simulink model "simulator_prototype_v2"  (R2021b)
(part 5 of 12)

tau_c = ft_4({dq1,dq2,dq3,dq4,dq5,dq6,t10,t100,t1000,t1001,t1002,t1003,t1006,t1009,t101,t1011,t1014,t1015,t1017,t1018,t1019,t1020,t1021,t1023,t1024,t1025,t1028,t1029,t103,t1030,t1031,t1032,t1035,t1038,t1039,t104,t1041,t1042,t1044,t1045,t1046,t1048,t1049,t1050,t1051,t1052,t1055,t1056,t1057,t1058,t1059,t106,t1061,t1062,t1065,t1066,t1067,t107,t1070,t1071,t1072,t1073,t1074,t1075,t1076,t108,t1080,t1083,t1084,t1089,t109,t1090,t1091,t1092,t1094,t1095,t1098,t1099,t11,t110,t1100,t1102,t1103,t1104,t1105,t1106,t1107,t1108,t1109,t111,t1110,t1111,t1112,t1113,t1114,t1115,t1116,t1117,t1118,t1119,t1120,t1121,t1122,t1123,t1124,t1125,t1126,t1129,t113,t1132,t1135,t1137,t1138,t1139,t114,t1140,t1141,t1142,t1144,t1145,t1146,t1147,t1148,t1149,t115,t1150,t1154,t1158,t1159,t1162,t1165,t1166,t1167,t1170,t1174,t1176,t1177,t1178,t1179,t118,t1180,t1184,t1185,t1186,t1187,t1188,t1189,t1190,t1192,t1193,t1194,t1195,t1196,t1197,t1198,t1199,t12,t120,t1202,t1203,t1204,t1205,t1206,t1207,t1208,t1209,t121,t1210,t1212,t1213,t1214,t1217,t1218,t1219,t122,t1220,t1221,t1222,t1223,t1224,t1229,t123,t1230,t1232,t1234,t1235,t1236,t1237,t1238,t124,t1241,t1242,t1245,t1246,t1247,t1248,t125,t1251,t1252,t1253,t1254,t1255,t1256,t1259,t126,t1260,t1261,t1262,t1263,t1264,t1265,t1266,t1267,t1268,t127,t1270,t1271,t1272,t1277,t1278,t128,t1280,t1281,t1285,t1286,t1287,t1288,t1289,t1290,t1291,t1292,t1294,t1295,t1296,t1297,t1298,t1299,t13,t130,t1300,t1301,t1302,t1303,t1304,t1305,t1307,t1310,t1311,t1316,t1317,t1319,t132,t1320,t1322,t1323,t1324,t1325,t1326,t1328,t133,t1330,t1331,t1332,t1334,t1335,t1336,t1337,t1338,t134,t1342,t1343,t1344,t1345,t1348,t1349,t1350,t1351,t1352,t1353,t1354,t136,t1360,t1364,t1366,t1367,t1368,t1369,t1370,t1371,t1372,t1374,t1375,t1376,t1377,t1378,t1379,t138,t1380,t1383,t1385,t1386,t1387,t1388,t1389,t139,t1392,t1393,t1394,t1395,t1396,t1397,t1398,t1399,t14,t140,t1401,t1402,t1403,t1404,t1405,t1406,t1407,t1408,t1409,t1410,t1411,t1412,t1413,t1414,t1415,t1416,t1417,t1418,t1419,t1420,t1421,t1422,t1423,t1424,t1425,t1426,t1427,t1428,t1429,t1430,t1431,t1432,t1433,t1434,t1435,t1436,t1437,t1439,t144,t1440,t1441,t1443,t1444,t1445,t1446,t1447,t1448,t145,t1451,t1453,t1454,t1456,t1457,t1458,t1459,t1460,t1461,t1462,t1463,t1464,t1468,t1469,t1471,t1474,t1477,t1478,t1479,t148,t1480,t1481,t1482,t1483,t1484,t1485,t1486,t1487,t1488,t1489,t149,t1490,t1491,t1492,t1493,t1494,t1495,t1497,t1498,t1499,t15,t150,t1500,t1501,t1503,t1504,t1505,t1506,t1507,t1509,t151,t1510,t1512,t1513,t1514,t1515,t1516,t1517,t1518,t1519,t152,t1520,t1522,t1523,t1525,t1526,t1527,t1528,t1529,t153,t1530,t1531,t1532,t1533,t1535,t1536,t1537,t1538,t1539,t1541,t1542,t1543,t1544,t1545,t1546,t1547,t1549,t1550,t1551,t1552,t1554,t1555,t1556,t1558,t1559,t156,t1560,t1565,t1567,t1568,t1569,t157,t1570,t1571,t1572,t1574,t1575,t1576,t1577,t1578,t1579,t158,t1581,t1582,t1583,t1584,t1585,t1586,t1587,t1588,t1591,t1592,t1593,t1594,t1595,t1596,t1599,t16,t160,t1600,t1601,t1602,t1604,t1605,t1606,t1607,t1608,t1609,t161,t1613,t1614,t1615,t1616,t1618,t1619,t162,t1620,t1621,t1622,t1623,t1624,t1625,t1626,t1627,t1628,t1629,t1631,t1633,t1634,t1635,t1636,t1637,t1638,t1639,t1640,t1641,t1642,t1643,t1644,t1645,t1646,t1648,t1649,t165,t1650,t1651,t1652,t1653,t1654,t1655,t1656,t1657,t1658,t166,t1660,t167,t168,t1686,t1688,t1689,t1690,t1695,t17,t170,t1700,t1701,t1702,t171,t172,t173,t174,t175,t1750,t176,t1765,t177,t178,t1780,t1782,t1795,t1796,t1797,t1798,t18,t180,t1807,t181,t1817,t182,t185,t186,t1865,t1868,t1870,t1871,t1872,t1873,t1874,t1875,t1876,t1877,t1879,t188,t1880,t1881,t1882,t1883,t1884,t1886,t1887,t1889,t189,t1890,t1891,t1894,t1895,t1897,t1898,t1899,t19,t190,t1901,t1902,t1903,t1904,t1907,t1909,t191,t1914,t1915,t1916,t1917,t1919,t192,t1920,t1922,t1923,t1924,t1925,t1926,t1927,t1928,t1929,t1930,t1931,t1936,t1937,t1940,t1941,t1942,t1943,t1947,t1948,t1949,t195,t1950,t1951,t1952,t1953,t1956,t1958,t1959,t196,t1960,t1961,t1965,t1966,t1967,t1968,t197,t1970,t1971,t1975,t1977,t198,t1982,t1991,t1997,t20,t201,t2017,t202,t2021,t2022,t2024,t2025,t2027,t2028,t2029,t203,t2030,t2032,t2034,t2035,t2038,t2039,t204,t2043,t2044,t2045,t2049,t205,t2050,t2051,t2052,t2054,t2055,t2056,t2057,t2058,t2059,t2061,t2062,t2063,t2069,t207,t2075,t2077,t208,t2080,t2081,t2082,t2083,t2084,t2085,t2086,t2087,t2088,t2089,t209,t2090,t2091,t2092,t2093,t2096,t2097,t2098,t2099,t21,t210,t2100,t2101,t2102,t2103,t2104,t2105,t211,t2117,t2118,t2119,t212,t2120,t2121,t2122,t2123,t2124,t2131,t2138,t2139,t2140,t2147,t2149,t2150,t2151,t2152,t2153,t2154,t2155,t2156,t2157,t2158,t2159,t216,t217,t218,t219,t22,t221,t223,t225,t226,t227,t229,t2294,t2296,t2299,t230,t2300,t2302,t2303,t2305,t2306,t2308,t2309,t231,t2310,t2313,t2314,t2315,t2316,t2317,t2318,t2319,t2322,t2323,t2324,t2325,t2326,t2327,t2328,t2329,t233,t2330,t2331,t2332,t2334,t2339,t2340,t2345,t2346,t2348,t2349,t2352,t2353,t2354,t2357,t2358,t2359,t236,t2360,t2361,t2362,t2364,t2365,t2366,t2367,t237,t2374,t2378,t238,t2382,t2383,t239,t2391,t2392,t2393,t24,t240,t2402,t2404,t2405,t2406,t2407,t2409,t241,t2411,t2415,t2416,t2417,t2418,t242,t2420,t2426,t2427,t2428,t2429,t243,t2430,t2431,t2432,t2433,t2434,t2435,t2436,t2437,t2438,t2439,t2440,t2441,t2442,t2443,t2444,t2446,t2447,t2448,t2449,t245,t2451,t2452,t2453,t2454,t2455,t2456,t2457,t2459,t246,t2460,t2461,t2463,t2466,t2467,t2469,t247,t2471,t2475,t2482,t2483,t2484,t2485,t2486,t2487,t2488,t2491,t2495,t2498,t2499,t25,t2505,t251,t2512,t2513,t2515,t2529,t2541,t2544,t2546,t2551,t2560,t2567,t2568,t257,t2573,t2577,t2579,t2581,t2586,t2587,t2588,t259,t2593,t2594,t2595,t2596,t2597,t2599,t26,t260,t2600,t2601,t2603,t2605,t2606,t2607,t2608,t2609,t261,t2610,t2611,t2612,t2613,t2614,t2616,t2617,t2618,t2619,t262,t2620,t2621,t2622,t2623,t2624,t2625,t2626,t2627,t2628,t263,t2631,t2632,t2633,t2635,t2639,t264,t2640,t2641,t2642,t2643,t2645,t2646,t2647,t265,t2651,t2652,t2653,t2656,t266,t267,t268,t269,t27,t270,t271,t272,t2723,t2724,t2725,t2726,t2727,t2728,t2729,t273,t2730,t2735,t2736,t274,t2745,t2748,t2749,t275,t2750,t276,t2773,t2774,t2775,t2777,t2778,t2779,t2780,t2781,t2782,t2783,t2785,t2786,t2787,t2788,t279,t2797,t28,t280,t2800,t282,t283,t285,t2857,t2858,t2859,t286,t2860,t2865,t2867,t2868,t2872,t2879,t2883,t2884,t2886,t2887,t289,t2890,t2891,t2892,t2894,t2895,t2896,t2898,t2899,t29,t2900,t2901,t2903,t2905,t2906,t2907,t2908,t291,t2915,t2917,t2918,t2919,t292,t293,t294,t295,t2959,t296,t2960,t2965,t2966,t2967,t2968,t297,t298,t299,t30,t301,t303,t305,t306,t308,t309,t31,t310,t311,t312,t313,t314,t315,t316,t318,t319,t32,t320,t321,t322,t323,t325,t326,t328,t329,t33,t330,t331,t332,t333,t335,t336,t337,t338,t339,t34,t341,t343,t346,t348,t35,t350,t351,t352,t354,t355,t356,t358,t359,t36,t360,t361,t362,t363,t364,t365,t366,t368,t369,t370,t371,t372,t373,t377,t378,t38,t380,t381,t382,t385,t386,t387,t388,t389,t39,t390,t391,t392,t393,t396,t403,t404,t406,t407,t408,t410,t411,t412,t413,t414,t415,t419,t42,t420,t421,t422,t424,t425,t426,t427,t428,t429,t43,t430,t431,t432,t433,t434,t435,t437,t438,t439,t440,t444,t445,t446,t448,t451,t452,t455,t456,t457,t458,t459,t46,t461,t463,t464,t465,t466,t467,t468,t469,t47,t471,t472,t473,t474,t476,t477,t478,t479,t480,t483,t485,t486,t488,t489,t49,t490,t491,t493,t494,t495,t496,t497,t498,t50,t503,t504,t506,t507,t508,t509,t51,t510,t511,t512,t513,t514,t515,t516,t517,t518,t519,t52,t520,t521,t522,t523,t524,t525,t526,t527,t528,t53,t530,t531,t532,t533,t536,t537,t538,t539,t54,t540,t542,t543,t544,t545,t546,t547,t548,t550,t551,t552,t553,t554,t555,t556,t557,t559,t56,t560,t561,t562,t563,t565,t566,t568,t569,t570,t571,t572,t573,t574,t575,t576,t577,t578,t58,t580,t582,t583,t584,t585,t589,t59,t590,t591,t592,t595,t597,t599,t60,t600,t601,t605,t606,t607,t608,t609,t610,t611,t612,t614,t615,t616,t618,t619,t620,t621,t622,t623,t624,t625,t627,t628,t629,t63,t631,t634,t635,t636,t638,t64,t640,t641,t642,t643,t645,t646,t648,t649,t65,t650,t651,t652,t654,t655,t656,t657,t658,t659,t660,t662,t663,t664,t665,t666,t667,t668,t669,t67,t670,t672,t673,t674,t675,t676,t677,t678,t679,t68,t681,t682,t683,t684,t685,t686,t687,t689,t69,t691,t692,t693,t694,t696,t698,t70,t701,t702,t704,t705,t707,t708,t71,t710,t711,t712,t713,t714,t715,t716,t717,t718,t719,t720,t721,t722,t723,t724,t725,t726,t728,t73,t733,t735,t736,t738,t739,t740,t741,t742,t743,t744,t745,t746,t747,t749,t75,t750,t751,t755,t756,t757,t758,t759,t76,t762,t763,t764,t765,t766,t767,t768,t77,t770,t771,t772,t773,t774,t775,t776,t777,t778,t78,t781,t782,t783,t784,t785,t786,t787,t789,t79,t790,t791,t792,t793,t794,t796,t797,t798,t799,t8,t80,t800,t801,t802,t806,t807,t808,t809,t81,t812,t813,t816,t817,t818,t819,t82,t820,t821,t822,t823,t824,t825,t826,t827,t828,t829,t830,t831,t832,t833,t836,t837,t838,t839,t84,t840,t841,t844,t845,t846,t85,t850,t851,t852,t853,t854,t855,t856,t857,t858,t859,t860,t861,t863,t864,t865,t866,t867,t868,t869,t870,t871,t872,t874,t875,t876,t877,t878,t881,t882,t883,t885,t887,t889,t89,t890,t891,t893,t894,t895,t896,t897,t898,t9,t90,t900,t901,t902,t903,t904,t905,t906,t907,t908,t909,t91,t911,t912,t913,t914,t915,t916,t917,t918,t92,t920,t921,t923,t924,t926,t927,t929,t93,t930,t932,t933,t934,t935,t936,t937,t938,t939,t94,t940,t942,t943,t944,t945,t946,t947,t948,t950,t951,t952,t954,t956,t957,t959,t96,t960,t961,t962,t963,t964,t965,t966,t967,t969,t97,t970,t974,t975,t976,t977,t978,t981,t983,t985,t986,t987,t988,t989,t99,t990,t992,t993,t994,t995,t996,t997,t998,t999});
end
function tau_c = ft_4(ct)
dq1 = ct{1};
dq2 = ct{2};
dq3 = ct{3};
dq4 = ct{4};
dq5 = ct{5};
dq6 = ct{6};
t10 = ct{7};
t100 = ct{8};
t1000 = ct{9};
t1001 = ct{10};
t1002 = ct{11};
t1003 = ct{12};
t1006 = ct{13};
t1009 = ct{14};
t101 = ct{15};
t1011 = ct{16};
t1014 = ct{17};
t1015 = ct{18};
t1017 = ct{19};
t1018 = ct{20};
t1019 = ct{21};
t1020 = ct{22};
t1021 = ct{23};
t1023 = ct{24};
t1024 = ct{25};
t1025 = ct{26};
t1028 = ct{27};
t1029 = ct{28};
t103 = ct{29};
t1030 = ct{30};
t1031 = ct{31};
t1032 = ct{32};
t1035 = ct{33};
t1038 = ct{34};
t1039 = ct{35};
t104 = ct{36};
t1041 = ct{37};
t1042 = ct{38};
t1044 = ct{39};
t1045 = ct{40};
t1046 = ct{41};
t1048 = ct{42};
t1049 = ct{43};
t1050 = ct{44};
t1051 = ct{45};
t1052 = ct{46};
t1055 = ct{47};
t1056 = ct{48};
t1057 = ct{49};
t1058 = ct{50};
t1059 = ct{51};
t106 = ct{52};
t1061 = ct{53};
t1062 = ct{54};
t1065 = ct{55};
t1066 = ct{56};
t1067 = ct{57};
t107 = ct{58};
t1070 = ct{59};
t1071 = ct{60};
t1072 = ct{61};
t1073 = ct{62};
t1074 = ct{63};
t1075 = ct{64};
t1076 = ct{65};
t108 = ct{66};
t1080 = ct{67};
t1083 = ct{68};
t1084 = ct{69};
t1089 = ct{70};
t109 = ct{71};
t1090 = ct{72};
t1091 = ct{73};
t1092 = ct{74};
t1094 = ct{75};
t1095 = ct{76};
t1098 = ct{77};
t1099 = ct{78};
t11 = ct{79};
t110 = ct{80};
t1100 = ct{81};
t1102 = ct{82};
t1103 = ct{83};
t1104 = ct{84};
t1105 = ct{85};
t1106 = ct{86};
t1107 = ct{87};
t1108 = ct{88};
t1109 = ct{89};
t111 = ct{90};
t1110 = ct{91};
t1111 = ct{92};
t1112 = ct{93};
t1113 = ct{94};
t1114 = ct{95};
t1115 = ct{96};
t1116 = ct{97};
t1117 = ct{98};
t1118 = ct{99};
t1119 = ct{100};
t1120 = ct{101};
t1121 = ct{102};
t1122 = ct{103};
t1123 = ct{104};
t1124 = ct{105};
t1125 = ct{106};
t1126 = ct{107};
t1129 = ct{108};
t113 = ct{109};
t1132 = ct{110};
t1135 = ct{111};
t1137 = ct{112};
t1138 = ct{113};
t1139 = ct{114};
t114 = ct{115};
t1140 = ct{116};
t1141 = ct{117};
t1142 = ct{118};
t1144 = ct{119};
t1145 = ct{120};
t1146 = ct{121};
t1147 = ct{122};
t1148 = ct{123};
t1149 = ct{124};
t115 = ct{125};
t1150 = ct{126};
t1154 = ct{127};
t1158 = ct{128};
t1159 = ct{129};
t1162 = ct{130};
t1165 = ct{131};
t1166 = ct{132};
t1167 = ct{133};
t1170 = ct{134};
t1174 = ct{135};
t1176 = ct{136};
t1177 = ct{137};
t1178 = ct{138};
t1179 = ct{139};
t118 = ct{140};
t1180 = ct{141};
t1184 = ct{142};
t1185 = ct{143};
t1186 = ct{144};
t1187 = ct{145};
t1188 = ct{146};
t1189 = ct{147};
t1190 = ct{148};
t1192 = ct{149};
t1193 = ct{150};
t1194 = ct{151};
t1195 = ct{152};
t1196 = ct{153};
t1197 = ct{154};
t1198 = ct{155};
t1199 = ct{156};
t12 = ct{157};
t120 = ct{158};
t1202 = ct{159};
t1203 = ct{160};
t1204 = ct{161};
t1205 = ct{162};
t1206 = ct{163};
t1207 = ct{164};
t1208 = ct{165};
t1209 = ct{166};
t121 = ct{167};
t1210 = ct{168};
t1212 = ct{169};
t1213 = ct{170};
t1214 = ct{171};
t1217 = ct{172};
t1218 = ct{173};
t1219 = ct{174};
t122 = ct{175};
t1220 = ct{176};
t1221 = ct{177};
t1222 = ct{178};
t1223 = ct{179};
t1224 = ct{180};
t1229 = ct{181};
t123 = ct{182};
t1230 = ct{183};
t1232 = ct{184};
t1234 = ct{185};
t1235 = ct{186};
t1236 = ct{187};
t1237 = ct{188};
t1238 = ct{189};
t124 = ct{190};
t1241 = ct{191};
t1242 = ct{192};
t1245 = ct{193};
t1246 = ct{194};
t1247 = ct{195};
t1248 = ct{196};
t125 = ct{197};
t1251 = ct{198};
t1252 = ct{199};
t1253 = ct{200};
t1254 = ct{201};
t1255 = ct{202};
t1256 = ct{203};
t1259 = ct{204};
t126 = ct{205};
t1260 = ct{206};
t1261 = ct{207};
t1262 = ct{208};
t1263 = ct{209};
t1264 = ct{210};
t1265 = ct{211};
t1266 = ct{212};
t1267 = ct{213};
t1268 = ct{214};
t127 = ct{215};
t1270 = ct{216};
t1271 = ct{217};
t1272 = ct{218};
t1277 = ct{219};
t1278 = ct{220};
t128 = ct{221};
t1280 = ct{222};
t1281 = ct{223};
t1285 = ct{224};
t1286 = ct{225};
t1287 = ct{226};
t1288 = ct{227};
t1289 = ct{228};
t1290 = ct{229};
t1291 = ct{230};
t1292 = ct{231};
t1294 = ct{232};
t1295 = ct{233};
t1296 = ct{234};
t1297 = ct{235};
t1298 = ct{236};
t1299 = ct{237};
t13 = ct{238};
t130 = ct{239};
t1300 = ct{240};
t1301 = ct{241};
t1302 = ct{242};
t1303 = ct{243};
t1304 = ct{244};
t1305 = ct{245};
t1307 = ct{246};
t1310 = ct{247};
t1311 = ct{248};
t1316 = ct{249};
t1317 = ct{250};
t1319 = ct{251};
t132 = ct{252};
t1320 = ct{253};
t1322 = ct{254};
t1323 = ct{255};
t1324 = ct{256};
t1325 = ct{257};
t1326 = ct{258};
t1328 = ct{259};
t133 = ct{260};
t1330 = ct{261};
t1331 = ct{262};
t1332 = ct{263};
t1334 = ct{264};
t1335 = ct{265};
t1336 = ct{266};
t1337 = ct{267};
t1338 = ct{268};
t134 = ct{269};
t1342 = ct{270};
t1343 = ct{271};
t1344 = ct{272};
t1345 = ct{273};
t1348 = ct{274};
t1349 = ct{275};
t1350 = ct{276};
t1351 = ct{277};
t1352 = ct{278};
t1353 = ct{279};
t1354 = ct{280};
t136 = ct{281};
t1360 = ct{282};
t1364 = ct{283};
t1366 = ct{284};
t1367 = ct{285};
t1368 = ct{286};
t1369 = ct{287};
t1370 = ct{288};
t1371 = ct{289};
t1372 = ct{290};
t1374 = ct{291};
t1375 = ct{292};
t1376 = ct{293};
t1377 = ct{294};
t1378 = ct{295};
t1379 = ct{296};
t138 = ct{297};
t1380 = ct{298};
t1383 = ct{299};
t1385 = ct{300};
t1386 = ct{301};
t1387 = ct{302};
t1388 = ct{303};
t1389 = ct{304};
t139 = ct{305};
t1392 = ct{306};
t1393 = ct{307};
t1394 = ct{308};
t1395 = ct{309};
t1396 = ct{310};
t1397 = ct{311};
t1398 = ct{312};
t1399 = ct{313};
t14 = ct{314};
t140 = ct{315};
t1401 = ct{316};
t1402 = ct{317};
t1403 = ct{318};
t1404 = ct{319};
t1405 = ct{320};
t1406 = ct{321};
t1407 = ct{322};
t1408 = ct{323};
t1409 = ct{324};
t1410 = ct{325};
t1411 = ct{326};
t1412 = ct{327};
t1413 = ct{328};
t1414 = ct{329};
t1415 = ct{330};
t1416 = ct{331};
t1417 = ct{332};
t1418 = ct{333};
t1419 = ct{334};
t1420 = ct{335};
t1421 = ct{336};
t1422 = ct{337};
t1423 = ct{338};
t1424 = ct{339};
t1425 = ct{340};
t1426 = ct{341};
t1427 = ct{342};
t1428 = ct{343};
t1429 = ct{344};
t1430 = ct{345};
t1431 = ct{346};
t1432 = ct{347};
t1433 = ct{348};
t1434 = ct{349};
t1435 = ct{350};
t1436 = ct{351};
t1437 = ct{352};
t1439 = ct{353};
t144 = ct{354};
t1440 = ct{355};
t1441 = ct{356};
t1443 = ct{357};
t1444 = ct{358};
t1445 = ct{359};
t1446 = ct{360};
t1447 = ct{361};
t1448 = ct{362};
t145 = ct{363};
t1451 = ct{364};
t1453 = ct{365};
t1454 = ct{366};
t1456 = ct{367};
t1457 = ct{368};
t1458 = ct{369};
t1459 = ct{370};
t1460 = ct{371};
t1461 = ct{372};
t1462 = ct{373};
t1463 = ct{374};
t1464 = ct{375};
t1468 = ct{376};
t1469 = ct{377};
t1471 = ct{378};
t1474 = ct{379};
t1477 = ct{380};
t1478 = ct{381};
t1479 = ct{382};
t148 = ct{383};
t1480 = ct{384};
t1481 = ct{385};
t1482 = ct{386};
t1483 = ct{387};
t1484 = ct{388};
t1485 = ct{389};
t1486 = ct{390};
t1487 = ct{391};
t1488 = ct{392};
t1489 = ct{393};
t149 = ct{394};
t1490 = ct{395};
t1491 = ct{396};
t1492 = ct{397};
t1493 = ct{398};
t1494 = ct{399};
t1495 = ct{400};
t1497 = ct{401};
t1498 = ct{402};
t1499 = ct{403};
t15 = ct{404};
t150 = ct{405};
t1500 = ct{406};
t1501 = ct{407};
t1503 = ct{408};
t1504 = ct{409};
t1505 = ct{410};
t1506 = ct{411};
t1507 = ct{412};
t1509 = ct{413};
t151 = ct{414};
t1510 = ct{415};
t1512 = ct{416};
t1513 = ct{417};
t1514 = ct{418};
t1515 = ct{419};
t1516 = ct{420};
t1517 = ct{421};
t1518 = ct{422};
t1519 = ct{423};
t152 = ct{424};
t1520 = ct{425};
t1522 = ct{426};
t1523 = ct{427};
t1525 = ct{428};
t1526 = ct{429};
t1527 = ct{430};
t1528 = ct{431};
t1529 = ct{432};
t153 = ct{433};
t1530 = ct{434};
t1531 = ct{435};
t1532 = ct{436};
t1533 = ct{437};
t1535 = ct{438};
t1536 = ct{439};
t1537 = ct{440};
t1538 = ct{441};
t1539 = ct{442};
t1541 = ct{443};
t1542 = ct{444};
t1543 = ct{445};
t1544 = ct{446};
t1545 = ct{447};
t1546 = ct{448};
t1547 = ct{449};
t1549 = ct{450};
t1550 = ct{451};
t1551 = ct{452};
t1552 = ct{453};
t1554 = ct{454};
t1555 = ct{455};
t1556 = ct{456};
t1558 = ct{457};
t1559 = ct{458};
t156 = ct{459};
t1560 = ct{460};
t1565 = ct{461};
t1567 = ct{462};
t1568 = ct{463};
t1569 = ct{464};
t157 = ct{465};
t1570 = ct{466};
t1571 = ct{467};
t1572 = ct{468};
t1574 = ct{469};
t1575 = ct{470};
t1576 = ct{471};
t1577 = ct{472};
t1578 = ct{473};
t1579 = ct{474};
t158 = ct{475};
t1581 = ct{476};
t1582 = ct{477};
t1583 = ct{478};
t1584 = ct{479};
t1585 = ct{480};
t1586 = ct{481};
t1587 = ct{482};
t1588 = ct{483};
t1591 = ct{484};
t1592 = ct{485};
t1593 = ct{486};
t1594 = ct{487};
t1595 = ct{488};
t1596 = ct{489};
t1599 = ct{490};
t16 = ct{491};
t160 = ct{492};
t1600 = ct{493};
t1601 = ct{494};
t1602 = ct{495};
t1604 = ct{496};
t1605 = ct{497};
t1606 = ct{498};
t1607 = ct{499};
t1608 = ct{500};
t1609 = ct{501};
t161 = ct{502};
t1613 = ct{503};
t1614 = ct{504};
t1615 = ct{505};
t1616 = ct{506};
t1618 = ct{507};
t1619 = ct{508};
t162 = ct{509};
t1620 = ct{510};
t1621 = ct{511};
t1622 = ct{512};
t1623 = ct{513};
t1624 = ct{514};
t1625 = ct{515};
t1626 = ct{516};
t1627 = ct{517};
t1628 = ct{518};
t1629 = ct{519};
t1631 = ct{520};
t1633 = ct{521};
t1634 = ct{522};
t1635 = ct{523};
t1636 = ct{524};
t1637 = ct{525};
t1638 = ct{526};
t1639 = ct{527};
t1640 = ct{528};
t1641 = ct{529};
t1642 = ct{530};
t1643 = ct{531};
t1644 = ct{532};
t1645 = ct{533};
t1646 = ct{534};
t1648 = ct{535};
t1649 = ct{536};
t165 = ct{537};
t1650 = ct{538};
t1651 = ct{539};
t1652 = ct{540};
t1653 = ct{541};
t1654 = ct{542};
t1655 = ct{543};
t1656 = ct{544};
t1657 = ct{545};
t1658 = ct{546};
t166 = ct{547};
t1660 = ct{548};
t167 = ct{549};
t168 = ct{550};
t1686 = ct{551};
t1688 = ct{552};
t1689 = ct{553};
t1690 = ct{554};
t1695 = ct{555};
t17 = ct{556};
t170 = ct{557};
t1700 = ct{558};
t1701 = ct{559};
t1702 = ct{560};
t171 = ct{561};
t172 = ct{562};
t173 = ct{563};
t174 = ct{564};
t175 = ct{565};
t1750 = ct{566};
t176 = ct{567};
t1765 = ct{568};
t177 = ct{569};
t178 = ct{570};
t1780 = ct{571};
t1782 = ct{572};
t1795 = ct{573};
t1796 = ct{574};
t1797 = ct{575};
t1798 = ct{576};
t18 = ct{577};
t180 = ct{578};
t1807 = ct{579};
t181 = ct{580};
t1817 = ct{581};
t182 = ct{582};
t185 = ct{583};
t186 = ct{584};
t1865 = ct{585};
t1868 = ct{586};
t1870 = ct{587};
t1871 = ct{588};
t1872 = ct{589};
t1873 = ct{590};
t1874 = ct{591};
t1875 = ct{592};
t1876 = ct{593};
t1877 = ct{594};
t1879 = ct{595};
t188 = ct{596};
t1880 = ct{597};
t1881 = ct{598};
t1882 = ct{599};
t1883 = ct{600};
t1884 = ct{601};
t1886 = ct{602};
t1887 = ct{603};
t1889 = ct{604};
t189 = ct{605};
t1890 = ct{606};
t1891 = ct{607};
t1894 = ct{608};
t1895 = ct{609};
t1897 = ct{610};
t1898 = ct{611};
t1899 = ct{612};
t19 = ct{613};
t190 = ct{614};
t1901 = ct{615};
t1902 = ct{616};
t1903 = ct{617};
t1904 = ct{618};
t1907 = ct{619};
t1909 = ct{620};
t191 = ct{621};
t1914 = ct{622};
t1915 = ct{623};
t1916 = ct{624};
t1917 = ct{625};
t1919 = ct{626};
t192 = ct{627};
t1920 = ct{628};
t1922 = ct{629};
t1923 = ct{630};
t1924 = ct{631};
t1925 = ct{632};
t1926 = ct{633};
t1927 = ct{634};
t1928 = ct{635};
t1929 = ct{636};
t1930 = ct{637};
t1931 = ct{638};
t1936 = ct{639};
t1937 = ct{640};
t1940 = ct{641};
t1941 = ct{642};
t1942 = ct{643};
t1943 = ct{644};
t1947 = ct{645};
t1948 = ct{646};
t1949 = ct{647};
t195 = ct{648};
t1950 = ct{649};
t1951 = ct{650};
t1952 = ct{651};
t1953 = ct{652};
t1956 = ct{653};
t1958 = ct{654};
t1959 = ct{655};
t196 = ct{656};
t1960 = ct{657};
t1961 = ct{658};
t1965 = ct{659};
t1966 = ct{660};
t1967 = ct{661};
t1968 = ct{662};
t197 = ct{663};
t1970 = ct{664};
t1971 = ct{665};
t1975 = ct{666};
t1977 = ct{667};
t198 = ct{668};
t1982 = ct{669};
t1991 = ct{670};
t1997 = ct{671};
t20 = ct{672};
t201 = ct{673};
t2017 = ct{674};
t202 = ct{675};
t2021 = ct{676};
t2022 = ct{677};
t2024 = ct{678};
t2025 = ct{679};
t2027 = ct{680};
t2028 = ct{681};
t2029 = ct{682};
t203 = ct{683};
t2030 = ct{684};
t2032 = ct{685};
t2034 = ct{686};
t2035 = ct{687};
t2038 = ct{688};
t2039 = ct{689};
t204 = ct{690};
t2043 = ct{691};
t2044 = ct{692};
t2045 = ct{693};
t2049 = ct{694};
t205 = ct{695};
t2050 = ct{696};
t2051 = ct{697};
t2052 = ct{698};
t2054 = ct{699};
t2055 = ct{700};
t2056 = ct{701};
t2057 = ct{702};
t2058 = ct{703};
t2059 = ct{704};
t2061 = ct{705};
t2062 = ct{706};
t2063 = ct{707};
t2069 = ct{708};
t207 = ct{709};
t2075 = ct{710};
t2077 = ct{711};
t208 = ct{712};
t2080 = ct{713};
t2081 = ct{714};
t2082 = ct{715};
t2083 = ct{716};
t2084 = ct{717};
t2085 = ct{718};
t2086 = ct{719};
t2087 = ct{720};
t2088 = ct{721};
t2089 = ct{722};
t209 = ct{723};
t2090 = ct{724};
t2091 = ct{725};
t2092 = ct{726};
t2093 = ct{727};
t2096 = ct{728};
t2097 = ct{729};
t2098 = ct{730};
t2099 = ct{731};
t21 = ct{732};
t210 = ct{733};
t2100 = ct{734};
t2101 = ct{735};
t2102 = ct{736};
t2103 = ct{737};
t2104 = ct{738};
t2105 = ct{739};
t211 = ct{740};
t2117 = ct{741};
t2118 = ct{742};
t2119 = ct{743};
t212 = ct{744};
t2120 = ct{745};
t2121 = ct{746};
t2122 = ct{747};
t2123 = ct{748};
t2124 = ct{749};
t2131 = ct{750};
t2138 = ct{751};
t2139 = ct{752};
t2140 = ct{753};
t2147 = ct{754};
t2149 = ct{755};
t2150 = ct{756};
t2151 = ct{757};
t2152 = ct{758};
t2153 = ct{759};
t2154 = ct{760};
t2155 = ct{761};
t2156 = ct{762};
t2157 = ct{763};
t2158 = ct{764};
t2159 = ct{765};
t216 = ct{766};
t217 = ct{767};
t218 = ct{768};
t219 = ct{769};
t22 = ct{770};
t221 = ct{771};
t223 = ct{772};
t225 = ct{773};
t226 = ct{774};
t227 = ct{775};
t229 = ct{776};
t2294 = ct{777};
t2296 = ct{778};
t2299 = ct{779};
t230 = ct{780};
t2300 = ct{781};
t2302 = ct{782};
t2303 = ct{783};
t2305 = ct{784};
t2306 = ct{785};
t2308 = ct{786};
t2309 = ct{787};
t231 = ct{788};
t2310 = ct{789};
t2313 = ct{790};
t2314 = ct{791};
t2315 = ct{792};
t2316 = ct{793};
t2317 = ct{794};
t2318 = ct{795};
t2319 = ct{796};
t2322 = ct{797};
t2323 = ct{798};
t2324 = ct{799};
t2325 = ct{800};
t2326 = ct{801};
t2327 = ct{802};
t2328 = ct{803};
t2329 = ct{804};
t233 = ct{805};
t2330 = ct{806};
t2331 = ct{807};
t2332 = ct{808};
t2334 = ct{809};
t2339 = ct{810};
t2340 = ct{811};
t2345 = ct{812};
t2346 = ct{813};
t2348 = ct{814};
t2349 = ct{815};
t2352 = ct{816};
t2353 = ct{817};
t2354 = ct{818};
t2357 = ct{819};
t2358 = ct{820};
t2359 = ct{821};
t236 = ct{822};
t2360 = ct{823};
t2361 = ct{824};
t2362 = ct{825};
t2364 = ct{826};
t2365 = ct{827};
t2366 = ct{828};
t2367 = ct{829};
t237 = ct{830};
t2374 = ct{831};
t2378 = ct{832};
t238 = ct{833};
t2382 = ct{834};
t2383 = ct{835};
t239 = ct{836};
t2391 = ct{837};
t2392 = ct{838};
t2393 = ct{839};
t24 = ct{840};
t240 = ct{841};
t2402 = ct{842};
t2404 = ct{843};
t2405 = ct{844};
t2406 = ct{845};
t2407 = ct{846};
t2409 = ct{847};
t241 = ct{848};
t2411 = ct{849};
t2415 = ct{850};
t2416 = ct{851};
t2417 = ct{852};
t2418 = ct{853};
t242 = ct{854};
t2420 = ct{855};
t2426 = ct{856};
t2427 = ct{857};
t2428 = ct{858};
t2429 = ct{859};
t243 = ct{860};
t2430 = ct{861};
t2431 = ct{862};
t2432 = ct{863};
t2433 = ct{864};
t2434 = ct{865};
t2435 = ct{866};
t2436 = ct{867};
t2437 = ct{868};
t2438 = ct{869};
t2439 = ct{870};
t2440 = ct{871};
t2441 = ct{872};
t2442 = ct{873};
t2443 = ct{874};
t2444 = ct{875};
t2446 = ct{876};
t2447 = ct{877};
t2448 = ct{878};
t2449 = ct{879};
t245 = ct{880};
t2451 = ct{881};
t2452 = ct{882};
t2453 = ct{883};
t2454 = ct{884};
t2455 = ct{885};
t2456 = ct{886};
t2457 = ct{887};
t2459 = ct{888};
t246 = ct{889};
t2460 = ct{890};
t2461 = ct{891};
t2463 = ct{892};
t2466 = ct{893};
t2467 = ct{894};
t2469 = ct{895};
t247 = ct{896};
t2471 = ct{897};
t2475 = ct{898};
t2482 = ct{899};
t2483 = ct{900};
t2484 = ct{901};
t2485 = ct{902};
t2486 = ct{903};
t2487 = ct{904};
t2488 = ct{905};
t2491 = ct{906};
t2495 = ct{907};
t2498 = ct{908};
t2499 = ct{909};
t25 = ct{910};
t2505 = ct{911};
t251 = ct{912};
t2512 = ct{913};
t2513 = ct{914};
t2515 = ct{915};
t2529 = ct{916};
t2541 = ct{917};
t2544 = ct{918};
t2546 = ct{919};
t2551 = ct{920};
t2560 = ct{921};
t2567 = ct{922};
t2568 = ct{923};
t257 = ct{924};
t2573 = ct{925};
t2577 = ct{926};
t2579 = ct{927};
t2581 = ct{928};
t2586 = ct{929};
t2587 = ct{930};
t2588 = ct{931};
t259 = ct{932};
t2593 = ct{933};
t2594 = ct{934};
t2595 = ct{935};
t2596 = ct{936};
t2597 = ct{937};
t2599 = ct{938};
t26 = ct{939};
t260 = ct{940};
t2600 = ct{941};
t2601 = ct{942};
t2603 = ct{943};
t2605 = ct{944};
t2606 = ct{945};
t2607 = ct{946};
t2608 = ct{947};
t2609 = ct{948};
t261 = ct{949};
t2610 = ct{950};
t2611 = ct{951};
t2612 = ct{952};
t2613 = ct{953};
t2614 = ct{954};
t2616 = ct{955};
t2617 = ct{956};
t2618 = ct{957};
t2619 = ct{958};
t262 = ct{959};
t2620 = ct{960};
t2621 = ct{961};
t2622 = ct{962};
t2623 = ct{963};
t2624 = ct{964};
t2625 = ct{965};
t2626 = ct{966};
t2627 = ct{967};
t2628 = ct{968};
t263 = ct{969};
t2631 = ct{970};
t2632 = ct{971};
t2633 = ct{972};
t2635 = ct{973};
t2639 = ct{974};
t264 = ct{975};
t2640 = ct{976};
t2641 = ct{977};
t2642 = ct{978};
t2643 = ct{979};
t2645 = ct{980};
t2646 = ct{981};
t2647 = ct{982};
t265 = ct{983};
t2651 = ct{984};
t2652 = ct{985};
t2653 = ct{986};
t2656 = ct{987};
t266 = ct{988};
t267 = ct{989};
t268 = ct{990};
t269 = ct{991};
t27 = ct{992};
t270 = ct{993};
t271 = ct{994};
t272 = ct{995};
t2723 = ct{996};
t2724 = ct{997};
t2725 = ct{998};
t2726 = ct{999};
t2727 = ct{1000};
t2728 = ct{1001};
t2729 = ct{1002};
t273 = ct{1003};
t2730 = ct{1004};
t2735 = ct{1005};
t2736 = ct{1006};
t274 = ct{1007};
t2745 = ct{1008};
t2748 = ct{1009};
t2749 = ct{1010};
t275 = ct{1011};
t2750 = ct{1012};
t276 = ct{1013};
t2773 = ct{1014};
t2774 = ct{1015};
t2775 = ct{1016};
t2777 = ct{1017};
t2778 = ct{1018};
t2779 = ct{1019};
t2780 = ct{1020};
t2781 = ct{1021};
t2782 = ct{1022};
t2783 = ct{1023};
t2785 = ct{1024};
t2786 = ct{1025};
t2787 = ct{1026};
t2788 = ct{1027};
t279 = ct{1028};
t2797 = ct{1029};
t28 = ct{1030};
t280 = ct{1031};
t2800 = ct{1032};
t282 = ct{1033};
t283 = ct{1034};
t285 = ct{1035};
t2857 = ct{1036};
t2858 = ct{1037};
t2859 = ct{1038};
t286 = ct{1039};
t2860 = ct{1040};
t2865 = ct{1041};
t2867 = ct{1042};
t2868 = ct{1043};
t2872 = ct{1044};
t2879 = ct{1045};
t2883 = ct{1046};
t2884 = ct{1047};
t2886 = ct{1048};
t2887 = ct{1049};
t289 = ct{1050};
t2890 = ct{1051};
t2891 = ct{1052};
t2892 = ct{1053};
t2894 = ct{1054};
t2895 = ct{1055};
t2896 = ct{1056};
t2898 = ct{1057};
t2899 = ct{1058};
t29 = ct{1059};
t2900 = ct{1060};
t2901 = ct{1061};
t2903 = ct{1062};
t2905 = ct{1063};
t2906 = ct{1064};
t2907 = ct{1065};
t2908 = ct{1066};
t291 = ct{1067};
t2915 = ct{1068};
t2917 = ct{1069};
t2918 = ct{1070};
t2919 = ct{1071};
t292 = ct{1072};
t293 = ct{1073};
t294 = ct{1074};
t295 = ct{1075};
t2959 = ct{1076};
t296 = ct{1077};
t2960 = ct{1078};
t2965 = ct{1079};
t2966 = ct{1080};
t2967 = ct{1081};
t2968 = ct{1082};
t297 = ct{1083};
t298 = ct{1084};
t299 = ct{1085};
t30 = ct{1086};
t301 = ct{1087};
t303 = ct{1088};
t305 = ct{1089};
t306 = ct{1090};
t308 = ct{1091};
t309 = ct{1092};
t31 = ct{1093};
t310 = ct{1094};
t311 = ct{1095};
t312 = ct{1096};
t313 = ct{1097};
t314 = ct{1098};
t315 = ct{1099};
t316 = ct{1100};
t318 = ct{1101};
t319 = ct{1102};
t32 = ct{1103};
t320 = ct{1104};
t321 = ct{1105};
t322 = ct{1106};
t323 = ct{1107};
t325 = ct{1108};
t326 = ct{1109};
t328 = ct{1110};
t329 = ct{1111};
t33 = ct{1112};
t330 = ct{1113};
t331 = ct{1114};
t332 = ct{1115};
t333 = ct{1116};
t335 = ct{1117};
t336 = ct{1118};
t337 = ct{1119};
t338 = ct{1120};
t339 = ct{1121};
t34 = ct{1122};
t341 = ct{1123};
t343 = ct{1124};
t346 = ct{1125};
t348 = ct{1126};
t35 = ct{1127};
t350 = ct{1128};
t351 = ct{1129};
t352 = ct{1130};
t354 = ct{1131};
t355 = ct{1132};
t356 = ct{1133};
t358 = ct{1134};
t359 = ct{1135};
t36 = ct{1136};
t360 = ct{1137};
t361 = ct{1138};
t362 = ct{1139};
t363 = ct{1140};
t364 = ct{1141};
t365 = ct{1142};
t366 = ct{1143};
t368 = ct{1144};
t369 = ct{1145};
t370 = ct{1146};
t371 = ct{1147};
t372 = ct{1148};
t373 = ct{1149};
t377 = ct{1150};
t378 = ct{1151};
t38 = ct{1152};
t380 = ct{1153};
t381 = ct{1154};
t382 = ct{1155};
t385 = ct{1156};
t386 = ct{1157};
t387 = ct{1158};
t388 = ct{1159};
t389 = ct{1160};
t39 = ct{1161};
t390 = ct{1162};
t391 = ct{1163};
t392 = ct{1164};
t393 = ct{1165};
t396 = ct{1166};
t403 = ct{1167};
t404 = ct{1168};
t406 = ct{1169};
t407 = ct{1170};
t408 = ct{1171};
t410 = ct{1172};
t411 = ct{1173};
t412 = ct{1174};
t413 = ct{1175};
t414 = ct{1176};
t415 = ct{1177};
t419 = ct{1178};
t42 = ct{1179};
t420 = ct{1180};
t421 = ct{1181};
t422 = ct{1182};
t424 = ct{1183};
t425 = ct{1184};
t426 = ct{1185};
t427 = ct{1186};
t428 = ct{1187};
t429 = ct{1188};
t43 = ct{1189};
t430 = ct{1190};
t431 = ct{1191};
t432 = ct{1192};
t433 = ct{1193};
t434 = ct{1194};
t435 = ct{1195};
t437 = ct{1196};
t438 = ct{1197};
t439 = ct{1198};
t440 = ct{1199};
t444 = ct{1200};
t445 = ct{1201};
t446 = ct{1202};
t448 = ct{1203};
t451 = ct{1204};
t452 = ct{1205};
t455 = ct{1206};
t456 = ct{1207};
t457 = ct{1208};
t458 = ct{1209};
t459 = ct{1210};
t46 = ct{1211};
t461 = ct{1212};
t463 = ct{1213};
t464 = ct{1214};
t465 = ct{1215};
t466 = ct{1216};
t467 = ct{1217};
t468 = ct{1218};
t469 = ct{1219};
t47 = ct{1220};
t471 = ct{1221};
t472 = ct{1222};
t473 = ct{1223};
t474 = ct{1224};
t476 = ct{1225};
t477 = ct{1226};
t478 = ct{1227};
t479 = ct{1228};
t480 = ct{1229};
t483 = ct{1230};
t485 = ct{1231};
t486 = ct{1232};
t488 = ct{1233};
t489 = ct{1234};
t49 = ct{1235};
t490 = ct{1236};
t491 = ct{1237};
t493 = ct{1238};
t494 = ct{1239};
t495 = ct{1240};
t496 = ct{1241};
t497 = ct{1242};
t498 = ct{1243};
t50 = ct{1244};
t503 = ct{1245};
t504 = ct{1246};
t506 = ct{1247};
t507 = ct{1248};
t508 = ct{1249};
t509 = ct{1250};
t51 = ct{1251};
t510 = ct{1252};
t511 = ct{1253};
t512 = ct{1254};
t513 = ct{1255};
t514 = ct{1256};
t515 = ct{1257};
t516 = ct{1258};
t517 = ct{1259};
t518 = ct{1260};
t519 = ct{1261};
t52 = ct{1262};
t520 = ct{1263};
t521 = ct{1264};
t522 = ct{1265};
t523 = ct{1266};
t524 = ct{1267};
t525 = ct{1268};
t526 = ct{1269};
t527 = ct{1270};
t528 = ct{1271};
t53 = ct{1272};
t530 = ct{1273};
t531 = ct{1274};
t532 = ct{1275};
t533 = ct{1276};
t536 = ct{1277};
t537 = ct{1278};
t538 = ct{1279};
t539 = ct{1280};
t54 = ct{1281};
t540 = ct{1282};
t542 = ct{1283};
t543 = ct{1284};
t544 = ct{1285};
t545 = ct{1286};
t546 = ct{1287};
t547 = ct{1288};
t548 = ct{1289};
t550 = ct{1290};
t551 = ct{1291};
t552 = ct{1292};
t553 = ct{1293};
t554 = ct{1294};
t555 = ct{1295};
t556 = ct{1296};
t557 = ct{1297};
t559 = ct{1298};
t56 = ct{1299};
t560 = ct{1300};
t561 = ct{1301};
t562 = ct{1302};
t563 = ct{1303};
t565 = ct{1304};
t566 = ct{1305};
t568 = ct{1306};
t569 = ct{1307};
t570 = ct{1308};
t571 = ct{1309};
t572 = ct{1310};
t573 = ct{1311};
t574 = ct{1312};
t575 = ct{1313};
t576 = ct{1314};
t577 = ct{1315};
t578 = ct{1316};
t58 = ct{1317};
t580 = ct{1318};
t582 = ct{1319};
t583 = ct{1320};
t584 = ct{1321};
t585 = ct{1322};
t589 = ct{1323};
t59 = ct{1324};
t590 = ct{1325};
t591 = ct{1326};
t592 = ct{1327};
t595 = ct{1328};
t597 = ct{1329};
t599 = ct{1330};
t60 = ct{1331};
t600 = ct{1332};
t601 = ct{1333};
t605 = ct{1334};
t606 = ct{1335};
t607 = ct{1336};
t608 = ct{1337};
t609 = ct{1338};
t610 = ct{1339};
t611 = ct{1340};
t612 = ct{1341};
t614 = ct{1342};
t615 = ct{1343};
t616 = ct{1344};
t618 = ct{1345};
t619 = ct{1346};
t620 = ct{1347};
t621 = ct{1348};
t622 = ct{1349};
t623 = ct{1350};
t624 = ct{1351};
t625 = ct{1352};
t627 = ct{1353};
t628 = ct{1354};
t629 = ct{1355};
t63 = ct{1356};
t631 = ct{1357};
t634 = ct{1358};
t635 = ct{1359};
t636 = ct{1360};
t638 = ct{1361};
t64 = ct{1362};
t640 = ct{1363};
t641 = ct{1364};
t642 = ct{1365};
t643 = ct{1366};
t645 = ct{1367};
t646 = ct{1368};
t648 = ct{1369};
t649 = ct{1370};
t65 = ct{1371};
t650 = ct{1372};
t651 = ct{1373};
t652 = ct{1374};
t654 = ct{1375};
t655 = ct{1376};
t656 = ct{1377};
t657 = ct{1378};
t658 = ct{1379};
t659 = ct{1380};
t660 = ct{1381};
t662 = ct{1382};
t663 = ct{1383};
t664 = ct{1384};
t665 = ct{1385};
t666 = ct{1386};
t667 = ct{1387};
t668 = ct{1388};
t669 = ct{1389};
t67 = ct{1390};
t670 = ct{1391};
t672 = ct{1392};
t673 = ct{1393};
t674 = ct{1394};
t675 = ct{1395};
t676 = ct{1396};
t677 = ct{1397};
t678 = ct{1398};
t679 = ct{1399};
t68 = ct{1400};
t681 = ct{1401};
t682 = ct{1402};
t683 = ct{1403};
t684 = ct{1404};
t685 = ct{1405};
t686 = ct{1406};
t687 = ct{1407};
t689 = ct{1408};
t69 = ct{1409};
t691 = ct{1410};
t692 = ct{1411};
t693 = ct{1412};
t694 = ct{1413};
t696 = ct{1414};
t698 = ct{1415};
t70 = ct{1416};
t701 = ct{1417};
t702 = ct{1418};
t704 = ct{1419};
t705 = ct{1420};
t707 = ct{1421};
t708 = ct{1422};
t71 = ct{1423};
t710 = ct{1424};
t711 = ct{1425};
t712 = ct{1426};
t713 = ct{1427};
t714 = ct{1428};
t715 = ct{1429};
t716 = ct{1430};
t717 = ct{1431};
t718 = ct{1432};
t719 = ct{1433};
t720 = ct{1434};
t721 = ct{1435};
t722 = ct{1436};
t723 = ct{1437};
t724 = ct{1438};
t725 = ct{1439};
t726 = ct{1440};
t728 = ct{1441};
t73 = ct{1442};
t733 = ct{1443};
t735 = ct{1444};
t736 = ct{1445};
t738 = ct{1446};
t739 = ct{1447};
t740 = ct{1448};
t741 = ct{1449};
t742 = ct{1450};
t743 = ct{1451};
t744 = ct{1452};
t745 = ct{1453};
t746 = ct{1454};
t747 = ct{1455};
t749 = ct{1456};
t75 = ct{1457};
t750 = ct{1458};
t751 = ct{1459};
t755 = ct{1460};
t756 = ct{1461};
t757 = ct{1462};
t758 = ct{1463};
t759 = ct{1464};
t76 = ct{1465};
t762 = ct{1466};
t763 = ct{1467};
t764 = ct{1468};
t765 = ct{1469};
t766 = ct{1470};
t767 = ct{1471};
t768 = ct{1472};
t77 = ct{1473};
t770 = ct{1474};
t771 = ct{1475};
t772 = ct{1476};
t773 = ct{1477};
t774 = ct{1478};
t775 = ct{1479};
t776 = ct{1480};
t777 = ct{1481};
t778 = ct{1482};
t78 = ct{1483};
t781 = ct{1484};
t782 = ct{1485};
t783 = ct{1486};
t784 = ct{1487};
t785 = ct{1488};
t786 = ct{1489};
t787 = ct{1490};
t789 = ct{1491};
t79 = ct{1492};
t790 = ct{1493};
t791 = ct{1494};
t792 = ct{1495};
t793 = ct{1496};
t794 = ct{1497};
t796 = ct{1498};
t797 = ct{1499};
t798 = ct{1500};
t799 = ct{1501};
t8 = ct{1502};
t80 = ct{1503};
t800 = ct{1504};
t801 = ct{1505};
t802 = ct{1506};
t806 = ct{1507};
t807 = ct{1508};
t808 = ct{1509};
t809 = ct{1510};
t81 = ct{1511};
t812 = ct{1512};
t813 = ct{1513};
t816 = ct{1514};
t817 = ct{1515};
t818 = ct{1516};
t819 = ct{1517};
t82 = ct{1518};
t820 = ct{1519};
t821 = ct{1520};
t822 = ct{1521};
t823 = ct{1522};
t824 = ct{1523};
t825 = ct{1524};
t826 = ct{1525};
t827 = ct{1526};
t828 = ct{1527};
t829 = ct{1528};
t830 = ct{1529};
t831 = ct{1530};
t832 = ct{1531};
t833 = ct{1532};
t836 = ct{1533};
t837 = ct{1534};
t838 = ct{1535};
t839 = ct{1536};
t84 = ct{1537};
t840 = ct{1538};
t841 = ct{1539};
t844 = ct{1540};
t845 = ct{1541};
t846 = ct{1542};
t85 = ct{1543};
t850 = ct{1544};
t851 = ct{1545};
t852 = ct{1546};
t853 = ct{1547};
t854 = ct{1548};
t855 = ct{1549};
t856 = ct{1550};
t857 = ct{1551};
t858 = ct{1552};
t859 = ct{1553};
t860 = ct{1554};
t861 = ct{1555};
t863 = ct{1556};
t864 = ct{1557};
t865 = ct{1558};
t866 = ct{1559};
t867 = ct{1560};
t868 = ct{1561};
t869 = ct{1562};
t870 = ct{1563};
t871 = ct{1564};
t872 = ct{1565};
t874 = ct{1566};
t875 = ct{1567};
t876 = ct{1568};
t877 = ct{1569};
t878 = ct{1570};
t881 = ct{1571};
t882 = ct{1572};
t883 = ct{1573};
t885 = ct{1574};
t887 = ct{1575};
t889 = ct{1576};
t89 = ct{1577};
t890 = ct{1578};
t891 = ct{1579};
t893 = ct{1580};
t894 = ct{1581};
t895 = ct{1582};
t896 = ct{1583};
t897 = ct{1584};
t898 = ct{1585};
t9 = ct{1586};
t90 = ct{1587};
t900 = ct{1588};
t901 = ct{1589};
t902 = ct{1590};
t903 = ct{1591};
t904 = ct{1592};
t905 = ct{1593};
t906 = ct{1594};
t907 = ct{1595};
t908 = ct{1596};
t909 = ct{1597};
t91 = ct{1598};
t911 = ct{1599};
t912 = ct{1600};
t913 = ct{1601};
t914 = ct{1602};
t915 = ct{1603};
t916 = ct{1604};
t917 = ct{1605};
t918 = ct{1606};
t92 = ct{1607};
t920 = ct{1608};
t921 = ct{1609};
t923 = ct{1610};
t924 = ct{1611};
t926 = ct{1612};
t927 = ct{1613};
t929 = ct{1614};
t93 = ct{1615};
t930 = ct{1616};
t932 = ct{1617};
t933 = ct{1618};
t934 = ct{1619};
t935 = ct{1620};
t936 = ct{1621};
t937 = ct{1622};
t938 = ct{1623};
t939 = ct{1624};
t94 = ct{1625};
t940 = ct{1626};
t942 = ct{1627};
t943 = ct{1628};
t944 = ct{1629};
t945 = ct{1630};
t946 = ct{1631};
t947 = ct{1632};
t948 = ct{1633};
t950 = ct{1634};
t951 = ct{1635};
t952 = ct{1636};
t954 = ct{1637};
t956 = ct{1638};
t957 = ct{1639};
t959 = ct{1640};
t96 = ct{1641};
t960 = ct{1642};
t961 = ct{1643};
t962 = ct{1644};
t963 = ct{1645};
t964 = ct{1646};
t965 = ct{1647};
t966 = ct{1648};
t967 = ct{1649};
t969 = ct{1650};
t97 = ct{1651};
t970 = ct{1652};
t974 = ct{1653};
t975 = ct{1654};
t976 = ct{1655};
t977 = ct{1656};
t978 = ct{1657};
t981 = ct{1658};
t983 = ct{1659};
t985 = ct{1660};
t986 = ct{1661};
t987 = ct{1662};
t988 = ct{1663};
t989 = ct{1664};
t99 = ct{1665};
t990 = ct{1666};
t992 = ct{1667};
t993 = ct{1668};
t994 = ct{1669};
t995 = ct{1670};
t996 = ct{1671};
t997 = ct{1672};
t998 = ct{1673};
t999 = ct{1674};
t1659 = t11.*t13.*t14.*t237.*3.257046415933332e-3;
t1661 = t8.*t9.*t16.*t237.*1.485161268617439e-3;
t1662 = t8.*t11.*t14.*t237.*1.485161268617439e-3;
t1663 = t9.*t11.*t13.*t237.*1.485161268617439e-3;
t1664 = t8.*t9.*t16.*t237.*5.478347731418506e-3;
t1665 = t8.*t9.*t11.*t238.*5.478347731418506e-3;
t1666 = t8.*t11.*t14.*t237.*5.478347731418506e-3;
t1667 = t9.*t11.*t13.*t237.*5.478347731418506e-3;
t1668 = t13.*t14.*t16.*t238.*2.498039274760989e-3;
t1669 = -t1623;
t1670 = t13.*t14.*t16.*t237.*3.257046415933332e-3;
t1671 = t11.*t13.*t14.*t238.*3.257046415933332e-3;
t1672 = t8.*t9.*t16.*t238.*1.485161268617439e-3;
t1673 = t8.*t14.*t16.*t237.*1.485161268617439e-3;
t1674 = t9.*t13.*t16.*t237.*1.485161268617439e-3;
t1675 = t11.*t13.*t14.*t237.*1.485161268617439e-3;
t1676 = t8.*t14.*t16.*t237.*5.478347731418506e-3;
t1677 = t8.*t11.*t14.*t238.*5.478347731418506e-3;
t1678 = t9.*t13.*t16.*t237.*5.478347731418506e-3;
t1679 = t9.*t11.*t13.*t238.*5.478347731418506e-3;
t1680 = t11.*t13.*t14.*t237.*5.478347731418506e-3;
t1681 = t8.*t14.*t16.*t238.*1.485161268617439e-3;
t1682 = t9.*t13.*t16.*t238.*1.485161268617439e-3;
t1683 = t13.*t14.*t16.*t237.*1.485161268617439e-3;
t1684 = t13.*t14.*t16.*t237.*5.478347731418506e-3;
t1685 = t11.*t13.*t14.*t238.*5.478347731418506e-3;
t1687 = t13.*t14.*t16.*t238.*1.485161268617439e-3;
t1691 = t8.*t9.*t237.*1.509490621508912e-3;
t1692 = t8.*t9.*t238.*1.509490621508912e-3;
t1693 = t8.*t14.*t237.*1.509490621508912e-3;
t1694 = t9.*t13.*t237.*1.509490621508912e-3;
t1696 = t8.*t14.*t238.*1.509490621508912e-3;
t1697 = t9.*t13.*t238.*1.509490621508912e-3;
t1698 = t13.*t14.*t237.*1.509490621508912e-3;
t1699 = t264.*3.212809800067317e-5;
t1704 = t262.*(t46-t47).*(-7.183142969324763e-22);
t1705 = t8.*t9.*t237.*1.689683482265228e-6;
t1706 = t8.*t9.*t238.*1.689683482265228e-6;
t1707 = t8.*t14.*t237.*1.689683482265228e-6;
t1708 = t9.*t13.*t237.*1.689683482265228e-6;
t1710 = t8.*t14.*t238.*1.689683482265228e-6;
t1711 = t9.*t13.*t238.*1.689683482265228e-6;
t1712 = t13.*t14.*t237.*1.689683482265228e-6;
t1716 = t13.*t14.*t238.*1.689683482265228e-6;
t1717 = -t1638;
t1738 = -t1686;
t1739 = t27.*t262.*3.161027044821787e-5;
t1740 = t21.*t264.*3.161027044821787e-5;
t1741 = -t1688;
t1742 = -t1689;
t1743 = t27.*t264.*3.161027044821787e-5;
t1745 = t21.*t262.*6.932319085178867e-5;
t1749 = t21.*t264.*6.932319085178867e-5;
t1751 = t27.*t264.*6.932319085178867e-5;
t1752 = -t1700;
t1753 = -t1701;
t1754 = -t1702;
t1756 = t8.*t9.*t237.*2.842045365580232e-6;
t1757 = t8.*t9.*t238.*2.842045365580232e-6;
t1758 = t8.*t14.*t237.*2.842045365580232e-6;
t1759 = t9.*t13.*t237.*2.842045365580232e-6;
t1760 = t8.*t14.*t238.*2.842045365580232e-6;
t1761 = t9.*t13.*t238.*2.842045365580232e-6;
t1762 = t13.*t14.*t237.*2.842045365580232e-6;
t1764 = t13.*t14.*t238.*2.842045365580232e-6;
t1766 = t262.*9.554306323645785e-8;
t1768 = t262.*3.596333474007969e-8;
t1769 = t264.*9.554306323645785e-8;
t1770 = t8.*t9.*t237.*2.538961213904336e-3;
t1771 = t8.*t9.*t238.*2.538961213904336e-3;
t1772 = t8.*t14.*t237.*2.538961213904336e-3;
t1773 = t9.*t13.*t237.*2.538961213904336e-3;
t1775 = t8.*t14.*t238.*2.538961213904336e-3;
t1776 = t9.*t13.*t238.*2.538961213904336e-3;
t1777 = t13.*t14.*t237.*2.538961213904336e-3;
t1779 = t13.*t14.*t238.*2.538961213904336e-3;
t1786 = t20.*t50.*t240.*1.553819674864718e+37i;
t1793 = -t1780;
t1794 = -t1782;
t1799 = t20.*t22.*t50.*t240.*2.657049668350291e+37i;
t1800 = -t1798;
t1801 = t20.*t28.*t50.*t240.*4.888570919953966e+37i;
t1802 = t26.*t50.*t240.*1.720021026545681e+34i;
t1810 = t18.*t19.*t262.*3.212809800067317e-5;
t1813 = t18.*t25.*t262.*3.212809800067317e-5;
t1814 = t19.*t24.*t262.*3.212809800067317e-5;
t1816 = t24.*t25.*t262.*3.212809800067317e-5;
t1819 = t18.*t19.*t27.*t264.*(-3.161027044821787e-5);
t1820 = t18.*t19.*t264.*3.596333474007969e-8;
t1821 = t18.*t25.*t27.*t264.*(-3.161027044821787e-5);
t1822 = t19.*t24.*t27.*t264.*(-3.161027044821787e-5);
t1823 = t18.*t25.*t264.*3.596333474007969e-8;
t1824 = t19.*t24.*t264.*3.596333474007969e-8;
t1825 = t18.*t19.*t27.*t264.*5.316843277159623e-5;
t1826 = t18.*t19.*t21.*t264.*1.166015146360021e-4;
t1827 = t24.*t25.*t264.*3.596333474007969e-8;
t1828 = t18.*t25.*t27.*t264.*5.316843277159623e-5;
t1829 = t19.*t24.*t27.*t264.*5.316843277159623e-5;
t1830 = t18.*t19.*t262.*5.403941802479429e-5;
t1831 = t18.*t21.*t25.*t264.*1.166015146360021e-4;
t1832 = t19.*t21.*t24.*t264.*1.166015146360021e-4;
t1834 = t24.*t25.*t27.*t264.*5.316843277159623e-5;
t1835 = t18.*t25.*t262.*5.403941802479429e-5;
t1836 = t19.*t24.*t262.*5.403941802479429e-5;
t1837 = t21.*t24.*t25.*t264.*1.166015146360021e-4;
t1840 = t24.*t25.*t262.*5.403941802479429e-5;
t1841 = t21.*t24.*t25.*t264.*(-6.932319085178867e-5);
t1842 = t20.*t21.*t50.*t240.*4.064789595703988e+32i;
t1843 = t18.*t19.*t264.*6.049028110982645e-8;
t1844 = t18.*t25.*t264.*6.049028110982645e-8;
t1845 = t19.*t24.*t264.*6.049028110982645e-8;
t1850 = t20.*t27.*t50.*t240.*1.618908833671003e+34i;
t1851 = t24.*t25.*t264.*6.049028110982645e-8;
t1856 = t26.*t27.*t28.*t50.*t240.*2.657049668350291e+37i;
t1858 = t22.*t26.*t27.*t50.*t240.*4.888570919953966e+37i;
t1860 = (t10.*t50.*t123.*t189)./8.112963841460668e+31;
t1861 = (t15.*t50.*t123.*t189)./8.112963841460668e+31;
t1862 = t20.*t21.*t28.*t50.*t240.*1.297387533374166e+34i;
t1866 = t20.*t21.*t22.*t50.*t240.*2.386997519508773e+34i;
t1878 = -t1872;
t1885 = -t1873;
t1888 = -t1874;
t1892 = -t1877;
t1900 = -t1879;
t1905 = -t1887;
t1906 = -t1889;
t1908 = t20.*t50.*t202.*(t46-t47).*(-1.232595164407831e-32);
t1910 = -t1895;
t1911 = -t1894;
t1913 = t26.*t50.*t202.*(t46-t47).*(-1.232595164407831e-32);
t1918 = -t1897;
t1921 = -t1899;
t1932 = -t1907;
t1933 = (t20.*t50.*t202.*(t46-t47))./8.112963841460668e+31;
t1934 = -t1916;
t1935 = -t1915;
t1938 = -t1919;
t1939 = -t1922;
t1944 = -t1928;
t1945 = -t1929;
t1946 = -t1930;
t1954 = -t1940;
t1955 = -t1941;
t1957 = -t1942;
t1962 = -t1947;
t1963 = -t1949;
t1964 = -t1950;
t1969 = -t1953;
t1972 = -t1959;
t1973 = t8.*t9.*t1924;
t1974 = t8.*t14.*t1922;
t1976 = t9.*t13.*t1922;
t1978 = -t1965;
t1979 = t8.*t14.*t1924;
t1980 = t9.*t13.*t1924;
t1981 = t13.*t14.*t1922;
t1983 = t8.*t9.*t10.*t1884;
t1984 = t8.*t9.*t15.*t1882;
t1985 = t13.*t14.*t1924;
t1986 = t8.*t9.*t15.*t1884;
t1987 = t8.*t10.*t14.*t1884;
t1988 = t8.*t14.*t15.*t1882;
t1989 = t9.*t10.*t13.*t1884;
t1990 = t9.*t13.*t15.*t1882;
t1992 = -t1967;
t1993 = t8.*t14.*t15.*t1884;
t1994 = t9.*t13.*t15.*t1884;
t1995 = t10.*t13.*t14.*t1884;
t1996 = t13.*t14.*t15.*t1882;
t1998 = -t1968;
t1999 = t13.*t14.*t15.*t1884;
t2000 = t8.*t9.*t10.*t1889;
t2001 = t8.*t9.*t15.*t1889;
t2002 = t8.*t10.*t14.*t1889;
t2003 = t9.*t10.*t13.*t1889;
t2004 = -t1970;
t2005 = t8.*t9.*t15.*t1890;
t2006 = t8.*t14.*t15.*t1889;
t2007 = t9.*t13.*t15.*t1889;
t2008 = t10.*t13.*t14.*t1889;
t2009 = t8.*t14.*t15.*t1890;
t2010 = t9.*t13.*t15.*t1890;
t2011 = t13.*t14.*t15.*t1889;
t2012 = t13.*t14.*t15.*t1890;
t2013 = t8.*t9.*t1909;
t2014 = t8.*t9.*t1915;
t2015 = t8.*t14.*t1909;
t2016 = t9.*t13.*t1909;
t2018 = t8.*t14.*t1915;
t2019 = t9.*t13.*t1915;
t2020 = t13.*t14.*t1909;
t2023 = t13.*t14.*t1915;
t2026 = t8.*t9.*t1922;
t2031 = -t1975;
t2033 = -t1977;
t2036 = -t1982;
t2037 = t8.*t9.*t1940;
t2040 = t8.*t9.*t1942;
t2041 = t8.*t14.*t1940;
t2042 = t9.*t13.*t1940;
t2046 = t8.*t14.*t1942;
t2047 = t9.*t13.*t1942;
t2048 = t13.*t14.*t1940;
t2053 = t13.*t14.*t1942;
t2060 = t8.*t9.*t1936;
t2064 = t8.*t9.*t1937;
t2065 = t8.*t14.*t1936;
t2066 = t9.*t13.*t1936;
t2067 = -t2021;
t2068 = -t2022;
t2070 = t8.*t14.*t1937;
t2071 = t9.*t13.*t1937;
t2072 = t13.*t14.*t1936;
t2073 = -t2024;
t2074 = -t2025;
t2076 = t13.*t14.*t1937;
t2078 = -t2038;
t2079 = -t2039;
t2094 = -t2055;
t2095 = -t2057;
t2106 = -t2080;
t2107 = -t2088;
t2108 = -t2092;
t2109 = -t2096;
t2110 = -t2097;
t2111 = -t2098;
t2112 = -t2099;
t2113 = t963+2.61156643317655e-1;
t2114 = t964+7.38843356682345e-1;
t2115 = t986+2.61156643317655e-1;
t2116 = t988+7.38843356682345e-1;
t2126 = -t2120;
t2127 = -t2122;
t2128 = -t2123;
t2129 = -t2124;
t2130 = t264.*(t46-t47).*(-1.875105520197095e-20);
t2136 = t264.*7.0482312e-7;
t2141 = -t2131;
t2144 = t264.*(t46-t47).*(-7.825108561121397e-23);
t2145 = -t2139;
t2146 = -t2140;
t2148 = t27.*t262.*6.1855407534e-5;
t2160 = t262.*(t46-t47).*(-2.075672598245148e-23);
t2161 = t21.*t262.*1.35652563578e-4;
t2162 = t264.*(t46-t47).*7.825108561121397e-23;
t2164 = -t2152;
t2165 = -t2153;
t2166 = -t2154;
t2167 = -t2155;
t2168 = -t2158;
t2169 = -t2159;
t2174 = t18.*t19.*t21.*t262.*3.542656816146526e-5;
t2175 = t18.*t19.*t27.*t262.*3.542656816146526e-5;
t2176 = t18.*t19.*t21.*t264.*3.542656816146526e-5;
t2177 = t18.*t21.*t25.*t262.*3.542656816146526e-5;
t2178 = t19.*t21.*t24.*t262.*3.542656816146526e-5;
t2179 = t18.*t25.*t27.*t262.*3.542656816146526e-5;
t2180 = t18.*t21.*t25.*t264.*3.542656816146526e-5;
t2181 = t19.*t24.*t27.*t262.*3.542656816146526e-5;
t2182 = t19.*t21.*t24.*t264.*3.542656816146526e-5;
t2183 = t21.*t24.*t25.*t262.*3.542656816146526e-5;
t2184 = t24.*t25.*t27.*t262.*3.542656816146526e-5;
t2185 = t21.*t24.*t25.*t264.*3.542656816146526e-5;
t2186 = t18.*t19.*t262.*1.641857854109028e-5;
t2187 = t18.*t19.*t264.*1.641857854109028e-5;
t2188 = t18.*t25.*t262.*1.641857854109028e-5;
t2189 = t19.*t24.*t262.*1.641857854109028e-5;
t2190 = t18.*t25.*t264.*1.641857854109028e-5;
t2191 = t19.*t24.*t264.*1.641857854109028e-5;
t2192 = t24.*t25.*t262.*1.641857854109028e-5;
t2193 = t24.*t25.*t264.*1.641857854109028e-5;
t2194 = t18.*t25.*t264.*2.761602722751607e-5;
t2195 = t19.*t24.*t264.*2.761602722751607e-5;
t2196 = t24.*t25.*t262.*2.761602722751607e-5;
t2197 = t18.*t19.*t21.*t262.*1.615395060262503e-5;
t2198 = t24.*t25.*t264.*2.761602722751607e-5;
t2199 = t18.*t19.*t27.*t262.*1.615395060262503e-5;
t2200 = t18.*t21.*t25.*t262.*1.615395060262503e-5;
t2201 = t19.*t21.*t24.*t262.*1.615395060262503e-5;
t2203 = t18.*t19.*t262.*1.837851826825065e-8;
t2204 = t18.*t19.*t27.*t264.*1.615395060262503e-5;
t2205 = t18.*t25.*t27.*t262.*1.615395060262503e-5;
t2206 = t19.*t24.*t27.*t262.*1.615395060262503e-5;
t2207 = t21.*t24.*t25.*t262.*1.615395060262503e-5;
t2209 = t18.*t19.*t264.*1.837851826825065e-8;
t2210 = t18.*t25.*t262.*1.837851826825065e-8;
t2211 = t19.*t24.*t262.*1.837851826825065e-8;
t2212 = t18.*t19.*t21.*t262.*5.958744043986595e-5;
t2213 = t18.*t25.*t27.*t264.*1.615395060262503e-5;
t2214 = t19.*t24.*t27.*t264.*1.615395060262503e-5;
t2215 = t24.*t25.*t27.*t262.*1.615395060262503e-5;
t2217 = t18.*t25.*t264.*1.837851826825065e-8;
t2218 = t19.*t24.*t264.*1.837851826825065e-8;
t2219 = t24.*t25.*t262.*1.837851826825065e-8;
t2220 = t18.*t19.*t27.*t262.*5.958744043986595e-5;
t2221 = t18.*t19.*t21.*t264.*5.958744043986595e-5;
t2222 = t18.*t21.*t25.*t262.*5.958744043986595e-5;
t2223 = t19.*t21.*t24.*t262.*5.958744043986595e-5;
t2224 = t24.*t25.*t27.*t264.*1.615395060262503e-5;
t2225 = t24.*t25.*t264.*1.837851826825065e-8;
t2226 = t18.*t25.*t27.*t262.*5.958744043986595e-5;
t2227 = t18.*t21.*t25.*t264.*5.958744043986595e-5;
t2228 = t19.*t24.*t27.*t262.*5.958744043986595e-5;
t2229 = t19.*t21.*t24.*t264.*5.958744043986595e-5;
t2230 = t21.*t24.*t25.*t262.*5.958744043986595e-5;
t2231 = t18.*t19.*t21.*t262.*2.71709233876478e-5;
t2232 = t24.*t25.*t27.*t262.*5.958744043986595e-5;
t2233 = t21.*t24.*t25.*t264.*5.958744043986595e-5;
t2234 = t18.*t19.*t27.*t262.*2.71709233876478e-5;
t2235 = t18.*t21.*t25.*t262.*2.71709233876478e-5;
t2236 = t19.*t21.*t24.*t262.*2.71709233876478e-5;
t2238 = t18.*t19.*t27.*t264.*2.71709233876478e-5;
t2239 = t18.*t25.*t27.*t262.*2.71709233876478e-5;
t2240 = t19.*t24.*t27.*t262.*2.71709233876478e-5;
t2241 = t21.*t24.*t25.*t262.*2.71709233876478e-5;
t2244 = t18.*t25.*t27.*t264.*2.71709233876478e-5;
t2245 = t19.*t24.*t27.*t264.*2.71709233876478e-5;
t2246 = t24.*t25.*t27.*t262.*2.71709233876478e-5;
t2247 = t24.*t25.*t27.*t264.*2.71709233876478e-5;
t2249 = t18.*t19.*t262.*2.761602722751607e-5;
t2250 = t18.*t19.*t264.*2.761602722751607e-5;
t2251 = t18.*t25.*t262.*2.761602722751607e-5;
t2252 = t19.*t24.*t262.*2.761602722751607e-5;
t2253 = t18.*t19.*t262.*3.091264323687963e-8;
t2255 = t18.*t19.*t264.*3.091264323687963e-8;
t2256 = t18.*t25.*t262.*3.091264323687963e-8;
t2257 = t19.*t24.*t262.*3.091264323687963e-8;
t2259 = t18.*t25.*t264.*3.091264323687963e-8;
t2260 = t19.*t24.*t264.*3.091264323687963e-8;
t2261 = t24.*t25.*t262.*3.091264323687963e-8;
t2263 = t24.*t25.*t264.*3.091264323687963e-8;
t2290 = t10.*t50.*t123.*t189.*7.204296868834178e-35;
t2291 = t15.*t50.*t123.*t189.*7.204296868834178e-35;
t2292 = t10.*t50.*t123.*t189.*7.987216665362745e-37;
t2295 = t15.*t50.*t123.*t189.*7.987216665362745e-37;
t2297 = t238+t1454;
t2304 = t15.*t50.*t123.*t189.*7.974890713718666e-38;
t2311 = t10.*t50.*t123.*t189.*7.974890713718666e-38;
t2320 = -t2308;
t2333 = -t2318;
t2336 = -t2319;
t2341 = -t2326;
t2343 = -t2329;
t2347 = -t2330;
t2363 = t264+t1474;
t2370 = t20.*t50.*t202.*(t46-t47).*(-7.204296868834178e-35);
t2372 = t26.*t50.*t202.*(t46-t47).*(-7.204296868834178e-35);
t2375 = -t2348;
t2377 = -t2349;
t2379 = -t2352;
t2380 = -t2353;
t2384 = -t2359;
t2385 = -t2361;
t2386 = -t2362;
t2389 = -t2364;
t2394 = -t2365;
t2395 = -t2366;
t2396 = -t2367;
t2398 = t20.*t50.*t202.*(t46-t47).*(-7.987216665362745e-37);
t2401 = t26.*t50.*t202.*(t46-t47).*(-7.987216665362745e-37);
t2403 = t26.*t50.*t202.*(t46-t47).*7.204296868834178e-35;
t2408 = -t2383;
t2413 = -t2392;
t2414 = -t2393;
t2422 = -t2406;
t2425 = -t2407;
t2450 = -t2415;
t2458 = -t2420;
t2462 = t20.*t50.*t202.*(t46-t47).*(-7.974890713718666e-38);
t2464 = t26.*t50.*t202.*(t46-t47).*(-7.974890713718666e-38);
t2472 = -t2428;
t2473 = -t2429;
t2474 = -t2430;
t2476 = -t2435;
t2477 = -t2436;
t2478 = -t2437;
t2479 = -t2439;
t2480 = -t2442;
t2481 = -t2443;
t2489 = -t2454;
t2490 = -t2453;
t2492 = -t2456;
t2493 = t20.*t50.*t202.*(t46-t47).*7.974890713718666e-38;
t2494 = t26.*t50.*t202.*(t46-t47).*7.974890713718666e-38;
t2504 = -t2469;
t2508 = -t2475;
t2509 = t35.*t50.*t265.*6.209141233430105e-19i;
t2510 = t36.*t50.*t265.*6.209141233430105e-19i;
t2511 = -t2483;
t2514 = -t2486;
t2516 = -t2495;
t2518 = t188.*t201.*(t46-t47).*(-2.442490654175345e-23);
t2520 = t189.*t202.*(t46-t47).*(-2.442490654175345e-23);
t2524 = -t2513;
t2525 = t188.*t201.*(t46-t47).*2.442490654175345e-23;
t2530 = t35.*t50.*t265.*3.200438707086705e-18i;
t2532 = t36.*t50.*t265.*3.200438707086705e-18i;
t2540 = t18.*t19.*t2483;
t2542 = t18.*t19.*t2484;
t2543 = t18.*t25.*t2483;
t2545 = t19.*t24.*t2483;
t2548 = t18.*t25.*t2484;
t2549 = t19.*t24.*t2484;
t2550 = t24.*t25.*t2483;
t2552 = t18.*t19.*t2451;
t2555 = t24.*t25.*t2484;
t2556 = t18.*t19.*t2453;
t2557 = t18.*t25.*t2451;
t2558 = t19.*t24.*t2451;
t2559 = t18.*t19.*t2455;
t2561 = t18.*t25.*t2453;
t2562 = t19.*t24.*t2453;
t2563 = t24.*t25.*t2451;
t2564 = t18.*t19.*t2457;
t2565 = t18.*t25.*t2455;
t2566 = t19.*t24.*t2455;
t2569 = t24.*t25.*t2453;
t2570 = t18.*t25.*t2457;
t2571 = t19.*t24.*t2457;
t2572 = t24.*t25.*t2455;
t2574 = t24.*t25.*t2457;
t2578 = t18.*t19.*t2512;
t2580 = -t2544;
t2582 = -t2546;
t2583 = t18.*t19.*t2513;
t2584 = t18.*t25.*t2512;
t2585 = t19.*t24.*t2512;
t2589 = -t2551;
t2590 = t18.*t25.*t2513;
t2591 = t19.*t24.*t2513;
t2592 = t24.*t25.*t2512;
t2604 = t24.*t25.*t2513;
t2629 = -t2567;
t2630 = -t2568;
t2634 = -t2573;
t2644 = -t2588;
t2648 = -t2593;
t2649 = -t2594;
t2650 = -t2596;
t2654 = -t2607;
t2655 = -t2608;
t2657 = -t2609;
t2658 = -t2612;
t2659 = -t2613;
t2660 = -t2617;
t2661 = -t2625;
t2662 = -t2631;
t2665 = -t2639;
t2666 = -t2651;
t2667 = -t2652;
t2668 = -t2656;
t2699 = t850+t874;
t2718 = t855+t878;
t2731 = -t2726;
t2734 = -t2727;
t2741 = t20.*t50.*t202.*(t46-t47).*(-2.081785322124547e-36);
t2742 = t26.*t50.*t202.*(t46-t47).*(-2.081785322124547e-36);
t2753 = t20.*t50.*t202.*(t46-t47).*2.081785322124547e-36;
t2754 = t26.*t50.*t202.*(t46-t47).*2.081785322124547e-36;
t2759 = t26.*t50.*t202.*(t46-t47).*(-8.687615694748404e-39);
t2762 = -t2745;
t2769 = t20.*t50.*t202.*(t46-t47).*(-8.687615694748404e-39);
t2790 = t20.*t50.*t202.*(t46-t47).*(-2.304459510155286e-39);
t2792 = t26.*t50.*t202.*(t46-t47).*(-2.304459510155286e-39);
t2795 = -t2773;
t2796 = -t2774;
t2798 = -t2777;
t2799 = -t2778;
t2802 = -t2779;
t2803 = -t2780;
t2805 = -t2781;
t2807 = -t2782;
t2808 = -t2783;
t2811 = -t2785;
t2812 = -t2786;
t2814 = t20.*t50.*t202.*(t46-t47).*2.304459510155286e-39;
t2823 = -t2800;
t2893 = -t2860;
t2911 = -t2872;
t2914 = -t2879;
t2920 = -t2887;
t2922 = -t2891;
t2923 = -t2892;
t2925 = -t2896;
t2926 = -t2899;
t2930 = -t2906;
t2931 = -t2907;
t2933 = -t2908;
t2935 = -t2915;
t2962 = t50.*t188.*t202.*(t46-t47).*(-2.711709361697228e-39);
t2963 = -t2959;
t2964 = -t2960;
t2969 = -t2967;
t2970 = -t2968;
t3974 = t175+t210+t219+t433+t472+t477+t867+t897+t901+t1242+t1291+t1295;
t3995 = t166+t190+t403+t427+t431+t446+t851+t875+t1184+t1197+t1202+t1256;
t4260 = t52+t77+t84+t85+t122+t125+t245+t294+t296+t520+t548+t559+t560+t591+t619+t909+t952+t954;
t4325 = t145+t157+t171+t181+t390+t407+t415+t440+t840+t845+t854+t864+t1166+t1170+t1223+t1254;
t4343 = t64+t65+t96+t104+t115+t246+t247+t266+t298+t299+t532+t533+t561+t566+t595+t913+t920+t938+t946+t957;
t4705 = t51+t69+t75+t80+t81+t82+t93+t118+t233+t251+t269+t282+t289+t515+t519+t537+t545+t554+t555+t557+t570+t599+t923+t929+t939+t975+t977+3.064357668490995e+34;
tau_c = ft_5({dq1,dq2,dq3,dq4,dq5,dq6,t10,t100,t1000,t1001,t1002,t1003,t1006,t1009,t101,t1011,t1014,t1015,t1017,t1018,t1019,t1020,t1021,t1023,t1024,t1025,t1028,t1029,t103,t1030,t1031,t1032,t1035,t1038,t1039,t1041,t1042,t1044,t1045,t1046,t1048,t1049,t1050,t1051,t1052,t1055,t1056,t1057,t1058,t1059,t106,t1061,t1062,t1065,t1066,t1067,t107,t1070,t1071,t1072,t1073,t1074,t1075,t1076,t108,t1080,t1083,t1084,t1089,t109,t1090,t1091,t1092,t1094,t1095,t1098,t1099,t11,t110,t1100,t1102,t1103,t1104,t1105,t1106,t1107,t1108,t1109,t111,t1110,t1111,t1112,t1113,t1114,t1115,t1116,t1117,t1118,t1119,t1120,t1121,t1122,t1123,t1124,t1125,t1126,t1129,t113,t1132,t1135,t1137,t1138,t1139,t114,t1140,t1141,t1142,t1144,t1145,t1146,t1147,t1148,t1149,t1150,t1154,t1158,t1159,t1162,t1165,t1167,t1174,t1176,t1177,t1178,t1179,t1180,t1185,t1186,t1187,t1188,t1189,t1190,t1192,t1193,t1194,t1195,t1196,t1198,t1199,t12,t120,t1203,t1204,t1205,t1206,t1207,t1208,t1209,t121,t1210,t1212,t1213,t1214,t1217,t1218,t1219,t1220,t1221,t1222,t1224,t1229,t123,t1230,t1232,t1234,t1235,t1236,t1237,t1238,t124,t1241,t1245,t1246,t1247,t1248,t1251,t1252,t1253,t1255,t1259,t126,t1260,t1261,t1262,t1263,t1264,t1265,t1266,t1267,t1268,t127,t1270,t1271,t1272,t1277,t1278,t128,t1280,t1281,t1285,t1286,t1287,t1288,t1289,t1290,t1292,t1294,t1296,t1297,t1298,t1299,t13,t130,t1300,t1301,t1302,t1303,t1304,t1305,t1307,t1310,t1311,t1316,t1317,t1319,t132,t1320,t1322,t1323,t1324,t1325,t1326,t1328,t133,t1330,t1331,t1332,t1334,t1335,t1336,t1337,t1338,t134,t1342,t1343,t1344,t1345,t1348,t1349,t1350,t1351,t1352,t1353,t1354,t136,t1360,t1364,t1366,t1367,t1368,t1369,t1370,t1371,t1372,t1374,t1375,t1376,t1377,t1378,t1379,t138,t1380,t1383,t1385,t1386,t1387,t1388,t1389,t139,t1392,t1393,t1394,t1395,t1396,t1397,t1398,t1399,t14,t140,t1401,t1402,t1403,t1404,t1405,t1406,t1407,t1408,t1409,t1410,t1411,t1412,t1413,t1414,t1415,t1416,t1417,t1418,t1419,t1420,t1421,t1422,t1423,t1424,t1425,t1426,t1427,t1428,t1429,t1430,t1431,t1432,t1433,t1434,t1435,t1436,t1437,t1439,t144,t1440,t1441,t1443,t1444,t1445,t1446,t1447,t1448,t1451,t1453,t1456,t1457,t1458,t1459,t1460,t1461,t1462,t1463,t1464,t1468,t1469,t1471,t1477,t1478,t1479,t148,t1480,t1481,t1482,t1483,t1484,t1485,t1486,t1487,t1488,t1489,t149,t1490,t1491,t1492,t1493,t1494,t1495,t1497,t1498,t1499,t15,t150,t1500,t1501,t1503,t1504,t1505,t1506,t1507,t1509,t151,t1510,t1512,t1513,t1514,t1515,t1516,t1517,t1518,t1519,t152,t1520,t1522,t1523,t1525,t1526,t1527,t1528,t1529,t153,t1530,t1531,t1532,t1533,t1535,t1536,t1537,t1538,t1539,t1541,t1542,t1543,t1544,t1545,t1546,t1547,t1549,t1550,t1551,t1552,t1554,t1555,t1556,t1558,t1559,t156,t1560,t1565,t1567,t1568,t1569,t1570,t1571,t1572,t1574,t1575,t1576,t1577,t1578,t1579,t158,t1581,t1582,t1583,t1584,t1585,t1586,t1587,t1588,t1591,t1592,t1593,t1594,t1595,t1596,t1599,t16,t160,t1600,t1601,t1602,t1604,t1605,t1606,t1607,t1608,t1609,t161,t1613,t1614,t1615,t1616,t1618,t1619,t162,t1620,t1621,t1622,t1624,t1625,t1626,t1627,t1628,t1629,t1631,t1633,t1634,t1635,t1636,t1637,t1639,t1640,t1641,t1642,t1643,t1644,t1645,t1646,t1648,t1649,t165,t1650,t1651,t1652,t1653,t1654,t1655,t1656,t1657,t1658,t1659,t1660,t1661,t1662,t1663,t1664,t1665,t1666,t1667,t1668,t1669,t167,t1670,t1671,t1672,t1673,t1674,t1675,t1676,t1677,t1678,t1679,t168,t1680,t1681,t1682,t1683,t1684,t1685,t1686,t1687,t1690,t1691,t1692,t1693,t1694,t1695,t1696,t1697,t1698,t1699,t17,t170,t1700,t1701,t1704,t1705,t1706,t1707,t1708,t1710,t1711,t1712,t1716,t1717,t172,t173,t1738,t1739,t174,t1740,t1741,t1742,t1743,t1745,t1749,t1750,t1751,t1752,t1753,t1754,t1756,t1757,t1758,t1759,t176,t1760,t1761,t1762,t1764,t1765,t1766,t1768,t1769,t177,t1770,t1771,t1772,t1773,t1775,t1776,t1777,t1779,t178,t1786,t1793,t1794,t1795,t1796,t1797,t1799,t18,t180,t1800,t1801,t1802,t1807,t1810,t1813,t1814,t1816,t1817,t1819,t182,t1820,t1821,t1822,t1823,t1824,t1825,t1826,t1827,t1828,t1829,t1830,t1831,t1832,t1834,t1835,t1836,t1837,t1840,t1841,t1842,t1843,t1844,t1845,t185,t1850,t1851,t1856,t1858,t186,t1860,t1861,t1862,t1865,t1866,t1868,t1870,t1871,t1874,t1875,t1876,t1878,t1879,t188,t1880,t1881,t1882,t1883,t1884,t1885,t1886,t1887,t1888,t1889,t189,t1890,t1891,t1892,t1898,t19,t1900,t1901,t1902,t1903,t1904,t1905,t1906,t1909,t191,t1910,t1911,t1913,t1914,t1917,t1918,t192,t1920,t1921,t1923,t1924,t1925,t1926,t1927,t1929,t1930,t1931,t1932,t1933,t1934,t1935,t1936,t1937,t1938,t1939,t1940,t1941,t1943,t1944,t1945,t1946,t1948,t195,t1951,t1952,t1953,t1954,t1955,t1956,t1957,t1958,t1959,t196,t1960,t1961,t1962,t1963,t1964,t1966,t1967,t1969,t197,t1971,t1972,t1973,t1978,t1979,t198,t1980,t1981,t1983,t1984,t1985,t1988,t1990,t1991,t1992,t1993,t1994,t1997,t1998,t1999,t20,t2001,t2002,t2003,t2004,t2005,t2006,t2007,t2008,t2009,t201,t2010,t2013,t2014,t2015,t2016,t2017,t202,t2023,t2024,t2027,t2028,t2029,t203,t2030,t2031,t2032,t2033,t2034,t2035,t2036,t2037,t2039,t204,t2040,t2041,t2042,t2043,t2044,t2045,t2049,t205,t2050,t2051,t2052,t2053,t2054,t2056,t2057,t2058,t2059,t2060,t2061,t2062,t2063,t2064,t2065,t2066,t2067,t2068,t2069,t207,t2070,t2071,t2072,t2073,t2074,t2075,t2077,t2078,t2079,t208,t2081,t2082,t2083,t2084,t2085,t2086,t2087,t2089,t209,t2090,t2091,t2093,t2094,t2095,t2098,t2099,t21,t2100,t2101,t2102,t2103,t2104,t2105,t2106,t2107,t2108,t2109,t211,t2110,t2111,t2112,t2113,t2114,t2115,t2116,t2117,t2118,t2119,t212,t2120,t2121,t2122,t2123,t2126,t2127,t2128,t2129,t2130,t2136,t2138,t2139,t2140,t2141,t2145,t2146,t2147,t2148,t2149,t2150,t2151,t2152,t2153,t2154,t2155,t2156,t2157,t2159,t216,t2160,t2161,t2162,t2164,t2165,t2166,t2167,t2168,t2169,t217,t2174,t2175,t2176,t2177,t2178,t2179,t218,t2180,t2181,t2182,t2183,t2184,t2185,t2186,t2187,t2188,t2189,t2190,t2191,t2192,t2193,t2194,t2195,t2196,t2197,t2198,t2199,t22,t2200,t2201,t2203,t2204,t2205,t2206,t2207,t2209,t221,t2210,t2211,t2212,t2213,t2214,t2215,t2217,t2218,t2219,t2220,t2221,t2222,t2223,t2224,t2225,t2226,t2227,t2228,t2229,t223,t2230,t2231,t2232,t2233,t2234,t2235,t2236,t2238,t2239,t2240,t2241,t2244,t2245,t2246,t2247,t2249,t225,t2250,t2251,t2252,t2253,t2255,t2256,t2257,t2259,t226,t2260,t2261,t2263,t227,t229,t2290,t2291,t2292,t2294,t2295,t2296,t2297,t2299,t230,t2300,t2302,t2303,t2304,t2305,t2306,t2308,t2309,t231,t2310,t2311,t2313,t2314,t2315,t2316,t2317,t2320,t2322,t2323,t2324,t2325,t2326,t2327,t2328,t2329,t2331,t2332,t2333,t2334,t2336,t2339,t2340,t2341,t2343,t2345,t2346,t2347,t2352,t2353,t2354,t2357,t2358,t2359,t236,t2360,t2361,t2362,t2363,t2364,t2365,t2366,t2367,t237,t2370,t2374,t2375,t2377,t2378,t2379,t238,t2380,t2382,t2384,t2385,t2386,t2389,t239,t2391,t2393,t2394,t2395,t2396,t2398,t24,t240,t2401,t2402,t2403,t2404,t2405,t2408,t2409,t241,t2411,t2413,t2414,t2416,t2417,t2418,t242,t2422,t2425,t2426,t2427,t243,t2431,t2432,t2433,t2434,t2438,t2440,t2441,t2444,t2446,t2447,t2448,t2449,t2450,t2451,t2452,t2455,t2457,t2458,t2459,t2460,t2461,t2463,t2466,t2467,t2471,t2472,t2473,t2474,t2476,t2477,t2478,t2479,t2480,t2481,t2482,t2484,t2485,t2487,t2488,t2489,t2490,t2491,t2492,t2493,t2494,t2498,t2499,t25,t2504,t2505,t2508,t2509,t2510,t2511,t2512,t2514,t2515,t2516,t2520,t2524,t2525,t2529,t2530,t2532,t2541,t2542,t2548,t2549,t2550,t2552,t2555,t2556,t2557,t2558,t2559,t2560,t2564,t2565,t2566,t2569,t257,t2570,t2571,t2572,t2577,t2578,t2579,t2580,t2581,t2582,t2583,t2584,t2585,t2586,t2587,t2589,t259,t2595,t2597,t2599,t26,t260,t2600,t2601,t2603,t2604,t2605,t2606,t261,t2610,t2611,t2612,t2613,t2614,t2616,t2618,t2619,t262,t2620,t2621,t2622,t2623,t2624,t2626,t2627,t2628,t2629,t263,t2630,t2632,t2633,t2634,t2635,t264,t2640,t2641,t2642,t2643,t2644,t2645,t2646,t2647,t2648,t2649,t2650,t2651,t2652,t2653,t2654,t2655,t2657,t2658,t2659,t2660,t2661,t2662,t2665,t2666,t2667,t2668,t267,t268,t2699,t27,t270,t271,t2718,t272,t2723,t2724,t2725,t2728,t2729,t273,t2730,t2731,t2734,t2735,t2736,t274,t2742,t2745,t2748,t2749,t275,t2750,t2753,t2754,t2759,t276,t2762,t2769,t2773,t2774,t2775,t2777,t2778,t2779,t2781,t2785,t2786,t2787,t2788,t279,t2790,t2792,t2795,t2796,t2797,t2798,t2799,t28,t280,t2802,t2803,t2805,t2807,t2808,t2811,t2812,t2814,t2823,t283,t285,t2857,t2858,t2859,t286,t2865,t2867,t2868,t2883,t2884,t2886,t2890,t2893,t2894,t2895,t2898,t29,t2900,t2901,t2903,t2905,t291,t2911,t2914,t2917,t2918,t2919,t292,t2920,t2922,t2923,t2925,t2926,t293,t2930,t2931,t2933,t2935,t295,t2962,t2963,t2964,t2965,t2966,t2969,t297,t2970,t30,t301,t303,t305,t306,t308,t309,t31,t310,t311,t312,t313,t314,t315,t316,t318,t319,t32,t320,t321,t322,t323,t325,t326,t328,t329,t33,t330,t331,t332,t333,t335,t336,t337,t338,t339,t34,t341,t343,t346,t348,t35,t350,t351,t352,t354,t355,t356,t358,t359,t36,t360,t361,t362,t363,t364,t365,t366,t368,t369,t370,t371,t372,t373,t377,t378,t38,t380,t381,t382,t385,t386,t387,t388,t389,t39,t391,t392,t393,t396,t3974,t3995,t404,t406,t408,t410,t411,t412,t413,t414,t419,t42,t420,t421,t422,t424,t425,t426,t4260,t428,t429,t43,t430,t432,t4325,t434,t4343,t435,t437,t438,t439,t444,t445,t448,t451,t452,t455,t456,t457,t458,t459,t46,t461,t463,t464,t465,t466,t467,t468,t469,t47,t4705,t471,t473,t474,t476,t478,t479,t480,t483,t485,t486,t488,t489,t49,t490,t491,t493,t494,t495,t496,t497,t498,t50,t503,t504,t506,t507,t508,t509,t510,t511,t512,t513,t514,t516,t517,t518,t521,t522,t523,t524,t525,t526,t527,t528,t53,t530,t531,t536,t538,t539,t54,t540,t542,t543,t544,t546,t547,t550,t551,t552,t553,t556,t56,t562,t563,t565,t568,t569,t571,t572,t573,t574,t575,t576,t577,t578,t58,t580,t582,t583,t584,t585,t589,t59,t590,t592,t597,t60,t600,t601,t605,t606,t607,t608,t609,t610,t611,t612,t614,t615,t616,t618,t620,t621,t622,t623,t624,t625,t627,t628,t629,t63,t631,t634,t635,t636,t638,t640,t641,t642,t643,t645,t646,t648,t649,t650,t651,t652,t654,t655,t656,t657,t658,t659,t660,t662,t663,t664,t665,t666,t667,t668,t669,t67,t670,t672,t673,t674,t675,t676,t677,t678,t679,t68,t681,t682,t683,t684,t685,t686,t687,t689,t691,t692,t693,t694,t696,t698,t70,t701,t702,t704,t705,t707,t708,t71,t710,t711,t712,t713,t714,t715,t716,t717,t718,t719,t720,t721,t722,t723,t724,t725,t726,t728,t73,t733,t735,t736,t738,t739,t740,t741,t742,t743,t744,t745,t746,t747,t749,t750,t751,t755,t756,t757,t758,t759,t76,t762,t763,t764,t765,t766,t767,t768,t770,t771,t772,t773,t774,t775,t776,t777,t778,t78,t781,t782,t783,t784,t785,t786,t787,t789,t79,t790,t791,t792,t793,t794,t796,t797,t798,t799,t8,t800,t801,t802,t806,t807,t808,t809,t812,t813,t816,t817,t818,t819,t820,t821,t822,t823,t824,t825,t826,t827,t828,t829,t830,t831,t832,t833,t836,t837,t838,t839,t841,t844,t846,t850,t852,t853,t855,t856,t857,t858,t859,t860,t861,t863,t865,t866,t868,t869,t870,t871,t872,t874,t876,t877,t878,t881,t882,t883,t885,t887,t889,t89,t890,t891,t893,t894,t895,t896,t898,t9,t90,t900,t902,t903,t904,t905,t906,t907,t908,t91,t911,t912,t914,t915,t916,t917,t918,t92,t921,t924,t926,t927,t930,t932,t933,t934,t935,t936,t937,t94,t940,t942,t943,t944,t945,t947,t948,t950,t951,t956,t959,t960,t961,t962,t965,t966,t967,t969,t97,t970,t974,t976,t978,t981,t983,t985,t987,t989,t99,t990,t992,t993,t994,t995,t996,t997,t998,t999});
end
function tau_c = ft_5(ct)
dq1 = ct{1};
dq2 = ct{2};
dq3 = ct{3};
dq4 = ct{4};
dq5 = ct{5};
dq6 = ct{6};
t10 = ct{7};
t100 = ct{8};
t1000 = ct{9};
t1001 = ct{10};
t1002 = ct{11};
t1003 = ct{12};
t1006 = ct{13};
t1009 = ct{14};
t101 = ct{15};
t1011 = ct{16};
t1014 = ct{17};
t1015 = ct{18};
t1017 = ct{19};
t1018 = ct{20};
t1019 = ct{21};
t1020 = ct{22};
t1021 = ct{23};
t1023 = ct{24};
t1024 = ct{25};
t1025 = ct{26};
t1028 = ct{27};
t1029 = ct{28};
t103 = ct{29};
t1030 = ct{30};
t1031 = ct{31};
t1032 = ct{32};
t1035 = ct{33};
t1038 = ct{34};
t1039 = ct{35};
t1041 = ct{36};
t1042 = ct{37};
t1044 = ct{38};
t1045 = ct{39};
t1046 = ct{40};
t1048 = ct{41};
t1049 = ct{42};
t1050 = ct{43};
t1051 = ct{44};
t1052 = ct{45};
t1055 = ct{46};
t1056 = ct{47};
t1057 = ct{48};
t1058 = ct{49};
t1059 = ct{50};
t106 = ct{51};
t1061 = ct{52};
t1062 = ct{53};
t1065 = ct{54};
t1066 = ct{55};
t1067 = ct{56};
t107 = ct{57};
t1070 = ct{58};
t1071 = ct{59};
t1072 = ct{60};
t1073 = ct{61};
t1074 = ct{62};
t1075 = ct{63};
t1076 = ct{64};
t108 = ct{65};
t1080 = ct{66};
t1083 = ct{67};
t1084 = ct{68};
t1089 = ct{69};
t109 = ct{70};
t1090 = ct{71};
t1091 = ct{72};
t1092 = ct{73};
t1094 = ct{74};
t1095 = ct{75};
t1098 = ct{76};
t1099 = ct{77};
t11 = ct{78};
t110 = ct{79};
t1100 = ct{80};
t1102 = ct{81};
t1103 = ct{82};
t1104 = ct{83};
t1105 = ct{84};
t1106 = ct{85};
t1107 = ct{86};
t1108 = ct{87};
t1109 = ct{88};
t111 = ct{89};
t1110 = ct{90};
t1111 = ct{91};
t1112 = ct{92};
t1113 = ct{93};
t1114 = ct{94};
t1115 = ct{95};
t1116 = ct{96};
t1117 = ct{97};
t1118 = ct{98};
t1119 = ct{99};
t1120 = ct{100};
t1121 = ct{101};
t1122 = ct{102};
t1123 = ct{103};
t1124 = ct{104};
t1125 = ct{105};
t1126 = ct{106};
t1129 = ct{107};
t113 = ct{108};
t1132 = ct{109};
t1135 = ct{110};
t1137 = ct{111};
t1138 = ct{112};
t1139 = ct{113};
t114 = ct{114};
t1140 = ct{115};
t1141 = ct{116};
t1142 = ct{117};
t1144 = ct{118};
t1145 = ct{119};
t1146 = ct{120};
t1147 = ct{121};
t1148 = ct{122};
t1149 = ct{123};
t1150 = ct{124};
t1154 = ct{125};
t1158 = ct{126};
t1159 = ct{127};
t1162 = ct{128};
t1165 = ct{129};
t1167 = ct{130};
t1174 = ct{131};
t1176 = ct{132};
t1177 = ct{133};
t1178 = ct{134};
t1179 = ct{135};
t1180 = ct{136};
t1185 = ct{137};
t1186 = ct{138};
t1187 = ct{139};
t1188 = ct{140};
t1189 = ct{141};
t1190 = ct{142};
t1192 = ct{143};
t1193 = ct{144};
t1194 = ct{145};
t1195 = ct{146};
t1196 = ct{147};
t1198 = ct{148};
t1199 = ct{149};
t12 = ct{150};
t120 = ct{151};
t1203 = ct{152};
t1204 = ct{153};
t1205 = ct{154};
t1206 = ct{155};
t1207 = ct{156};
t1208 = ct{157};
t1209 = ct{158};
t121 = ct{159};
t1210 = ct{160};
t1212 = ct{161};
t1213 = ct{162};
t1214 = ct{163};
t1217 = ct{164};
t1218 = ct{165};
t1219 = ct{166};
t1220 = ct{167};
t1221 = ct{168};
t1222 = ct{169};
t1224 = ct{170};
t1229 = ct{171};
t123 = ct{172};
t1230 = ct{173};
t1232 = ct{174};
t1234 = ct{175};
t1235 = ct{176};
t1236 = ct{177};
t1237 = ct{178};
t1238 = ct{179};
t124 = ct{180};
t1241 = ct{181};
t1245 = ct{182};
t1246 = ct{183};
t1247 = ct{184};
t1248 = ct{185};
t1251 = ct{186};
t1252 = ct{187};
t1253 = ct{188};
t1255 = ct{189};
t1259 = ct{190};
t126 = ct{191};
t1260 = ct{192};
t1261 = ct{193};
t1262 = ct{194};
t1263 = ct{195};
t1264 = ct{196};
t1265 = ct{197};
t1266 = ct{198};
t1267 = ct{199};
t1268 = ct{200};
t127 = ct{201};
t1270 = ct{202};
t1271 = ct{203};
t1272 = ct{204};
t1277 = ct{205};
t1278 = ct{206};
t128 = ct{207};
t1280 = ct{208};
t1281 = ct{209};
t1285 = ct{210};
t1286 = ct{211};
t1287 = ct{212};
t1288 = ct{213};
t1289 = ct{214};
t1290 = ct{215};
t1292 = ct{216};
t1294 = ct{217};
t1296 = ct{218};
t1297 = ct{219};
t1298 = ct{220};
t1299 = ct{221};
t13 = ct{222};
t130 = ct{223};
t1300 = ct{224};
t1301 = ct{225};
t1302 = ct{226};
t1303 = ct{227};
t1304 = ct{228};
t1305 = ct{229};
t1307 = ct{230};
t1310 = ct{231};
t1311 = ct{232};
t1316 = ct{233};
t1317 = ct{234};
t1319 = ct{235};
t132 = ct{236};
t1320 = ct{237};
t1322 = ct{238};
t1323 = ct{239};
t1324 = ct{240};
t1325 = ct{241};
t1326 = ct{242};
t1328 = ct{243};
t133 = ct{244};
t1330 = ct{245};
t1331 = ct{246};
t1332 = ct{247};
t1334 = ct{248};
t1335 = ct{249};
t1336 = ct{250};
t1337 = ct{251};
t1338 = ct{252};
t134 = ct{253};
t1342 = ct{254};
t1343 = ct{255};
t1344 = ct{256};
t1345 = ct{257};
t1348 = ct{258};
t1349 = ct{259};
t1350 = ct{260};
t1351 = ct{261};
t1352 = ct{262};
t1353 = ct{263};
t1354 = ct{264};
t136 = ct{265};
t1360 = ct{266};
t1364 = ct{267};
t1366 = ct{268};
t1367 = ct{269};
t1368 = ct{270};
t1369 = ct{271};
t1370 = ct{272};
t1371 = ct{273};
t1372 = ct{274};
t1374 = ct{275};
t1375 = ct{276};
t1376 = ct{277};
t1377 = ct{278};
t1378 = ct{279};
t1379 = ct{280};
t138 = ct{281};
t1380 = ct{282};
t1383 = ct{283};
t1385 = ct{284};
t1386 = ct{285};
t1387 = ct{286};
t1388 = ct{287};
t1389 = ct{288};
t139 = ct{289};
t1392 = ct{290};
t1393 = ct{291};
t1394 = ct{292};
t1395 = ct{293};
t1396 = ct{294};
t1397 = ct{295};
t1398 = ct{296};
t1399 = ct{297};
t14 = ct{298};
t140 = ct{299};
t1401 = ct{300};
t1402 = ct{301};
t1403 = ct{302};
t1404 = ct{303};
t1405 = ct{304};
t1406 = ct{305};
t1407 = ct{306};
t1408 = ct{307};
t1409 = ct{308};
t1410 = ct{309};
t1411 = ct{310};
t1412 = ct{311};
t1413 = ct{312};
t1414 = ct{313};
t1415 = ct{314};
t1416 = ct{315};
t1417 = ct{316};
t1418 = ct{317};
t1419 = ct{318};
t1420 = ct{319};
t1421 = ct{320};
t1422 = ct{321};
t1423 = ct{322};
t1424 = ct{323};
t1425 = ct{324};
t1426 = ct{325};
t1427 = ct{326};
t1428 = ct{327};
t1429 = ct{328};
t1430 = ct{329};
t1431 = ct{330};
t1432 = ct{331};
t1433 = ct{332};
t1434 = ct{333};
t1435 = ct{334};
t1436 = ct{335};
t1437 = ct{336};
t1439 = ct{337};
t144 = ct{338};
t1440 = ct{339};
t1441 = ct{340};
t1443 = ct{341};
t1444 = ct{342};
t1445 = ct{343};
t1446 = ct{344};
t1447 = ct{345};
t1448 = ct{346};
t1451 = ct{347};
t1453 = ct{348};
t1456 = ct{349};
t1457 = ct{350};
t1458 = ct{351};
t1459 = ct{352};
t1460 = ct{353};
t1461 = ct{354};
t1462 = ct{355};
t1463 = ct{356};
t1464 = ct{357};
t1468 = ct{358};
t1469 = ct{359};
t1471 = ct{360};
t1477 = ct{361};
t1478 = ct{362};
t1479 = ct{363};
t148 = ct{364};
t1480 = ct{365};
t1481 = ct{366};
t1482 = ct{367};
t1483 = ct{368};
t1484 = ct{369};
t1485 = ct{370};
t1486 = ct{371};
t1487 = ct{372};
t1488 = ct{373};
t1489 = ct{374};
t149 = ct{375};
t1490 = ct{376};
t1491 = ct{377};
t1492 = ct{378};
t1493 = ct{379};
t1494 = ct{380};
t1495 = ct{381};
t1497 = ct{382};
t1498 = ct{383};
t1499 = ct{384};
t15 = ct{385};
t150 = ct{386};
t1500 = ct{387};
t1501 = ct{388};
t1503 = ct{389};
t1504 = ct{390};
t1505 = ct{391};
t1506 = ct{392};
t1507 = ct{393};
t1509 = ct{394};
t151 = ct{395};
t1510 = ct{396};
t1512 = ct{397};
t1513 = ct{398};
t1514 = ct{399};
t1515 = ct{400};
t1516 = ct{401};
t1517 = ct{402};
t1518 = ct{403};
t1519 = ct{404};
t152 = ct{405};
t1520 = ct{406};
t1522 = ct{407};
t1523 = ct{408};
t1525 = ct{409};
t1526 = ct{410};
t1527 = ct{411};
t1528 = ct{412};
t1529 = ct{413};
t153 = ct{414};
t1530 = ct{415};
t1531 = ct{416};
t1532 = ct{417};
t1533 = ct{418};
t1535 = ct{419};
t1536 = ct{420};
t1537 = ct{421};
t1538 = ct{422};
t1539 = ct{423};
t1541 = ct{424};
t1542 = ct{425};
t1543 = ct{426};
t1544 = ct{427};
t1545 = ct{428};
t1546 = ct{429};
t1547 = ct{430};
t1549 = ct{431};
t1550 = ct{432};
t1551 = ct{433};
t1552 = ct{434};
t1554 = ct{435};
t1555 = ct{436};
t1556 = ct{437};
t1558 = ct{438};
t1559 = ct{439};
t156 = ct{440};
t1560 = ct{441};
t1565 = ct{442};
t1567 = ct{443};
t1568 = ct{444};
t1569 = ct{445};
t1570 = ct{446};
t1571 = ct{447};
t1572 = ct{448};
t1574 = ct{449};
t1575 = ct{450};
t1576 = ct{451};
t1577 = ct{452};
t1578 = ct{453};
t1579 = ct{454};
t158 = ct{455};
t1581 = ct{456};
t1582 = ct{457};
t1583 = ct{458};
t1584 = ct{459};
t1585 = ct{460};
t1586 = ct{461};
t1587 = ct{462};
t1588 = ct{463};
t1591 = ct{464};
t1592 = ct{465};
t1593 = ct{466};
t1594 = ct{467};
t1595 = ct{468};
t1596 = ct{469};
t1599 = ct{470};
t16 = ct{471};
t160 = ct{472};
t1600 = ct{473};
t1601 = ct{474};
t1602 = ct{475};
t1604 = ct{476};
t1605 = ct{477};
t1606 = ct{478};
t1607 = ct{479};
t1608 = ct{480};
t1609 = ct{481};
t161 = ct{482};
t1613 = ct{483};
t1614 = ct{484};
t1615 = ct{485};
t1616 = ct{486};
t1618 = ct{487};
t1619 = ct{488};
t162 = ct{489};
t1620 = ct{490};
t1621 = ct{491};
t1622 = ct{492};
t1624 = ct{493};
t1625 = ct{494};
t1626 = ct{495};
t1627 = ct{496};
t1628 = ct{497};
t1629 = ct{498};
t1631 = ct{499};
t1633 = ct{500};
t1634 = ct{501};
t1635 = ct{502};
t1636 = ct{503};
t1637 = ct{504};
t1639 = ct{505};
t1640 = ct{506};
t1641 = ct{507};
t1642 = ct{508};
t1643 = ct{509};
t1644 = ct{510};
t1645 = ct{511};
t1646 = ct{512};
t1648 = ct{513};
t1649 = ct{514};
t165 = ct{515};
t1650 = ct{516};
t1651 = ct{517};
t1652 = ct{518};
t1653 = ct{519};
t1654 = ct{520};
t1655 = ct{521};
t1656 = ct{522};
t1657 = ct{523};
t1658 = ct{524};
t1659 = ct{525};
t1660 = ct{526};
t1661 = ct{527};
t1662 = ct{528};
t1663 = ct{529};
t1664 = ct{530};
t1665 = ct{531};
t1666 = ct{532};
t1667 = ct{533};
t1668 = ct{534};
t1669 = ct{535};
t167 = ct{536};
t1670 = ct{537};
t1671 = ct{538};
t1672 = ct{539};
t1673 = ct{540};
t1674 = ct{541};
t1675 = ct{542};
t1676 = ct{543};
t1677 = ct{544};
t1678 = ct{545};
t1679 = ct{546};
t168 = ct{547};
t1680 = ct{548};
t1681 = ct{549};
t1682 = ct{550};
t1683 = ct{551};
t1684 = ct{552};
t1685 = ct{553};
t1686 = ct{554};
t1687 = ct{555};
t1690 = ct{556};
t1691 = ct{557};
t1692 = ct{558};
t1693 = ct{559};
t1694 = ct{560};
t1695 = ct{561};
t1696 = ct{562};
t1697 = ct{563};
t1698 = ct{564};
t1699 = ct{565};
t17 = ct{566};
t170 = ct{567};
t1700 = ct{568};
t1701 = ct{569};
t1704 = ct{570};
t1705 = ct{571};
t1706 = ct{572};
t1707 = ct{573};
t1708 = ct{574};
t1710 = ct{575};
t1711 = ct{576};
t1712 = ct{577};
t1716 = ct{578};
t1717 = ct{579};
t172 = ct{580};
t173 = ct{581};
t1738 = ct{582};
t1739 = ct{583};
t174 = ct{584};
t1740 = ct{585};
t1741 = ct{586};
t1742 = ct{587};
t1743 = ct{588};
t1745 = ct{589};
t1749 = ct{590};
t1750 = ct{591};
t1751 = ct{592};
t1752 = ct{593};
t1753 = ct{594};
t1754 = ct{595};
t1756 = ct{596};
t1757 = ct{597};
t1758 = ct{598};
t1759 = ct{599};
t176 = ct{600};
t1760 = ct{601};
t1761 = ct{602};
t1762 = ct{603};
t1764 = ct{604};
t1765 = ct{605};
t1766 = ct{606};
t1768 = ct{607};
t1769 = ct{608};
t177 = ct{609};
t1770 = ct{610};
t1771 = ct{611};
t1772 = ct{612};
t1773 = ct{613};
t1775 = ct{614};
t1776 = ct{615};
t1777 = ct{616};
t1779 = ct{617};
t178 = ct{618};
t1786 = ct{619};
t1793 = ct{620};
t1794 = ct{621};
t1795 = ct{622};
t1796 = ct{623};
t1797 = ct{624};
t1799 = ct{625};
t18 = ct{626};
t180 = ct{627};
t1800 = ct{628};
t1801 = ct{629};
t1802 = ct{630};
t1807 = ct{631};
t1810 = ct{632};
t1813 = ct{633};
t1814 = ct{634};
t1816 = ct{635};
t1817 = ct{636};
t1819 = ct{637};
t182 = ct{638};
t1820 = ct{639};
t1821 = ct{640};
t1822 = ct{641};
t1823 = ct{642};
t1824 = ct{643};
t1825 = ct{644};
t1826 = ct{645};
t1827 = ct{646};
t1828 = ct{647};
t1829 = ct{648};
t1830 = ct{649};
t1831 = ct{650};
t1832 = ct{651};
t1834 = ct{652};
t1835 = ct{653};
t1836 = ct{654};
t1837 = ct{655};
t1840 = ct{656};
t1841 = ct{657};
t1842 = ct{658};
t1843 = ct{659};
t1844 = ct{660};
t1845 = ct{661};
t185 = ct{662};
t1850 = ct{663};
t1851 = ct{664};
t1856 = ct{665};
t1858 = ct{666};
t186 = ct{667};
t1860 = ct{668};
t1861 = ct{669};
t1862 = ct{670};
t1865 = ct{671};
t1866 = ct{672};
t1868 = ct{673};
t1870 = ct{674};
t1871 = ct{675};
t1874 = ct{676};
t1875 = ct{677};
t1876 = ct{678};
t1878 = ct{679};
t1879 = ct{680};
t188 = ct{681};
t1880 = ct{682};
t1881 = ct{683};
t1882 = ct{684};
t1883 = ct{685};
t1884 = ct{686};
t1885 = ct{687};
t1886 = ct{688};
t1887 = ct{689};
t1888 = ct{690};
t1889 = ct{691};
t189 = ct{692};
t1890 = ct{693};
t1891 = ct{694};
t1892 = ct{695};
t1898 = ct{696};
t19 = ct{697};
t1900 = ct{698};
t1901 = ct{699};
t1902 = ct{700};
t1903 = ct{701};
t1904 = ct{702};
t1905 = ct{703};
t1906 = ct{704};
t1909 = ct{705};
t191 = ct{706};
t1910 = ct{707};
t1911 = ct{708};
t1913 = ct{709};
t1914 = ct{710};
t1917 = ct{711};
t1918 = ct{712};
t192 = ct{713};
t1920 = ct{714};
t1921 = ct{715};
t1923 = ct{716};
t1924 = ct{717};
t1925 = ct{718};
t1926 = ct{719};
t1927 = ct{720};
t1929 = ct{721};
t1930 = ct{722};
t1931 = ct{723};
t1932 = ct{724};
t1933 = ct{725};
t1934 = ct{726};
t1935 = ct{727};
t1936 = ct{728};
t1937 = ct{729};
t1938 = ct{730};
t1939 = ct{731};
t1940 = ct{732};
t1941 = ct{733};
t1943 = ct{734};
t1944 = ct{735};
t1945 = ct{736};
t1946 = ct{737};
t1948 = ct{738};
t195 = ct{739};
t1951 = ct{740};
t1952 = ct{741};
t1953 = ct{742};
t1954 = ct{743};
t1955 = ct{744};
t1956 = ct{745};
t1957 = ct{746};
t1958 = ct{747};
t1959 = ct{748};
t196 = ct{749};
t1960 = ct{750};
t1961 = ct{751};
t1962 = ct{752};
t1963 = ct{753};
t1964 = ct{754};
t1966 = ct{755};
t1967 = ct{756};
t1969 = ct{757};
t197 = ct{758};
t1971 = ct{759};
t1972 = ct{760};
t1973 = ct{761};
t1978 = ct{762};
t1979 = ct{763};
t198 = ct{764};
t1980 = ct{765};
t1981 = ct{766};
t1983 = ct{767};
t1984 = ct{768};
t1985 = ct{769};
t1988 = ct{770};
t1990 = ct{771};
t1991 = ct{772};
t1992 = ct{773};
t1993 = ct{774};
t1994 = ct{775};
t1997 = ct{776};
t1998 = ct{777};
t1999 = ct{778};
t20 = ct{779};
t2001 = ct{780};
t2002 = ct{781};
t2003 = ct{782};
t2004 = ct{783};
t2005 = ct{784};
t2006 = ct{785};
t2007 = ct{786};
t2008 = ct{787};
t2009 = ct{788};
t201 = ct{789};
t2010 = ct{790};
t2013 = ct{791};
t2014 = ct{792};
t2015 = ct{793};
t2016 = ct{794};
t2017 = ct{795};
t202 = ct{796};
t2023 = ct{797};
t2024 = ct{798};
t2027 = ct{799};
t2028 = ct{800};
t2029 = ct{801};
t203 = ct{802};
t2030 = ct{803};
t2031 = ct{804};
t2032 = ct{805};
t2033 = ct{806};
t2034 = ct{807};
t2035 = ct{808};
t2036 = ct{809};
t2037 = ct{810};
t2039 = ct{811};
t204 = ct{812};
t2040 = ct{813};
t2041 = ct{814};
t2042 = ct{815};
t2043 = ct{816};
t2044 = ct{817};
t2045 = ct{818};
t2049 = ct{819};
t205 = ct{820};
t2050 = ct{821};
t2051 = ct{822};
t2052 = ct{823};
t2053 = ct{824};
t2054 = ct{825};
t2056 = ct{826};
t2057 = ct{827};
t2058 = ct{828};
t2059 = ct{829};
t2060 = ct{830};
t2061 = ct{831};
t2062 = ct{832};
t2063 = ct{833};
t2064 = ct{834};
t2065 = ct{835};
t2066 = ct{836};
t2067 = ct{837};
t2068 = ct{838};
t2069 = ct{839};
t207 = ct{840};
t2070 = ct{841};
t2071 = ct{842};
t2072 = ct{843};
t2073 = ct{844};
t2074 = ct{845};
t2075 = ct{846};
t2077 = ct{847};
t2078 = ct{848};
t2079 = ct{849};
t208 = ct{850};
t2081 = ct{851};
t2082 = ct{852};
t2083 = ct{853};
t2084 = ct{854};
t2085 = ct{855};
t2086 = ct{856};
t2087 = ct{857};
t2089 = ct{858};
t209 = ct{859};
t2090 = ct{860};
t2091 = ct{861};
t2093 = ct{862};
t2094 = ct{863};
t2095 = ct{864};
t2098 = ct{865};
t2099 = ct{866};
t21 = ct{867};
t2100 = ct{868};
t2101 = ct{869};
t2102 = ct{870};
t2103 = ct{871};
t2104 = ct{872};
t2105 = ct{873};
t2106 = ct{874};
t2107 = ct{875};
t2108 = ct{876};
t2109 = ct{877};
t211 = ct{878};
t2110 = ct{879};
t2111 = ct{880};
t2112 = ct{881};
t2113 = ct{882};
t2114 = ct{883};
t2115 = ct{884};
t2116 = ct{885};
t2117 = ct{886};
t2118 = ct{887};
t2119 = ct{888};
t212 = ct{889};
t2120 = ct{890};
t2121 = ct{891};
t2122 = ct{892};
t2123 = ct{893};
t2126 = ct{894};
t2127 = ct{895};
t2128 = ct{896};
t2129 = ct{897};
t2130 = ct{898};
t2136 = ct{899};
t2138 = ct{900};
t2139 = ct{901};
t2140 = ct{902};
t2141 = ct{903};
t2145 = ct{904};
t2146 = ct{905};
t2147 = ct{906};
t2148 = ct{907};
t2149 = ct{908};
t2150 = ct{909};
t2151 = ct{910};
t2152 = ct{911};
t2153 = ct{912};
t2154 = ct{913};
t2155 = ct{914};
t2156 = ct{915};
t2157 = ct{916};
t2159 = ct{917};
t216 = ct{918};
t2160 = ct{919};
t2161 = ct{920};
t2162 = ct{921};
t2164 = ct{922};
t2165 = ct{923};
t2166 = ct{924};
t2167 = ct{925};
t2168 = ct{926};
t2169 = ct{927};
t217 = ct{928};
t2174 = ct{929};
t2175 = ct{930};
t2176 = ct{931};
t2177 = ct{932};
t2178 = ct{933};
t2179 = ct{934};
t218 = ct{935};
t2180 = ct{936};
t2181 = ct{937};
t2182 = ct{938};
t2183 = ct{939};
t2184 = ct{940};
t2185 = ct{941};
t2186 = ct{942};
t2187 = ct{943};
t2188 = ct{944};
t2189 = ct{945};
t2190 = ct{946};
t2191 = ct{947};
t2192 = ct{948};
t2193 = ct{949};
t2194 = ct{950};
t2195 = ct{951};
t2196 = ct{952};
t2197 = ct{953};
t2198 = ct{954};
t2199 = ct{955};
t22 = ct{956};
t2200 = ct{957};
t2201 = ct{958};
t2203 = ct{959};
t2204 = ct{960};
t2205 = ct{961};
t2206 = ct{962};
t2207 = ct{963};
t2209 = ct{964};
t221 = ct{965};
t2210 = ct{966};
t2211 = ct{967};
t2212 = ct{968};
t2213 = ct{969};
t2214 = ct{970};
t2215 = ct{971};
t2217 = ct{972};
t2218 = ct{973};
t2219 = ct{974};
t2220 = ct{975};
t2221 = ct{976};
t2222 = ct{977};
t2223 = ct{978};
t2224 = ct{979};
t2225 = ct{980};
t2226 = ct{981};
t2227 = ct{982};
t2228 = ct{983};
t2229 = ct{984};
t223 = ct{985};
t2230 = ct{986};
t2231 = ct{987};
t2232 = ct{988};
t2233 = ct{989};
t2234 = ct{990};
t2235 = ct{991};
t2236 = ct{992};
t2238 = ct{993};
t2239 = ct{994};
t2240 = ct{995};
t2241 = ct{996};
t2244 = ct{997};
t2245 = ct{998};
t2246 = ct{999};
t2247 = ct{1000};
t2249 = ct{1001};
t225 = ct{1002};
t2250 = ct{1003};
t2251 = ct{1004};
t2252 = ct{1005};
t2253 = ct{1006};
t2255 = ct{1007};
t2256 = ct{1008};
t2257 = ct{1009};
t2259 = ct{1010};
t226 = ct{1011};
t2260 = ct{1012};
t2261 = ct{1013};
t2263 = ct{1014};
t227 = ct{1015};
t229 = ct{1016};
t2290 = ct{1017};
t2291 = ct{1018};
t2292 = ct{1019};
t2294 = ct{1020};
t2295 = ct{1021};
t2296 = ct{1022};
t2297 = ct{1023};
t2299 = ct{1024};
t230 = ct{1025};
t2300 = ct{1026};
t2302 = ct{1027};
t2303 = ct{1028};
t2304 = ct{1029};
t2305 = ct{1030};
t2306 = ct{1031};
t2308 = ct{1032};
t2309 = ct{1033};
t231 = ct{1034};
t2310 = ct{1035};
t2311 = ct{1036};
t2313 = ct{1037};
t2314 = ct{1038};
t2315 = ct{1039};
t2316 = ct{1040};
t2317 = ct{1041};
t2320 = ct{1042};
t2322 = ct{1043};
t2323 = ct{1044};
t2324 = ct{1045};
t2325 = ct{1046};
t2326 = ct{1047};
t2327 = ct{1048};
t2328 = ct{1049};
t2329 = ct{1050};
t2331 = ct{1051};
t2332 = ct{1052};
t2333 = ct{1053};
t2334 = ct{1054};
t2336 = ct{1055};
t2339 = ct{1056};
t2340 = ct{1057};
t2341 = ct{1058};
t2343 = ct{1059};
t2345 = ct{1060};
t2346 = ct{1061};
t2347 = ct{1062};
t2352 = ct{1063};
t2353 = ct{1064};
t2354 = ct{1065};
t2357 = ct{1066};
t2358 = ct{1067};
t2359 = ct{1068};
t236 = ct{1069};
t2360 = ct{1070};
t2361 = ct{1071};
t2362 = ct{1072};
t2363 = ct{1073};
t2364 = ct{1074};
t2365 = ct{1075};
t2366 = ct{1076};
t2367 = ct{1077};
t237 = ct{1078};
t2370 = ct{1079};
t2374 = ct{1080};
t2375 = ct{1081};
t2377 = ct{1082};
t2378 = ct{1083};
t2379 = ct{1084};
t238 = ct{1085};
t2380 = ct{1086};
t2382 = ct{1087};
t2384 = ct{1088};
t2385 = ct{1089};
t2386 = ct{1090};
t2389 = ct{1091};
t239 = ct{1092};
t2391 = ct{1093};
t2393 = ct{1094};
t2394 = ct{1095};
t2395 = ct{1096};
t2396 = ct{1097};
t2398 = ct{1098};
t24 = ct{1099};
t240 = ct{1100};
t2401 = ct{1101};
t2402 = ct{1102};
t2403 = ct{1103};
t2404 = ct{1104};
t2405 = ct{1105};
t2408 = ct{1106};
t2409 = ct{1107};
t241 = ct{1108};
t2411 = ct{1109};
t2413 = ct{1110};
t2414 = ct{1111};
t2416 = ct{1112};
t2417 = ct{1113};
t2418 = ct{1114};
t242 = ct{1115};
t2422 = ct{1116};
t2425 = ct{1117};
t2426 = ct{1118};
t2427 = ct{1119};
t243 = ct{1120};
t2431 = ct{1121};
t2432 = ct{1122};
t2433 = ct{1123};
t2434 = ct{1124};
t2438 = ct{1125};
t2440 = ct{1126};
t2441 = ct{1127};
t2444 = ct{1128};
t2446 = ct{1129};
t2447 = ct{1130};
t2448 = ct{1131};
t2449 = ct{1132};
t2450 = ct{1133};
t2451 = ct{1134};
t2452 = ct{1135};
t2455 = ct{1136};
t2457 = ct{1137};
t2458 = ct{1138};
t2459 = ct{1139};
t2460 = ct{1140};
t2461 = ct{1141};
t2463 = ct{1142};
t2466 = ct{1143};
t2467 = ct{1144};
t2471 = ct{1145};
t2472 = ct{1146};
t2473 = ct{1147};
t2474 = ct{1148};
t2476 = ct{1149};
t2477 = ct{1150};
t2478 = ct{1151};
t2479 = ct{1152};
t2480 = ct{1153};
t2481 = ct{1154};
t2482 = ct{1155};
t2484 = ct{1156};
t2485 = ct{1157};
t2487 = ct{1158};
t2488 = ct{1159};
t2489 = ct{1160};
t2490 = ct{1161};
t2491 = ct{1162};
t2492 = ct{1163};
t2493 = ct{1164};
t2494 = ct{1165};
t2498 = ct{1166};
t2499 = ct{1167};
t25 = ct{1168};
t2504 = ct{1169};
t2505 = ct{1170};
t2508 = ct{1171};
t2509 = ct{1172};
t2510 = ct{1173};
t2511 = ct{1174};
t2512 = ct{1175};
t2514 = ct{1176};
t2515 = ct{1177};
t2516 = ct{1178};
t2520 = ct{1179};
t2524 = ct{1180};
t2525 = ct{1181};
t2529 = ct{1182};
t2530 = ct{1183};
t2532 = ct{1184};
t2541 = ct{1185};
t2542 = ct{1186};
t2548 = ct{1187};
t2549 = ct{1188};
t2550 = ct{1189};
t2552 = ct{1190};
t2555 = ct{1191};
t2556 = ct{1192};
t2557 = ct{1193};
t2558 = ct{1194};
t2559 = ct{1195};
t2560 = ct{1196};
t2564 = ct{1197};
t2565 = ct{1198};
t2566 = ct{1199};
t2569 = ct{1200};
t257 = ct{1201};
t2570 = ct{1202};
t2571 = ct{1203};
t2572 = ct{1204};
t2577 = ct{1205};
t2578 = ct{1206};
t2579 = ct{1207};
t2580 = ct{1208};
t2581 = ct{1209};
t2582 = ct{1210};
t2583 = ct{1211};
t2584 = ct{1212};
t2585 = ct{1213};
t2586 = ct{1214};
t2587 = ct{1215};
t2589 = ct{1216};
t259 = ct{1217};
t2595 = ct{1218};
t2597 = ct{1219};
t2599 = ct{1220};
t26 = ct{1221};
t260 = ct{1222};
t2600 = ct{1223};
t2601 = ct{1224};
t2603 = ct{1225};
t2604 = ct{1226};
t2605 = ct{1227};
t2606 = ct{1228};
t261 = ct{1229};
t2610 = ct{1230};
t2611 = ct{1231};
t2612 = ct{1232};
t2613 = ct{1233};
t2614 = ct{1234};
t2616 = ct{1235};
t2618 = ct{1236};
t2619 = ct{1237};
t262 = ct{1238};
t2620 = ct{1239};
t2621 = ct{1240};
t2622 = ct{1241};
t2623 = ct{1242};
t2624 = ct{1243};
t2626 = ct{1244};
t2627 = ct{1245};
t2628 = ct{1246};
t2629 = ct{1247};
t263 = ct{1248};
t2630 = ct{1249};
t2632 = ct{1250};
t2633 = ct{1251};
t2634 = ct{1252};
t2635 = ct{1253};
t264 = ct{1254};
t2640 = ct{1255};
t2641 = ct{1256};
t2642 = ct{1257};
t2643 = ct{1258};
t2644 = ct{1259};
t2645 = ct{1260};
t2646 = ct{1261};
t2647 = ct{1262};
t2648 = ct{1263};
t2649 = ct{1264};
t2650 = ct{1265};
t2651 = ct{1266};
t2652 = ct{1267};
t2653 = ct{1268};
t2654 = ct{1269};
t2655 = ct{1270};
t2657 = ct{1271};
t2658 = ct{1272};
t2659 = ct{1273};
t2660 = ct{1274};
t2661 = ct{1275};
t2662 = ct{1276};
t2665 = ct{1277};
t2666 = ct{1278};
t2667 = ct{1279};
t2668 = ct{1280};
t267 = ct{1281};
t268 = ct{1282};
t2699 = ct{1283};
t27 = ct{1284};
t270 = ct{1285};
t271 = ct{1286};
t2718 = ct{1287};
t272 = ct{1288};
t2723 = ct{1289};
t2724 = ct{1290};
t2725 = ct{1291};
t2728 = ct{1292};
t2729 = ct{1293};
t273 = ct{1294};
t2730 = ct{1295};
t2731 = ct{1296};
t2734 = ct{1297};
t2735 = ct{1298};
t2736 = ct{1299};
t274 = ct{1300};
t2742 = ct{1301};
t2745 = ct{1302};
t2748 = ct{1303};
t2749 = ct{1304};
t275 = ct{1305};
t2750 = ct{1306};
t2753 = ct{1307};
t2754 = ct{1308};
t2759 = ct{1309};
t276 = ct{1310};
t2762 = ct{1311};
t2769 = ct{1312};
t2773 = ct{1313};
t2774 = ct{1314};
t2775 = ct{1315};
t2777 = ct{1316};
t2778 = ct{1317};
t2779 = ct{1318};
t2781 = ct{1319};
t2785 = ct{1320};
t2786 = ct{1321};
t2787 = ct{1322};
t2788 = ct{1323};
t279 = ct{1324};
t2790 = ct{1325};
t2792 = ct{1326};
t2795 = ct{1327};
t2796 = ct{1328};
t2797 = ct{1329};
t2798 = ct{1330};
t2799 = ct{1331};
t28 = ct{1332};
t280 = ct{1333};
t2802 = ct{1334};
t2803 = ct{1335};
t2805 = ct{1336};
t2807 = ct{1337};
t2808 = ct{1338};
t2811 = ct{1339};
t2812 = ct{1340};
t2814 = ct{1341};
t2823 = ct{1342};
t283 = ct{1343};
t285 = ct{1344};
t2857 = ct{1345};
t2858 = ct{1346};
t2859 = ct{1347};
t286 = ct{1348};
t2865 = ct{1349};
t2867 = ct{1350};
t2868 = ct{1351};
t2883 = ct{1352};
t2884 = ct{1353};
t2886 = ct{1354};
t2890 = ct{1355};
t2893 = ct{1356};
t2894 = ct{1357};
t2895 = ct{1358};
t2898 = ct{1359};
t29 = ct{1360};
t2900 = ct{1361};
t2901 = ct{1362};
t2903 = ct{1363};
t2905 = ct{1364};
t291 = ct{1365};
t2911 = ct{1366};
t2914 = ct{1367};
t2917 = ct{1368};
t2918 = ct{1369};
t2919 = ct{1370};
t292 = ct{1371};
t2920 = ct{1372};
t2922 = ct{1373};
t2923 = ct{1374};
t2925 = ct{1375};
t2926 = ct{1376};
t293 = ct{1377};
t2930 = ct{1378};
t2931 = ct{1379};
t2933 = ct{1380};
t2935 = ct{1381};
t295 = ct{1382};
t2962 = ct{1383};
t2963 = ct{1384};
t2964 = ct{1385};
t2965 = ct{1386};
t2966 = ct{1387};
t2969 = ct{1388};
t297 = ct{1389};
t2970 = ct{1390};
t30 = ct{1391};
t301 = ct{1392};
t303 = ct{1393};
t305 = ct{1394};
t306 = ct{1395};
t308 = ct{1396};
t309 = ct{1397};
t31 = ct{1398};
t310 = ct{1399};
t311 = ct{1400};
t312 = ct{1401};
t313 = ct{1402};
t314 = ct{1403};
t315 = ct{1404};
t316 = ct{1405};
t318 = ct{1406};
t319 = ct{1407};
t32 = ct{1408};
t320 = ct{1409};
t321 = ct{1410};
t322 = ct{1411};
t323 = ct{1412};
t325 = ct{1413};
t326 = ct{1414};
t328 = ct{1415};
t329 = ct{1416};
t33 = ct{1417};
t330 = ct{1418};
t331 = ct{1419};
t332 = ct{1420};
t333 = ct{1421};
t335 = ct{1422};
t336 = ct{1423};
t337 = ct{1424};
t338 = ct{1425};
t339 = ct{1426};
t34 = ct{1427};
t341 = ct{1428};
t343 = ct{1429};
t346 = ct{1430};
t348 = ct{1431};
t35 = ct{1432};
t350 = ct{1433};
t351 = ct{1434};
t352 = ct{1435};
t354 = ct{1436};
t355 = ct{1437};
t356 = ct{1438};
t358 = ct{1439};
t359 = ct{1440};
t36 = ct{1441};
t360 = ct{1442};
t361 = ct{1443};
t362 = ct{1444};
t363 = ct{1445};
t364 = ct{1446};
t365 = ct{1447};
t366 = ct{1448};
t368 = ct{1449};
t369 = ct{1450};
t370 = ct{1451};
t371 = ct{1452};
t372 = ct{1453};
t373 = ct{1454};
t377 = ct{1455};
t378 = ct{1456};
t38 = ct{1457};
t380 = ct{1458};
t381 = ct{1459};
t382 = ct{1460};
t385 = ct{1461};
t386 = ct{1462};
t387 = ct{1463};
t388 = ct{1464};
t389 = ct{1465};
t39 = ct{1466};
t391 = ct{1467};
t392 = ct{1468};
t393 = ct{1469};
t396 = ct{1470};
t3974 = ct{1471};
t3995 = ct{1472};
t404 = ct{1473};
t406 = ct{1474};
t408 = ct{1475};
t410 = ct{1476};
t411 = ct{1477};
t412 = ct{1478};
t413 = ct{1479};
t414 = ct{1480};
t419 = ct{1481};
t42 = ct{1482};
t420 = ct{1483};
t421 = ct{1484};
t422 = ct{1485};
t424 = ct{1486};
t425 = ct{1487};
t426 = ct{1488};
t4260 = ct{1489};
t428 = ct{1490};
t429 = ct{1491};
t43 = ct{1492};
t430 = ct{1493};
t432 = ct{1494};
t4325 = ct{1495};
t434 = ct{1496};
t4343 = ct{1497};
t435 = ct{1498};
t437 = ct{1499};
t438 = ct{1500};
t439 = ct{1501};
t444 = ct{1502};
t445 = ct{1503};
t448 = ct{1504};
t451 = ct{1505};
t452 = ct{1506};
t455 = ct{1507};
t456 = ct{1508};
t457 = ct{1509};
t458 = ct{1510};
t459 = ct{1511};
t46 = ct{1512};
t461 = ct{1513};
t463 = ct{1514};
t464 = ct{1515};
t465 = ct{1516};
t466 = ct{1517};
t467 = ct{1518};
t468 = ct{1519};
t469 = ct{1520};
t47 = ct{1521};
t4705 = ct{1522};
t471 = ct{1523};
t473 = ct{1524};
t474 = ct{1525};
t476 = ct{1526};
t478 = ct{1527};
t479 = ct{1528};
t480 = ct{1529};
t483 = ct{1530};
t485 = ct{1531};
t486 = ct{1532};
t488 = ct{1533};
t489 = ct{1534};
t49 = ct{1535};
t490 = ct{1536};
t491 = ct{1537};
t493 = ct{1538};
t494 = ct{1539};
t495 = ct{1540};
t496 = ct{1541};
t497 = ct{1542};
t498 = ct{1543};
t50 = ct{1544};
t503 = ct{1545};
t504 = ct{1546};
t506 = ct{1547};
t507 = ct{1548};
t508 = ct{1549};
t509 = ct{1550};
t510 = ct{1551};
t511 = ct{1552};
t512 = ct{1553};
t513 = ct{1554};
t514 = ct{1555};
t516 = ct{1556};
t517 = ct{1557};
t518 = ct{1558};
t521 = ct{1559};
t522 = ct{1560};
t523 = ct{1561};
t524 = ct{1562};
t525 = ct{1563};
t526 = ct{1564};
t527 = ct{1565};
t528 = ct{1566};
t53 = ct{1567};
t530 = ct{1568};
t531 = ct{1569};
t536 = ct{1570};
t538 = ct{1571};
t539 = ct{1572};
t54 = ct{1573};
t540 = ct{1574};
t542 = ct{1575};
t543 = ct{1576};
t544 = ct{1577};
t546 = ct{1578};
t547 = ct{1579};
t550 = ct{1580};
t551 = ct{1581};
t552 = ct{1582};
t553 = ct{1583};
t556 = ct{1584};
t56 = ct{1585};
t562 = ct{1586};
t563 = ct{1587};
t565 = ct{1588};
t568 = ct{1589};
t569 = ct{1590};
t571 = ct{1591};
t572 = ct{1592};
t573 = ct{1593};
t574 = ct{1594};
t575 = ct{1595};
t576 = ct{1596};
t577 = ct{1597};
t578 = ct{1598};
t58 = ct{1599};
t580 = ct{1600};
t582 = ct{1601};
t583 = ct{1602};
t584 = ct{1603};
t585 = ct{1604};
t589 = ct{1605};
t59 = ct{1606};
t590 = ct{1607};
t592 = ct{1608};
t597 = ct{1609};
t60 = ct{1610};
t600 = ct{1611};
t601 = ct{1612};
t605 = ct{1613};
t606 = ct{1614};
t607 = ct{1615};
t608 = ct{1616};
t609 = ct{1617};
t610 = ct{1618};
t611 = ct{1619};
t612 = ct{1620};
t614 = ct{1621};
t615 = ct{1622};
t616 = ct{1623};
t618 = ct{1624};
t620 = ct{1625};
t621 = ct{1626};
t622 = ct{1627};
t623 = ct{1628};
t624 = ct{1629};
t625 = ct{1630};
t627 = ct{1631};
t628 = ct{1632};
t629 = ct{1633};
t63 = ct{1634};
t631 = ct{1635};
t634 = ct{1636};
t635 = ct{1637};
t636 = ct{1638};
t638 = ct{1639};
t640 = ct{1640};
t641 = ct{1641};
t642 = ct{1642};
t643 = ct{1643};
t645 = ct{1644};
t646 = ct{1645};
t648 = ct{1646};
t649 = ct{1647};
t650 = ct{1648};
t651 = ct{1649};
t652 = ct{1650};
t654 = ct{1651};
t655 = ct{1652};
t656 = ct{1653};
t657 = ct{1654};
t658 = ct{1655};
t659 = ct{1656};
t660 = ct{1657};
t662 = ct{1658};
t663 = ct{1659};
t664 = ct{1660};
t665 = ct{1661};
t666 = ct{1662};
t667 = ct{1663};
t668 = ct{1664};
t669 = ct{1665};
t67 = ct{1666};
t670 = ct{1667};
t672 = ct{1668};
t673 = ct{1669};
t674 = ct{1670};
t675 = ct{1671};
t676 = ct{1672};
t677 = ct{1673};
t678 = ct{1674};
t679 = ct{1675};
t68 = ct{1676};
t681 = ct{1677};
t682 = ct{1678};
t683 = ct{1679};
t684 = ct{1680};
t685 = ct{1681};
t686 = ct{1682};
t687 = ct{1683};
t689 = ct{1684};
t691 = ct{1685};
t692 = ct{1686};
t693 = ct{1687};
t694 = ct{1688};
t696 = ct{1689};
t698 = ct{1690};
t70 = ct{1691};
t701 = ct{1692};
t702 = ct{1693};
t704 = ct{1694};
t705 = ct{1695};
t707 = ct{1696};
t708 = ct{1697};
t71 = ct{1698};
t710 = ct{1699};
t711 = ct{1700};
t712 = ct{1701};
t713 = ct{1702};
t714 = ct{1703};
t715 = ct{1704};
t716 = ct{1705};
t717 = ct{1706};
t718 = ct{1707};
t719 = ct{1708};
t720 = ct{1709};
t721 = ct{1710};
t722 = ct{1711};
t723 = ct{1712};
t724 = ct{1713};
t725 = ct{1714};
t726 = ct{1715};
t728 = ct{1716};
t73 = ct{1717};
t733 = ct{1718};
t735 = ct{1719};
t736 = ct{1720};
t738 = ct{1721};
t739 = ct{1722};
t740 = ct{1723};
t741 = ct{1724};
t742 = ct{1725};
t743 = ct{1726};
t744 = ct{1727};
t745 = ct{1728};
t746 = ct{1729};
t747 = ct{1730};
t749 = ct{1731};
t750 = ct{1732};
t751 = ct{1733};
t755 = ct{1734};
t756 = ct{1735};
t757 = ct{1736};
t758 = ct{1737};
t759 = ct{1738};
t76 = ct{1739};
t762 = ct{1740};
t763 = ct{1741};
t764 = ct{1742};
t765 = ct{1743};
t766 = ct{1744};
t767 = ct{1745};
t768 = ct{1746};
t770 = ct{1747};
t771 = ct{1748};
t772 = ct{1749};
t773 = ct{1750};
t774 = ct{1751};
t775 = ct{1752};
t776 = ct{1753};
t777 = ct{1754};
t778 = ct{1755};
t78 = ct{1756};
t781 = ct{1757};
t782 = ct{1758};
t783 = ct{1759};
t784 = ct{1760};
t785 = ct{1761};
t786 = ct{1762};
t787 = ct{1763};
t789 = ct{1764};
t79 = ct{1765};
t790 = ct{1766};
t791 = ct{1767};
t792 = ct{1768};
t793 = ct{1769};
t794 = ct{1770};
t796 = ct{1771};
t797 = ct{1772};
t798 = ct{1773};
t799 = ct{1774};
t8 = ct{1775};
t800 = ct{1776};
t801 = ct{1777};
t802 = ct{1778};
t806 = ct{1779};
t807 = ct{1780};
t808 = ct{1781};
t809 = ct{1782};
t812 = ct{1783};
t813 = ct{1784};
t816 = ct{1785};
t817 = ct{1786};
t818 = ct{1787};
t819 = ct{1788};
t820 = ct{1789};
t821 = ct{1790};
t822 = ct{1791};
t823 = ct{1792};
t824 = ct{1793};
t825 = ct{1794};
t826 = ct{1795};
t827 = ct{1796};
t828 = ct{1797};
t829 = ct{1798};
t830 = ct{1799};
t831 = ct{1800};
t832 = ct{1801};
t833 = ct{1802};
t836 = ct{1803};
t837 = ct{1804};
t838 = ct{1805};
t839 = ct{1806};
t841 = ct{1807};
t844 = ct{1808};
t846 = ct{1809};
t850 = ct{1810};
t852 = ct{1811};
t853 = ct{1812};
t855 = ct{1813};
t856 = ct{1814};
t857 = ct{1815};
t858 = ct{1816};
t859 = ct{1817};
t860 = ct{1818};
t861 = ct{1819};
t863 = ct{1820};
t865 = ct{1821};
t866 = ct{1822};
t868 = ct{1823};
t869 = ct{1824};
t870 = ct{1825};
t871 = ct{1826};
t872 = ct{1827};
t874 = ct{1828};
t876 = ct{1829};
t877 = ct{1830};
t878 = ct{1831};
t881 = ct{1832};
t882 = ct{1833};
t883 = ct{1834};
t885 = ct{1835};
t887 = ct{1836};
t889 = ct{1837};
t89 = ct{1838};
t890 = ct{1839};
t891 = ct{1840};
t893 = ct{1841};
t894 = ct{1842};
t895 = ct{1843};
t896 = ct{1844};
t898 = ct{1845};
t9 = ct{1846};
t90 = ct{1847};
t900 = ct{1848};
t902 = ct{1849};
t903 = ct{1850};
t904 = ct{1851};
t905 = ct{1852};
t906 = ct{1853};
t907 = ct{1854};
t908 = ct{1855};
t91 = ct{1856};
t911 = ct{1857};
t912 = ct{1858};
t914 = ct{1859};
t915 = ct{1860};
t916 = ct{1861};
t917 = ct{1862};
t918 = ct{1863};
t92 = ct{1864};
t921 = ct{1865};
t924 = ct{1866};
t926 = ct{1867};
t927 = ct{1868};
t930 = ct{1869};
t932 = ct{1870};
t933 = ct{1871};
t934 = ct{1872};
t935 = ct{1873};
t936 = ct{1874};
t937 = ct{1875};
t94 = ct{1876};
t940 = ct{1877};
t942 = ct{1878};
t943 = ct{1879};
t944 = ct{1880};
t945 = ct{1881};
t947 = ct{1882};
t948 = ct{1883};
t950 = ct{1884};
t951 = ct{1885};
t956 = ct{1886};
t959 = ct{1887};
t960 = ct{1888};
t961 = ct{1889};
t962 = ct{1890};
t965 = ct{1891};
t966 = ct{1892};
t967 = ct{1893};
t969 = ct{1894};
t97 = ct{1895};
t970 = ct{1896};
t974 = ct{1897};
t976 = ct{1898};
t978 = ct{1899};
t981 = ct{1900};
t983 = ct{1901};
t985 = ct{1902};
t987 = ct{1903};
t989 = ct{1904};
t99 = ct{1905};
t990 = ct{1906};
t992 = ct{1907};
t993 = ct{1908};
t994 = ct{1909};
t995 = ct{1910};
t996 = ct{1911};
t997 = ct{1912};
t998 = ct{1913};
t999 = ct{1914};
t4762 = t144+t153+t170+t180+t368+t386+t392+t408+t424+t425+t434+t459+t839+t841+t853+t863+t1080+t1148+t1167+t1178+t1179+t1180+t1204+t1234;
t4763 = t150+t156+t168+t178+t355+t385+t391+t396+t404+t406+t432+t457+t838+t844+t852+t861+t1112+t1145+t1177+t1185+t1198+t1199+t1203+t1232;
t5025 = t149+t158+t177+t192+t198+t212+t221+t388+t420+t435+t451+t467+t476+t483+t837+t846+t869+t877+t890+t898+t903+t1092+t1192+t1246+t1252+t1267+t1294+t1297;
t5027 = t148+t165+t174+t186+t207+t209+t218+t377+t419+t448+t452+t464+t495+t496+t836+t857+t866+t883+t889+t896+t900+t1137+t1189+t1229+t1247+t1265+t1278+t1280;
t141 = t47+t49;
t300 = t292.^2;
t347 = -t335;
t535 = -t523;
t549 = -t536;
t564 = -t542;
t579 = -t551;
t581 = -t556;
t587 = -t565;
t593 = -t571;
t594 = -t577;
t598 = -t578;
t644 = -t611;
t680 = -t651;
t925 = -t907;
t941 = t188+t268;
t949 = -t944;
t991 = t948.^2;
t1004 = (t140.*t262)./9.007199254740992e+15;
t1005 = (t140.*t264)./9.007199254740992e+15;
t1022 = t999.^2;
t1033 = t27.*t992;
t1034 = t27.*t993;
t1036 = -t1015;
t1037 = t27.*t995;
t1040 = -t1020;
t1043 = -t1024;
t1053 = -t1038;
t1054 = -t1041;
t1060 = -t1046;
t1063 = -t1051;
t1064 = -t1052;
t1068 = -t1059;
t1069 = -t1062;
t1077 = t8.*t9.*t1041;
t1078 = t8.*t14.*t1041;
t1079 = t9.*t13.*t1041;
t1081 = t13.*t14.*t1041;
t1085 = t8.*t9.*t1028;
t1086 = t8.*t14.*t1028;
t1087 = t9.*t13.*t1028;
t1088 = t13.*t14.*t1028;
t1093 = -t1072;
t1097 = -t1073;
t1127 = t8.*t14.*t1059;
t1128 = t9.*t13.*t1059;
t1130 = -t1090;
t1131 = -t1091;
t1133 = -t1094;
t1134 = t13.*t14.*t1059;
t1136 = -t1095;
t1151 = -t1102;
t1152 = -t1106;
t1153 = -t1107;
t1156 = -t1117;
t1160 = -t1122;
t1163 = t8.*t9.*t1059;
t1164 = -t1132;
t1169 = -t1141;
t1172 = -t1146;
t1173 = -t1147;
t1175 = -t1149;
t1200 = -t1186;
t1211 = -t1188;
t1442 = t337+t348;
t1465 = t27.*t1431;
t1466 = t27.*t1432;
t1467 = t27.*t1439;
t1472 = -t1459;
t1476 = -t1468;
t1502 = -t1486;
t1508 = -t1499;
t1534 = -t1525;
t1540 = -t1532;
t1548 = -t1544;
t1553 = -t1547;
t1557 = -t1552;
t1564 = -t1559;
t1580 = t140.*t264.*6.489053738789607e-19;
t1597 = t140.*t264.*7.194245199571015e-21;
t1603 = -t1588;
t1610 = -t1594;
t1630 = t140.*t262.*7.183142969324763e-22;
t1632 = -t1618;
t1647 = -t1620;
t1709 = -t1633;
t1713 = -t1635;
t1714 = -t1636;
t1715 = -t1637;
t1718 = -t1643;
t1719 = -t1650;
t1720 = -t1651;
t1721 = -t1652;
t1722 = -t1653;
t1723 = -t1654;
t1724 = -t1664;
t1725 = -t1665;
t1726 = -t1666;
t1727 = -t1667;
t1728 = -t1668;
t1729 = -t1671;
t1730 = -t1672;
t1731 = -t1673;
t1732 = -t1674;
t1733 = -t1676;
t1734 = -t1678;
t1735 = -t1681;
t1736 = -t1682;
t1737 = -t1683;
t1744 = -t1691;
t1746 = -t1692;
t1747 = -t1693;
t1748 = -t1694;
t1755 = -t1705;
t1763 = -t1716;
t1767 = -t1739;
t1774 = -t1745;
t1778 = -t1749;
t1781 = -t1756;
t1783 = -t1757;
t1784 = -t1758;
t1785 = -t1759;
t1787 = -t1771;
t1788 = -t1772;
t1789 = -t1773;
t1790 = -t1775;
t1791 = -t1776;
t1792 = -t1777;
t1803 = -t1799;
t1804 = t18.*t19.*t1743;
t1805 = t18.*t25.*t1743;
t1806 = t19.*t24.*t1743;
t1808 = t24.*t25.*t1743;
t1809 = t18.*t19.*t1749;
t1811 = t18.*t25.*t1749;
t1812 = t19.*t24.*t1749;
t1815 = t24.*t25.*t1749;
t1818 = -t1802;
t1833 = -t1810;
t1838 = -t1813;
t1839 = -t1814;
t1846 = -t1826;
t1847 = -t1827;
t1848 = -t1828;
t1849 = -t1829;
t1852 = -t1834;
t1853 = -t1835;
t1854 = -t1836;
t1855 = -t1840;
t1857 = -t1842;
t1859 = -t1843;
t1864 = -t1861;
t1867 = -t1862;
t1869 = -t1866;
t1893 = (t20.*t50.*t140.*t202)./8.112963841460668e+31;
t1896 = (t26.*t50.*t140.*t202)./8.112963841460668e+31;
t2125 = t140.*t264.*1.875105520197095e-20;
t2132 = t35.*t2113;
t2133 = t35.*t2114;
t2134 = t36.*t2113;
t2135 = t36.*t2114;
t2137 = t140.*t264.*7.825108561121397e-23;
t2142 = t140.*t262.*2.075672598245148e-23;
t2143 = -t2136;
t2163 = -t2148;
t2170 = t38.*t2115;
t2171 = t38.*t2116;
t2172 = t39.*t2115;
t2173 = t39.*t2116;
t2202 = -t2175;
t2208 = -t2183;
t2216 = -t2185;
t2237 = -t2186;
t2242 = -t2188;
t2243 = -t2189;
t2248 = -t2193;
t2254 = -t2196;
t2258 = -t2197;
t2262 = -t2199;
t2264 = -t2204;
t2265 = -t2205;
t2266 = -t2206;
t2267 = -t2212;
t2268 = -t2213;
t2269 = -t2214;
t2270 = -t2219;
t2271 = -t2220;
t2272 = -t2221;
t2273 = -t2225;
t2274 = -t2226;
t2275 = -t2228;
t2276 = -t2231;
t2277 = -t2235;
t2278 = -t2236;
t2279 = -t2239;
t2280 = -t2240;
t2281 = -t2244;
t2282 = -t2245;
t2283 = -t2246;
t2284 = -t2247;
t2285 = -t2250;
t2286 = -t2251;
t2287 = -t2252;
t2288 = -t2253;
t2289 = -t2255;
t2293 = -t2290;
t2298 = -t2292;
t2301 = -t2295;
t2307 = t237+t1469;
t2312 = -t2304;
t2321 = t513+t872;
t2335 = t12.*t2297;
t2337 = t17.*t2297;
t2338 = t512+t887;
t2342 = t20.*t50.*t140.*t202.*7.204296868834178e-35;
t2344 = t26.*t50.*t140.*t202.*7.204296868834178e-35;
t2368 = t20.*t50.*t140.*t202.*7.987216665362745e-37;
t2371 = t26.*t50.*t140.*t202.*7.987216665362745e-37;
t2388 = t262+t1484;
t2399 = t518+t891;
t2419 = t517+t904;
t2421 = t20.*t50.*t140.*t202.*7.974890713718666e-38;
t2423 = t26.*t50.*t140.*t202.*7.974890713718666e-38;
t2465 = t22.*t2363;
t2468 = t28.*t2363;
t2470 = t16.*t2297.*(3.0./5.0e+2);
t2500 = t140.*t188.*t201.*2.442490654175345e-23;
t2507 = t140.*t189.*t202.*2.442490654175345e-23;
t2534 = -t2530;
t2535 = t27.*t2363.*(3.0./5.0e+2);
t2538 = t38.*t50.*t292.*6.209141233430105e-19i;
t2539 = t39.*t50.*t292.*6.209141233430105e-19i;
t2554 = (t11.*t2297)./1.0e+8;
t2576 = t39.*t50.*t292.*3.200438707086705e-18i;
t2637 = t38.*t50.*t292.*3.200438707086705e-18i;
t2670 = t35.*t236.*t291.*2.79634861451666e-3;
t2671 = t36.*t236.*t291.*2.79634861451666e-3;
t2678 = t35.*t236.*t291.*1.44134945686578e-2;
t2680 = t36.*t236.*t291.*1.44134945686578e-2;
t2706 = t859+t874;
t2722 = t865+t878;
t2732 = t20.*t50.*t140.*t202.*2.081785322124547e-36;
t2733 = t26.*t50.*t140.*t202.*2.081785322124547e-36;
t2743 = t11.*t2297.*1.247162e-2;
t2744 = t26.*t50.*t140.*t202.*8.687615694748404e-39;
t2757 = t20.*t50.*t140.*t202.*8.687615694748404e-39;
t2758 = t16.*t2297.*5.68686e-3;
t2765 = t20.*t50.*t140.*t202.*2.304459510155286e-39;
t2767 = t26.*t50.*t140.*t202.*2.304459510155286e-39;
t2793 = t16.*t2297.*3.131399999999998e-4;
t2801 = t16.*t2297.*5.7e-7;
t2831 = t11.*t2297.*2.4e-7;
t2832 = t21.*t2363.*1.247162e-2;
t2849 = t27.*t2363.*5.68686e-3;
t2850 = t11.*t2297.*4.0e-8;
t2851 = t16.*t2297.*4.0e-8;
t2909 = t27.*t2363.*3.131399999999998e-4;
t2924 = t38.*t50.*t292.*4.512400254276827e-21i;
t2927 = t39.*t50.*t292.*4.512400254276827e-21i;
t2939 = t38.*t50.*t292.*2.325870823794656e-20i;
t2940 = t39.*t50.*t292.*2.325870823794656e-20i;
t2958 = t50.*t140.*t188.*t202.*2.711709361697228e-39;
t2971 = t526+t1871;
t2972 = t997+t1483;
t2973 = t525+t1878;
t2974 = t35.*t50.*t236.*t291.*3.104570616715053e-19i;
t2975 = t36.*t50.*t236.*t291.*3.104570616715053e-19i;
t2976 = t574+t1921;
t2979 = t35.*t50.*t236.*t291.*1.600219353543352e-18i;
t2980 = t36.*t50.*t236.*t291.*1.600219353543352e-18i;
t2981 = t569+t1938;
t2988 = t318+t323+t1403;
t2989 = t315+t320+t325+t361;
t2990 = (t1403.*t1535)./2.0;
t2993 = t201.*t2297.*8.595599785252598e-9;
t3017 = t201.*t2297.*5.329271866856611e-7;
t3018 = t201.*t2297.*2.784974330421842e-6;
t3019 = t201.*t2297.*6.730354631852784e-6;
t3049 = t50.*t202.*t2297.*9.543032792050485e-25;
t3064 = t50.*t202.*t2297.*9.390344267377678e-22;
t3066 = t50.*t202.*t2297.*5.916680331071301e-23;
t3070 = t50.*t202.*t2297.*3.091942624624357e-22;
t3071 = t50.*t202.*t2297.*7.472194676175529e-22;
t3080 = t11.*t50.*t202.*t2297.*9.733893447891495e-23;
t3081 = t16.*t50.*t202.*t2297.*5.439528691468777e-23;
t3084 = t11.*t50.*t202.*t2297.*2.290327870092116e-23;
t3086 = t11.*t50.*t202.*t2297.*3.817213116820194e-24;
t3087 = t16.*t50.*t202.*t2297.*3.817213116820194e-24;
t3130 = (t2297.*t2363)./1.0e+8;
t3154 = t2297.*t2363.*6.2e-7;
t3155 = t576+t1898+t1932;
t3160 = t11.*t2297.*t2363.*1.02e-6;
t3166 = t572+t1917+t1944;
t3172 = t11.*t2297.*t2363.*(-4.0e-8);
t3173 = t16.*t2297.*t2363.*(-4.0e-8);
t3313 = t38.*t947.*t999.*t2718.*4.392651260556773e-1;
t3315 = t39.*t947.*t999.*t2718.*4.392651260556773e-1;
t3320 = t540+t552+t1914+t1920;
t3327 = t1017+t1057+t1480+t1531;
t3381 = t38.*t947.*t999.*t2718.*2.244797987218524e-1;
t3382 = t39.*t947.*t999.*t2718.*2.244797987218524e-1;
t3384 = t38.*t947.*t999.*t2718.*3.775747223193135e-1;
t3385 = t39.*t947.*t999.*t2718.*3.775747223193135e-1;
t3390 = t38.*t947.*t999.*t2718.*1.015213745795343e-2;
t3391 = t39.*t947.*t999.*t2718.*1.015213745795343e-2;
t3470 = t38.*t947.*t999.*t2718.*2.933606309255039e-4;
t3471 = t39.*t947.*t999.*t2718.*2.933606309255039e-4;
t3523 = t1622+t1766+t1960+t2078;
t3533 = t1100+t1118+t2452+t2482;
t3638 = t524+t575+t1885+t1886+t1957;
t3649 = t543+t610+t1892+t1927+t1998;
t3767 = t1001+t1025+t1031+t1042+t1497+t1509;
t3806 = t2314+t2331+t2332+t2333;
t3807 = t2315+t2316+t2334+t2347;
t3837 = t2723+t2728+t2729+t2731;
t3838 = t2724+t2725+t2730+t2734;
t3875 = t1624+t1669+t1740+t1751+t2056+t2077;
t3876 = t592+t600+t601+t608+t1560+t1570+t1571+t1572;
t3877 = t589+t590+t597+t621+t1567+t1568+t1569+t1583;
t3878 = t584+t585+t607+t622+t1560+t1570+t1571+t1572;
t3879 = t583+t605+t606+t609+t1567+t1568+t1569+t1583;
t4035 = t204+t260+t272+t491+t507+t509+t912+t960+t967+t1304+t1460+t1463;
t4104 = t225+t229+t439+t458+t486+t489+t932+t935+t1264+t1272+t1326+t1422;
t4147 = t1110+t1123+t1124+t1150+t2118+t2119+t2121+t2129;
t4150 = t1104+t1105+t1121+t1126+t2117+t2126+t2127+t2128;
t4153 = t1113+t1114+t1162+t1176+t2118+t2119+t2121+t2129;
t4154 = t1108+t1154+t1158+t1159+t2117+t2126+t2127+t2128;
t4314 = t54+t113+t114+t121+t133+t138+t273+t301+t303+t546+t631+t634+t652+t739+t765+t985+t1029+t1032;
t4327 = t63+t78+t79+t94+t106+t127+t267+t270+t285+t297+t531+t550+t553+t568+t582+t620+t921+t924+t956+t976;
t4334 = t162+t176+t197+t227+t421+t426+t485+t497+t871+t895+t918+t934+t1224+t1262+t1325+t1353;
t4338 = t185+t191+t211+t242+t465+t468+t478+t494+t876+t882+t902+t906+t1248+t1253+t1277+t1296;
t4476 = t1292+t1334+t1402+t1443+t1445+t1446+t1479+t1482+t1796+t1800+t1807+t1817;
t4563 = t547+t905+t908+t1055+t1061+t1066+t1070+t1491+t1523+t1528+t1530+t1533+t1541+t1542;
t4683 = t860+t1255+t1281+t1298+t1401+t1413+t1426+t1430+t1695+t1765+t1793+t1794+t1795+t1797;
t4716 = t53+t103+t109+t110+t111+t120+t132+t136+t275+t283+t295+t309+t311+t527+t544+t618+t625+t627+t629+t650+t701+t735+t970+t981+t994+t1009+t1014+3.064357668490995e+34;
t4847 = t161+t172+t196+t226+t373+t412+t414+t422+t437+t438+t469+t490+t870+t885+t917+t933+t1187+t1209+t1251+t1263+t1270+t1271+t1332+t1423;
t4850 = t160+t173+t195+t223+t389+t411+t413+t445+t455+t456+t466+t488+t868+t894+t916+t930+t1174+t1206+t1241+t1245+t1260+t1261+t1330+t1418;
t5036 = t152+t167+t205+t217+t243+t263+t274+t381+t430+t471+t479+t493+t508+t511+t858+t881+t914+t927+t943+t962+t969+t1213+t1268+t1310+t1383+t1437+t1451+t1461;
et1 = t236.*t241.*t4705.*(t208-t225-t439+t444+t463-t489+t915+t1259+t1364-t20.*t21.*t28.*t240.*1.075008113939401e+50-t27.*t28.*t50.*t240.*1.025883768304404e+34i-t21.*t22.*t26.*t50.*t240.*3.315051378778914e+33i);
et2 = -2.394182569460511e-91;
t5296 = et1.*et2;
et3 = t236.*t241.*t4705.*(t208-t225-t439+t444+t463-t489+t915+t1259+t1364-t20.*t21.*t28.*t240.*1.075008113939401e+50-t27.*t28.*t50.*t240.*1.025883768304404e+34i-t21.*t22.*t26.*t50.*t240.*3.315051378778914e+33i);
et4 = 2.394182569460511e-91;
t5299 = et3.*et4;
et5 = t236.*t241.*t4763.*(t208-t225-t439+t444+t463-t489+t915+t1259+t1364-t20.*t21.*t28.*t240.*1.075008113939401e+50-t27.*t28.*t50.*t240.*1.025883768304404e+34i-t21.*t22.*t26.*t50.*t240.*3.315051378778914e+33i);
et6 = -2.658076613771277e-107;
t5370 = et5.*et6;
et7 = t236.*t241.*t5025.*(t208-t225-t439+t444+t463-t489+t915+t1259+t1364-t20.*t21.*t28.*t240.*1.075008113939401e+50-t27.*t28.*t50.*t240.*1.025883768304404e+34i-t21.*t22.*t26.*t50.*t240.*3.315051378778914e+33i);
et8 = -1.297888971568006e-110;
t5437 = et7.*et8;
t1026 = -t1005;
t1598 = -t1580;
t1612 = -t1597;
t1703 = -t1630;
t1912 = -t1896;
t2350 = t11.*t2307;
t2351 = t12.*t2307;
t2355 = t16.*t2307;
t2356 = t17.*t2307;
t2369 = -t2342;
t2373 = t16.*t2335;
t2376 = t16.*t2337;
t2381 = -t2337;
t2387 = t11.*t2321;
t2390 = t16.*t2321;
t2397 = -t2368;
t2400 = -t2371;
t2410 = t12.*t2338;
t2412 = t17.*t2338;
t2496 = t21.*t2388;
t2497 = t22.*t2388;
t2502 = t27.*t2388;
t2503 = t28.*t2388;
t2517 = -t2500;
t2521 = t21.*t2399;
t2522 = t27.*t2399;
t2526 = t27.*t2465;
t2527 = t22.*t2419;
t2528 = t27.*t2468;
t2531 = t28.*t2419;
t2575 = -t2538;
t2638 = -t2576;
t2664 = -t2637;
t2672 = t2132.*5.110348748545983e-1;
t2673 = -t2670;
t2674 = t2134.*5.110348748545983e-1;
t2675 = -t2671;
t2676 = t2133.*8.595599785252598e-1;
t2679 = t2135.*8.595599785252598e-1;
t2681 = t2132.*2.311164e-2;
t2682 = t2134.*2.311164e-2;
t2683 = -t2678;
t2684 = t2133.*1.273194e-2;
t2685 = -t2680;
t2686 = t2132.*4.251385e-2;
t2687 = t2135.*1.273194e-2;
t2688 = t2134.*4.251385e-2;
t2691 = t2170.*5.110348748545983e-1;
t2692 = t2132.*6.562549e-2;
t2694 = t2172.*5.110348748545983e-1;
t2695 = t2134.*6.562549e-2;
t2697 = t38.*t241.*t300.*2.79634861451666e-3;
t2698 = t39.*t241.*t300.*2.79634861451666e-3;
t2701 = t2171.*8.595599785252598e-1;
t2703 = t2173.*8.595599785252598e-1;
t2707 = t2171.*1.273194e-2;
t2708 = t2170.*4.251385e-2;
t2709 = t2173.*1.273194e-2;
t2710 = t2172.*4.251385e-2;
t2711 = t38.*t241.*t300.*1.44134945686578e-2;
t2712 = t39.*t241.*t300.*1.44134945686578e-2;
t2714 = t2170.*6.562549e-2;
t2716 = t2172.*6.562549e-2;
t2737 = t2335.*9.99471e-3;
t2738 = t2337.*9.99471e-3;
t2739 = t2335.*1.838876e-2;
t2740 = t2337.*1.838876e-2;
t2771 = -t2758;
t2791 = -t2767;
t2804 = t2335.*9.3e-7;
t2806 = t2335.*1.02e-6;
t2810 = t2337.*9.3e-7;
t2813 = t2337.*1.02e-6;
t2817 = t2465.*9.99471e-3;
t2818 = t2468.*9.99471e-3;
t2819 = t2465.*1.838876e-2;
t2820 = t2468.*1.838876e-2;
t2825 = -t2801;
t2835 = t2335.*9.0e-8;
t2838 = t2337.*9.0e-8;
t2870 = -t2849;
t2875 = -t2851;
t2937 = -t2924;
t2941 = -t2939;
t2942 = -t2940;
t2943 = t38.*t241.*t300.*2.032204410370765e-5;
t2944 = t39.*t241.*t300.*2.032204410370765e-5;
t2947 = t2170.*6.678441185616e-4;
t2948 = t2172.*6.678441185616e-4;
t2949 = t2171.*9.2527464159e-5;
t2950 = t2173.*9.2527464159e-5;
t2951 = t38.*t241.*t300.*1.047479097535352e-4;
t2952 = t39.*t241.*t300.*1.047479097535352e-4;
t2955 = t2170.*4.769234047515e-4;
t2956 = t2172.*4.769234047515e-4;
t2961 = -t2958;
t2977 = -t2974;
t2978 = -t2975;
t2982 = -t2980;
t2983 = t39.*t50.*t241.*t300.*3.104570616715053e-19i;
t2984 = t38.*t50.*t241.*t300.*3.104570616715053e-19i;
t2986 = t38.*t50.*t241.*t300.*1.600219353543352e-18i;
t2987 = t39.*t50.*t241.*t300.*1.600219353543352e-18i;
t2991 = (t1442.*t1536)./2.0;
t2999 = t35.*t941.*t991.*2.196325630278387e-1;
t3000 = t36.*t941.*t991.*2.196325630278387e-1;
t3004 = t38.*t50.*t241.*t300.*2.256200127138414e-21i;
t3005 = t39.*t50.*t241.*t300.*2.256200127138414e-21i;
t3008 = t39.*t50.*t241.*t300.*1.162935411897328e-20i;
t3010 = t38.*t50.*t241.*t300.*1.162935411897328e-20i;
t3011 = t39.*t947.*t1022.*2.196325630278387e-1;
t3012 = t38.*t947.*t1022.*2.196325630278387e-1;
t3015 = t201.*t2307.*8.458070188688557e-6;
t3022 = t35.*t941.*t991.*1.122398993609262e-1;
t3023 = t36.*t941.*t991.*1.122398993609262e-1;
t3026 = t35.*t941.*t991.*1.887873611596568e-1;
t3027 = t36.*t941.*t991.*1.887873611596568e-1;
t3029 = t35.*t941.*t991.*5.076068728976717e-3;
t3030 = t36.*t941.*t991.*5.076068728976717e-3;
t3036 = t38.*t947.*t1022.*1.122398993609262e-1;
t3037 = t39.*t947.*t1022.*1.122398993609262e-1;
t3042 = t38.*t947.*t1022.*1.887873611596568e-1;
t3043 = t39.*t947.*t1022.*1.887873611596568e-1;
t3044 = t38.*t947.*t1022.*5.076068728976717e-3;
t3045 = t39.*t947.*t1022.*5.076068728976717e-3;
t3050 = t50.*t202.*t2307.*9.543032792050485e-25;
t3051 = t11.*t3049;
t3054 = t50.*t202.*t2338.*9.543032792050485e-25;
t3057 = (t410.*t2989)./2.0;
t3058 = (t429.*t2988)./2.0;
t3065 = t50.*t202.*t2307.*9.390344267377678e-22;
t3067 = t50.*t202.*t2307.*5.916680331071301e-23;
t3068 = t50.*t202.*t2321.*9.390344267377678e-22;
t3069 = t38.*t947.*t1022.*1.46680315462752e-4;
t3072 = t39.*t947.*t1022.*1.46680315462752e-4;
t3074 = t50.*t202.*t2307.*3.091942624624357e-22;
t3075 = -t3070;
t3076 = t50.*t202.*t2307.*7.472194676175529e-22;
t3077 = -t3071;
t3079 = t50.*t202.*t2338.*5.916680331071301e-23;
t3082 = t50.*t202.*t2338.*3.091942624624357e-22;
t3083 = t50.*t202.*t2338.*7.472194676175529e-22;
t3085 = -t3081;
t3088 = -t3084;
t3119 = t1039+t1064+t1520;
t3120 = t1030+t1069+t1518;
tau_c = ft_6({dq1,dq2,dq3,dq4,dq5,dq6,t10,t100,t1000,t1002,t1003,t1004,t1005,t1006,t101,t1011,t1015,t1018,t1019,t1020,t1021,t1022,t1023,t1024,t1026,t1028,t1033,t1034,t1035,t1036,t1037,t1038,t1040,t1043,t1044,t1045,t1046,t1048,t1049,t1050,t1051,t1053,t1054,t1056,t1057,t1058,t1059,t1060,t1063,t1065,t1067,t1068,t107,t1071,t1072,t1074,t1075,t1076,t1077,t1078,t1079,t108,t1083,t1084,t1088,t1089,t1093,t1097,t1098,t1099,t11,t1103,t1104,t1105,t1108,t1109,t1111,t1115,t1116,t1119,t1120,t1121,t1125,t1127,t1128,t1129,t1130,t1131,t1133,t1135,t1136,t1138,t1139,t1140,t1142,t1144,t1151,t1152,t1153,t1156,t1158,t1159,t1160,t1163,t1164,t1165,t1169,t1172,t1173,t1175,t1190,t1193,t1194,t1195,t1196,t12,t1200,t1205,t1207,t1208,t1210,t1211,t1212,t1214,t1217,t1218,t1219,t1220,t1221,t1222,t123,t1230,t1235,t1236,t1237,t1238,t124,t126,t1266,t128,t1285,t1286,t1287,t1288,t1289,t1290,t1299,t13,t130,t1300,t1301,t1302,t1303,t1305,t1307,t1311,t1316,t1317,t1319,t1320,t1322,t1323,t1324,t1328,t1331,t1335,t1336,t1337,t1338,t134,t1342,t1343,t1344,t1345,t1348,t1349,t1350,t1351,t1352,t1354,t1360,t1366,t1367,t1368,t1369,t1370,t1371,t1372,t1374,t1375,t1376,t1377,t1378,t1379,t1380,t1385,t1386,t1387,t1388,t1389,t139,t1392,t1393,t1394,t1395,t1396,t1397,t1398,t1399,t14,t140,t1404,t1405,t1406,t1407,t1408,t1409,t1410,t1411,t1412,t1414,t1415,t1416,t1417,t1419,t1420,t1421,t1424,t1425,t1427,t1428,t1429,t1431,t1432,t1433,t1434,t1435,t1436,t1439,t1440,t1441,t1444,t1447,t1448,t1453,t1456,t1457,t1458,t1462,t1464,t1465,t1466,t1467,t1471,t1472,t1476,t1477,t1478,t1481,t1485,t1487,t1488,t1489,t1490,t1492,t1493,t1494,t1495,t1498,t15,t1500,t1501,t1502,t1503,t1504,t1505,t1506,t1507,t1508,t151,t1510,t1512,t1513,t1514,t1515,t1516,t1517,t1519,t1522,t1526,t1527,t1529,t1531,t1534,t1537,t1538,t1539,t1540,t1543,t1544,t1545,t1546,t1547,t1548,t1549,t1550,t1551,t1553,t1554,t1555,t1556,t1557,t1558,t1559,t1564,t1565,t1574,t1575,t1576,t1577,t1578,t1579,t1581,t1582,t1584,t1585,t1586,t1587,t1591,t1592,t1593,t1595,t1596,t1598,t1599,t16,t1600,t1601,t1602,t1603,t1604,t1605,t1606,t1607,t1608,t1609,t1610,t1612,t1613,t1614,t1615,t1616,t1619,t1621,t1625,t1626,t1627,t1628,t1629,t1631,t1632,t1634,t1637,t1639,t1640,t1641,t1642,t1644,t1645,t1646,t1647,t1648,t1649,t1655,t1656,t1657,t1658,t1659,t1660,t1661,t1662,t1663,t1666,t1667,t1670,t1675,t1677,t1679,t1680,t1683,t1684,t1685,t1686,t1687,t1690,t1692,t1696,t1697,t1698,t1699,t17,t1700,t1701,t1703,t1704,t1705,t1706,t1707,t1708,t1709,t1710,t1711,t1712,t1713,t1714,t1715,t1717,t1718,t1719,t1720,t1721,t1722,t1723,t1724,t1725,t1726,t1727,t1728,t1729,t1730,t1731,t1732,t1733,t1734,t1735,t1736,t1737,t1738,t1739,t1741,t1742,t1743,t1744,t1745,t1746,t1747,t1748,t1750,t1752,t1753,t1754,t1755,t1758,t1759,t1760,t1761,t1762,t1763,t1764,t1767,t1768,t1769,t1770,t1774,t1775,t1776,t1778,t1779,t1781,t1783,t1784,t1785,t1786,t1787,t1788,t1789,t1790,t1791,t1792,t18,t1801,t1803,t1808,t1809,t1811,t1812,t1816,t1818,t1819,t182,t1820,t1821,t1822,t1823,t1824,t1825,t1830,t1831,t1832,t1833,t1837,t1838,t1839,t1841,t1844,t1845,t1846,t1847,t1848,t1849,t1850,t1851,t1852,t1853,t1854,t1855,t1856,t1857,t1858,t1859,t1860,t1861,t1864,t1865,t1867,t1868,t1869,t1870,t1874,t1875,t1876,t1879,t188,t1880,t1881,t1882,t1883,t1884,t1886,t1887,t1888,t1889,t189,t1890,t1891,t1893,t1896,t19,t1900,t1901,t1902,t1903,t1904,t1905,t1906,t1909,t1910,t1911,t1912,t1913,t1918,t1923,t1924,t1925,t1926,t1927,t1929,t1930,t1931,t1933,t1934,t1935,t1936,t1937,t1939,t1940,t1941,t1943,t1945,t1946,t1948,t1951,t1952,t1953,t1954,t1955,t1956,t1957,t1958,t1959,t1961,t1962,t1963,t1964,t1966,t1967,t1969,t1971,t1972,t1973,t1978,t1979,t1980,t1981,t1983,t1984,t1985,t1988,t1990,t1991,t1992,t1993,t1994,t1997,t1998,t1999,t20,t2001,t2002,t2003,t2004,t2005,t2006,t2007,t2008,t2009,t201,t2010,t2013,t2014,t2015,t2016,t2017,t202,t2023,t2024,t2027,t2028,t2029,t203,t2030,t2031,t2032,t2033,t2034,t2035,t2036,t2037,t2039,t2040,t2041,t2042,t2043,t2044,t2045,t2049,t2050,t2051,t2052,t2053,t2054,t2057,t2058,t2059,t2060,t2061,t2062,t2063,t2064,t2065,t2066,t2067,t2068,t2069,t2070,t2071,t2072,t2073,t2074,t2075,t2079,t2081,t2082,t2083,t2084,t2085,t2086,t2087,t2089,t2090,t2091,t2093,t2094,t2095,t2098,t2099,t21,t2100,t2101,t2102,t2103,t2104,t2105,t2106,t2107,t2108,t2109,t2110,t2111,t2112,t2117,t2120,t2122,t2123,t2125,t2130,t2132,t2133,t2134,t2135,t2137,t2138,t2139,t2140,t2141,t2142,t2143,t2145,t2146,t2147,t2149,t2150,t2151,t2152,t2153,t2154,t2155,t2156,t2157,t2159,t216,t2160,t2161,t2162,t2163,t2164,t2165,t2166,t2167,t2168,t2169,t2170,t2171,t2172,t2173,t2174,t2176,t2177,t2178,t2179,t2180,t2181,t2182,t2183,t2184,t2187,t2190,t2191,t2192,t2193,t2194,t2195,t2198,t2199,t22,t2200,t2201,t2202,t2203,t2207,t2208,t2209,t2210,t2211,t2215,t2216,t2217,t2218,t2219,t2222,t2223,t2224,t2227,t2229,t2230,t2232,t2233,t2234,t2237,t2238,t2239,t2240,t2241,t2242,t2243,t2248,t2249,t2254,t2256,t2257,t2258,t2259,t2260,t2261,t2262,t2263,t2264,t2265,t2266,t2267,t2268,t2269,t2270,t2271,t2272,t2273,t2274,t2275,t2276,t2277,t2278,t2279,t2280,t2281,t2282,t2283,t2284,t2285,t2286,t2287,t2288,t2289,t2290,t2291,t2292,t2293,t2294,t2295,t2296,t2297,t2298,t2299,t230,t2300,t2301,t2302,t2303,t2304,t2305,t2306,t2307,t2308,t2309,t231,t2310,t2311,t2312,t2313,t2317,t2320,t2322,t2323,t2324,t2325,t2326,t2327,t2328,t2329,t2335,t2336,t2337,t2338,t2339,t2340,t2341,t2342,t2343,t2344,t2345,t2346,t2350,t2351,t2352,t2353,t2354,t2355,t2356,t2357,t2358,t2359,t236,t2360,t2361,t2362,t2363,t2364,t2365,t2366,t2367,t2368,t2369,t237,t2370,t2371,t2373,t2374,t2375,t2376,t2377,t2378,t2379,t238,t2380,t2381,t2382,t2384,t2385,t2386,t2387,t2388,t2389,t239,t2390,t2391,t2393,t2394,t2395,t2396,t2397,t2398,t2399,t24,t2400,t2401,t2402,t2403,t2404,t2405,t2408,t2409,t241,t2410,t2411,t2412,t2413,t2414,t2416,t2417,t2418,t2419,t2421,t2422,t2423,t2425,t2426,t2427,t2431,t2432,t2433,t2434,t2438,t2440,t2441,t2444,t2446,t2447,t2448,t2449,t2450,t2451,t2455,t2457,t2458,t2459,t2460,t2461,t2463,t2465,t2466,t2467,t2468,t2470,t2471,t2472,t2473,t2474,t2476,t2477,t2478,t2479,t2480,t2481,t2484,t2485,t2487,t2488,t2489,t2490,t2491,t2492,t2493,t2494,t2496,t2497,t2498,t2499,t25,t2500,t2502,t2503,t2504,t2505,t2507,t2508,t2509,t2510,t2511,t2512,t2514,t2515,t2516,t2517,t2520,t2521,t2522,t2524,t2525,t2526,t2527,t2528,t2529,t2530,t2531,t2532,t2534,t2535,t2539,t2541,t2542,t2548,t2549,t2550,t2552,t2554,t2555,t2556,t2557,t2558,t2559,t2560,t2564,t2565,t2566,t2569,t257,t2570,t2571,t2572,t2575,t2577,t2578,t2579,t2580,t2581,t2582,t2583,t2584,t2585,t2586,t2587,t2589,t259,t2595,t2597,t2599,t26,t2600,t2601,t2603,t2604,t2605,t2606,t261,t2610,t2611,t2612,t2613,t2614,t2616,t2618,t2619,t262,t2620,t2621,t2622,t2623,t2624,t2626,t2627,t2628,t2629,t2630,t2632,t2633,t2634,t2635,t2638,t264,t2640,t2641,t2642,t2643,t2644,t2645,t2646,t2647,t2648,t2649,t2650,t2651,t2652,t2653,t2654,t2655,t2657,t2658,t2659,t2660,t2661,t2662,t2664,t2665,t2666,t2667,t2668,t2670,t2671,t2672,t2673,t2674,t2675,t2676,t2678,t2679,t2680,t2681,t2682,t2683,t2684,t2685,t2686,t2687,t2688,t2691,t2692,t2694,t2695,t2697,t2698,t2699,t27,t2701,t2703,t2707,t2708,t2709,t271,t2710,t2711,t2712,t2714,t2716,t2732,t2733,t2735,t2736,t2737,t2738,t2739,t2740,t2742,t2743,t2744,t2745,t2748,t2749,t2750,t2753,t2754,t2757,t2759,t276,t2762,t2765,t2769,t2771,t2773,t2774,t2775,t2777,t2778,t2779,t2781,t2785,t2786,t2787,t2788,t279,t2790,t2791,t2792,t2793,t2795,t2796,t2797,t2798,t2799,t28,t280,t2801,t2802,t2803,t2804,t2805,t2806,t2807,t2808,t2810,t2811,t2812,t2813,t2814,t2817,t2818,t2819,t2820,t2823,t2825,t2831,t2832,t2835,t2838,t2850,t2851,t2857,t2858,t2859,t286,t2865,t2867,t2868,t2870,t2875,t2883,t2884,t2886,t2890,t2893,t2894,t2895,t2898,t29,t2900,t2901,t2903,t2905,t2909,t2911,t2914,t2917,t2918,t2919,t2920,t2922,t2923,t2925,t2926,t2927,t293,t2930,t2931,t2933,t2935,t2937,t2941,t2942,t2943,t2944,t2947,t2948,t2949,t2950,t2951,t2952,t2955,t2956,t2961,t2962,t2963,t2964,t2965,t2966,t2969,t2970,t2971,t2972,t2973,t2975,t2976,t2977,t2978,t2979,t2981,t2982,t2983,t2984,t2986,t2987,t2990,t2991,t2993,t2999,t30,t3000,t3004,t3005,t3008,t3010,t3011,t3012,t3015,t3017,t3018,t3019,t3022,t3023,t3026,t3027,t3029,t3030,t3036,t3037,t3042,t3043,t3044,t3045,t3049,t305,t3050,t3051,t3054,t3057,t3058,t306,t3064,t3065,t3066,t3067,t3068,t3069,t3072,t3074,t3075,t3076,t3077,t3079,t308,t3080,t3081,t3082,t3083,t3085,t3086,t3087,t3088,t31,t310,t3119,t312,t3120,t313,t3130,t314,t3154,t3155,t316,t3160,t3166,t3172,t3173,t319,t32,t321,t322,t326,t328,t329,t33,t330,t331,t3313,t3315,t332,t3320,t3327,t333,t335,t336,t338,t3381,t3382,t3384,t3385,t339,t3390,t3391,t34,t341,t343,t346,t347,t3470,t3471,t35,t350,t351,t352,t3523,t3533,t354,t356,t358,t359,t36,t360,t362,t363,t3638,t364,t3649,t365,t366,t369,t370,t371,t372,t3767,t378,t38,t380,t3806,t3807,t382,t3837,t3838,t387,t3875,t3876,t3877,t3878,t3879,t39,t393,t3974,t3995,t4035,t410,t4147,t4153,t4154,t42,t4260,t428,t429,t43,t4314,t4325,t4327,t4334,t4338,t4343,t4476,t4563,t46,t461,t4683,t47,t4705,t4716,t473,t474,t4762,t4763,t480,t4847,t4850,t498,t50,t5025,t5027,t503,t5036,t504,t506,t510,t514,t516,t521,t522,t523,t524,t528,t5296,t530,t535,t5370,t538,t539,t542,t543,t5437,t549,t56,t562,t563,t564,t573,t575,t577,t579,t58,t580,t581,t587,t59,t593,t594,t598,t60,t610,t611,t612,t614,t615,t616,t623,t624,t628,t635,t636,t638,t640,t641,t642,t643,t644,t645,t646,t648,t649,t654,t655,t656,t657,t658,t659,t660,t662,t663,t664,t665,t666,t667,t668,t669,t67,t670,t672,t673,t674,t675,t676,t677,t678,t679,t68,t680,t681,t682,t683,t684,t685,t686,t687,t689,t691,t692,t693,t694,t696,t698,t70,t702,t704,t705,t707,t708,t71,t710,t711,t712,t713,t714,t715,t716,t717,t718,t719,t720,t721,t722,t723,t724,t725,t726,t728,t73,t733,t736,t738,t740,t741,t742,t743,t744,t745,t746,t747,t749,t750,t751,t755,t756,t757,t758,t759,t76,t762,t763,t764,t766,t767,t768,t770,t771,t772,t773,t774,t775,t776,t777,t778,t781,t782,t783,t784,t785,t786,t787,t789,t790,t791,t792,t793,t794,t796,t797,t798,t799,t8,t800,t801,t802,t806,t807,t808,t809,t812,t813,t816,t817,t818,t819,t820,t821,t822,t823,t824,t825,t826,t827,t828,t829,t830,t831,t832,t833,t850,t855,t856,t874,t878,t89,t893,t9,t90,t91,t911,t92,t925,t926,t936,t937,t940,t941,t942,t944,t945,t948,t949,t950,t951,t959,t961,t965,t966,t97,t974,t978,t983,t987,t989,t99,t990,t991,t992,t993,t995,t996,t998});
end
function tau_c = ft_6(ct)
dq1 = ct{1};
dq2 = ct{2};
dq3 = ct{3};
dq4 = ct{4};
dq5 = ct{5};
dq6 = ct{6};
t10 = ct{7};
t100 = ct{8};
t1000 = ct{9};
t1002 = ct{10};
t1003 = ct{11};
t1004 = ct{12};
t1005 = ct{13};
t1006 = ct{14};
t101 = ct{15};
t1011 = ct{16};
t1015 = ct{17};
t1018 = ct{18};
t1019 = ct{19};
t1020 = ct{20};
t1021 = ct{21};
t1022 = ct{22};
t1023 = ct{23};
t1024 = ct{24};
t1026 = ct{25};
t1028 = ct{26};
t1033 = ct{27};
t1034 = ct{28};
t1035 = ct{29};
t1036 = ct{30};
t1037 = ct{31};
t1038 = ct{32};
t1040 = ct{33};
t1043 = ct{34};
t1044 = ct{35};
t1045 = ct{36};
t1046 = ct{37};
t1048 = ct{38};
t1049 = ct{39};
t1050 = ct{40};
t1051 = ct{41};
t1053 = ct{42};
t1054 = ct{43};
t1056 = ct{44};
t1057 = ct{45};
t1058 = ct{46};
t1059 = ct{47};
t1060 = ct{48};
t1063 = ct{49};
t1065 = ct{50};
t1067 = ct{51};
t1068 = ct{52};
t107 = ct{53};
t1071 = ct{54};
t1072 = ct{55};
t1074 = ct{56};
t1075 = ct{57};
t1076 = ct{58};
t1077 = ct{59};
t1078 = ct{60};
t1079 = ct{61};
t108 = ct{62};
t1083 = ct{63};
t1084 = ct{64};
t1088 = ct{65};
t1089 = ct{66};
t1093 = ct{67};
t1097 = ct{68};
t1098 = ct{69};
t1099 = ct{70};
t11 = ct{71};
t1103 = ct{72};
t1104 = ct{73};
t1105 = ct{74};
t1108 = ct{75};
t1109 = ct{76};
t1111 = ct{77};
t1115 = ct{78};
t1116 = ct{79};
t1119 = ct{80};
t1120 = ct{81};
t1121 = ct{82};
t1125 = ct{83};
t1127 = ct{84};
t1128 = ct{85};
t1129 = ct{86};
t1130 = ct{87};
t1131 = ct{88};
t1133 = ct{89};
t1135 = ct{90};
t1136 = ct{91};
t1138 = ct{92};
t1139 = ct{93};
t1140 = ct{94};
t1142 = ct{95};
t1144 = ct{96};
t1151 = ct{97};
t1152 = ct{98};
t1153 = ct{99};
t1156 = ct{100};
t1158 = ct{101};
t1159 = ct{102};
t1160 = ct{103};
t1163 = ct{104};
t1164 = ct{105};
t1165 = ct{106};
t1169 = ct{107};
t1172 = ct{108};
t1173 = ct{109};
t1175 = ct{110};
t1190 = ct{111};
t1193 = ct{112};
t1194 = ct{113};
t1195 = ct{114};
t1196 = ct{115};
t12 = ct{116};
t1200 = ct{117};
t1205 = ct{118};
t1207 = ct{119};
t1208 = ct{120};
t1210 = ct{121};
t1211 = ct{122};
t1212 = ct{123};
t1214 = ct{124};
t1217 = ct{125};
t1218 = ct{126};
t1219 = ct{127};
t1220 = ct{128};
t1221 = ct{129};
t1222 = ct{130};
t123 = ct{131};
t1230 = ct{132};
t1235 = ct{133};
t1236 = ct{134};
t1237 = ct{135};
t1238 = ct{136};
t124 = ct{137};
t126 = ct{138};
t1266 = ct{139};
t128 = ct{140};
t1285 = ct{141};
t1286 = ct{142};
t1287 = ct{143};
t1288 = ct{144};
t1289 = ct{145};
t1290 = ct{146};
t1299 = ct{147};
t13 = ct{148};
t130 = ct{149};
t1300 = ct{150};
t1301 = ct{151};
t1302 = ct{152};
t1303 = ct{153};
t1305 = ct{154};
t1307 = ct{155};
t1311 = ct{156};
t1316 = ct{157};
t1317 = ct{158};
t1319 = ct{159};
t1320 = ct{160};
t1322 = ct{161};
t1323 = ct{162};
t1324 = ct{163};
t1328 = ct{164};
t1331 = ct{165};
t1335 = ct{166};
t1336 = ct{167};
t1337 = ct{168};
t1338 = ct{169};
t134 = ct{170};
t1342 = ct{171};
t1343 = ct{172};
t1344 = ct{173};
t1345 = ct{174};
t1348 = ct{175};
t1349 = ct{176};
t1350 = ct{177};
t1351 = ct{178};
t1352 = ct{179};
t1354 = ct{180};
t1360 = ct{181};
t1366 = ct{182};
t1367 = ct{183};
t1368 = ct{184};
t1369 = ct{185};
t1370 = ct{186};
t1371 = ct{187};
t1372 = ct{188};
t1374 = ct{189};
t1375 = ct{190};
t1376 = ct{191};
t1377 = ct{192};
t1378 = ct{193};
t1379 = ct{194};
t1380 = ct{195};
t1385 = ct{196};
t1386 = ct{197};
t1387 = ct{198};
t1388 = ct{199};
t1389 = ct{200};
t139 = ct{201};
t1392 = ct{202};
t1393 = ct{203};
t1394 = ct{204};
t1395 = ct{205};
t1396 = ct{206};
t1397 = ct{207};
t1398 = ct{208};
t1399 = ct{209};
t14 = ct{210};
t140 = ct{211};
t1404 = ct{212};
t1405 = ct{213};
t1406 = ct{214};
t1407 = ct{215};
t1408 = ct{216};
t1409 = ct{217};
t1410 = ct{218};
t1411 = ct{219};
t1412 = ct{220};
t1414 = ct{221};
t1415 = ct{222};
t1416 = ct{223};
t1417 = ct{224};
t1419 = ct{225};
t1420 = ct{226};
t1421 = ct{227};
t1424 = ct{228};
t1425 = ct{229};
t1427 = ct{230};
t1428 = ct{231};
t1429 = ct{232};
t1431 = ct{233};
t1432 = ct{234};
t1433 = ct{235};
t1434 = ct{236};
t1435 = ct{237};
t1436 = ct{238};
t1439 = ct{239};
t1440 = ct{240};
t1441 = ct{241};
t1444 = ct{242};
t1447 = ct{243};
t1448 = ct{244};
t1453 = ct{245};
t1456 = ct{246};
t1457 = ct{247};
t1458 = ct{248};
t1462 = ct{249};
t1464 = ct{250};
t1465 = ct{251};
t1466 = ct{252};
t1467 = ct{253};
t1471 = ct{254};
t1472 = ct{255};
t1476 = ct{256};
t1477 = ct{257};
t1478 = ct{258};
t1481 = ct{259};
t1485 = ct{260};
t1487 = ct{261};
t1488 = ct{262};
t1489 = ct{263};
t1490 = ct{264};
t1492 = ct{265};
t1493 = ct{266};
t1494 = ct{267};
t1495 = ct{268};
t1498 = ct{269};
t15 = ct{270};
t1500 = ct{271};
t1501 = ct{272};
t1502 = ct{273};
t1503 = ct{274};
t1504 = ct{275};
t1505 = ct{276};
t1506 = ct{277};
t1507 = ct{278};
t1508 = ct{279};
t151 = ct{280};
t1510 = ct{281};
t1512 = ct{282};
t1513 = ct{283};
t1514 = ct{284};
t1515 = ct{285};
t1516 = ct{286};
t1517 = ct{287};
t1519 = ct{288};
t1522 = ct{289};
t1526 = ct{290};
t1527 = ct{291};
t1529 = ct{292};
t1531 = ct{293};
t1534 = ct{294};
t1537 = ct{295};
t1538 = ct{296};
t1539 = ct{297};
t1540 = ct{298};
t1543 = ct{299};
t1544 = ct{300};
t1545 = ct{301};
t1546 = ct{302};
t1547 = ct{303};
t1548 = ct{304};
t1549 = ct{305};
t1550 = ct{306};
t1551 = ct{307};
t1553 = ct{308};
t1554 = ct{309};
t1555 = ct{310};
t1556 = ct{311};
t1557 = ct{312};
t1558 = ct{313};
t1559 = ct{314};
t1564 = ct{315};
t1565 = ct{316};
t1574 = ct{317};
t1575 = ct{318};
t1576 = ct{319};
t1577 = ct{320};
t1578 = ct{321};
t1579 = ct{322};
t1581 = ct{323};
t1582 = ct{324};
t1584 = ct{325};
t1585 = ct{326};
t1586 = ct{327};
t1587 = ct{328};
t1591 = ct{329};
t1592 = ct{330};
t1593 = ct{331};
t1595 = ct{332};
t1596 = ct{333};
t1598 = ct{334};
t1599 = ct{335};
t16 = ct{336};
t1600 = ct{337};
t1601 = ct{338};
t1602 = ct{339};
t1603 = ct{340};
t1604 = ct{341};
t1605 = ct{342};
t1606 = ct{343};
t1607 = ct{344};
t1608 = ct{345};
t1609 = ct{346};
t1610 = ct{347};
t1612 = ct{348};
t1613 = ct{349};
t1614 = ct{350};
t1615 = ct{351};
t1616 = ct{352};
t1619 = ct{353};
t1621 = ct{354};
t1625 = ct{355};
t1626 = ct{356};
t1627 = ct{357};
t1628 = ct{358};
t1629 = ct{359};
t1631 = ct{360};
t1632 = ct{361};
t1634 = ct{362};
t1637 = ct{363};
t1639 = ct{364};
t1640 = ct{365};
t1641 = ct{366};
t1642 = ct{367};
t1644 = ct{368};
t1645 = ct{369};
t1646 = ct{370};
t1647 = ct{371};
t1648 = ct{372};
t1649 = ct{373};
t1655 = ct{374};
t1656 = ct{375};
t1657 = ct{376};
t1658 = ct{377};
t1659 = ct{378};
t1660 = ct{379};
t1661 = ct{380};
t1662 = ct{381};
t1663 = ct{382};
t1666 = ct{383};
t1667 = ct{384};
t1670 = ct{385};
t1675 = ct{386};
t1677 = ct{387};
t1679 = ct{388};
t1680 = ct{389};
t1683 = ct{390};
t1684 = ct{391};
t1685 = ct{392};
t1686 = ct{393};
t1687 = ct{394};
t1690 = ct{395};
t1692 = ct{396};
t1696 = ct{397};
t1697 = ct{398};
t1698 = ct{399};
t1699 = ct{400};
t17 = ct{401};
t1700 = ct{402};
t1701 = ct{403};
t1703 = ct{404};
t1704 = ct{405};
t1705 = ct{406};
t1706 = ct{407};
t1707 = ct{408};
t1708 = ct{409};
t1709 = ct{410};
t1710 = ct{411};
t1711 = ct{412};
t1712 = ct{413};
t1713 = ct{414};
t1714 = ct{415};
t1715 = ct{416};
t1717 = ct{417};
t1718 = ct{418};
t1719 = ct{419};
t1720 = ct{420};
t1721 = ct{421};
t1722 = ct{422};
t1723 = ct{423};
t1724 = ct{424};
t1725 = ct{425};
t1726 = ct{426};
t1727 = ct{427};
t1728 = ct{428};
t1729 = ct{429};
t1730 = ct{430};
t1731 = ct{431};
t1732 = ct{432};
t1733 = ct{433};
t1734 = ct{434};
t1735 = ct{435};
t1736 = ct{436};
t1737 = ct{437};
t1738 = ct{438};
t1739 = ct{439};
t1741 = ct{440};
t1742 = ct{441};
t1743 = ct{442};
t1744 = ct{443};
t1745 = ct{444};
t1746 = ct{445};
t1747 = ct{446};
t1748 = ct{447};
t1750 = ct{448};
t1752 = ct{449};
t1753 = ct{450};
t1754 = ct{451};
t1755 = ct{452};
t1758 = ct{453};
t1759 = ct{454};
t1760 = ct{455};
t1761 = ct{456};
t1762 = ct{457};
t1763 = ct{458};
t1764 = ct{459};
t1767 = ct{460};
t1768 = ct{461};
t1769 = ct{462};
t1770 = ct{463};
t1774 = ct{464};
t1775 = ct{465};
t1776 = ct{466};
t1778 = ct{467};
t1779 = ct{468};
t1781 = ct{469};
t1783 = ct{470};
t1784 = ct{471};
t1785 = ct{472};
t1786 = ct{473};
t1787 = ct{474};
t1788 = ct{475};
t1789 = ct{476};
t1790 = ct{477};
t1791 = ct{478};
t1792 = ct{479};
t18 = ct{480};
t1801 = ct{481};
t1803 = ct{482};
t1808 = ct{483};
t1809 = ct{484};
t1811 = ct{485};
t1812 = ct{486};
t1816 = ct{487};
t1818 = ct{488};
t1819 = ct{489};
t182 = ct{490};
t1820 = ct{491};
t1821 = ct{492};
t1822 = ct{493};
t1823 = ct{494};
t1824 = ct{495};
t1825 = ct{496};
t1830 = ct{497};
t1831 = ct{498};
t1832 = ct{499};
t1833 = ct{500};
t1837 = ct{501};
t1838 = ct{502};
t1839 = ct{503};
t1841 = ct{504};
t1844 = ct{505};
t1845 = ct{506};
t1846 = ct{507};
t1847 = ct{508};
t1848 = ct{509};
t1849 = ct{510};
t1850 = ct{511};
t1851 = ct{512};
t1852 = ct{513};
t1853 = ct{514};
t1854 = ct{515};
t1855 = ct{516};
t1856 = ct{517};
t1857 = ct{518};
t1858 = ct{519};
t1859 = ct{520};
t1860 = ct{521};
t1861 = ct{522};
t1864 = ct{523};
t1865 = ct{524};
t1867 = ct{525};
t1868 = ct{526};
t1869 = ct{527};
t1870 = ct{528};
t1874 = ct{529};
t1875 = ct{530};
t1876 = ct{531};
t1879 = ct{532};
t188 = ct{533};
t1880 = ct{534};
t1881 = ct{535};
t1882 = ct{536};
t1883 = ct{537};
t1884 = ct{538};
t1886 = ct{539};
t1887 = ct{540};
t1888 = ct{541};
t1889 = ct{542};
t189 = ct{543};
t1890 = ct{544};
t1891 = ct{545};
t1893 = ct{546};
t1896 = ct{547};
t19 = ct{548};
t1900 = ct{549};
t1901 = ct{550};
t1902 = ct{551};
t1903 = ct{552};
t1904 = ct{553};
t1905 = ct{554};
t1906 = ct{555};
t1909 = ct{556};
t1910 = ct{557};
t1911 = ct{558};
t1912 = ct{559};
t1913 = ct{560};
t1918 = ct{561};
t1923 = ct{562};
t1924 = ct{563};
t1925 = ct{564};
t1926 = ct{565};
t1927 = ct{566};
t1929 = ct{567};
t1930 = ct{568};
t1931 = ct{569};
t1933 = ct{570};
t1934 = ct{571};
t1935 = ct{572};
t1936 = ct{573};
t1937 = ct{574};
t1939 = ct{575};
t1940 = ct{576};
t1941 = ct{577};
t1943 = ct{578};
t1945 = ct{579};
t1946 = ct{580};
t1948 = ct{581};
t1951 = ct{582};
t1952 = ct{583};
t1953 = ct{584};
t1954 = ct{585};
t1955 = ct{586};
t1956 = ct{587};
t1957 = ct{588};
t1958 = ct{589};
t1959 = ct{590};
t1961 = ct{591};
t1962 = ct{592};
t1963 = ct{593};
t1964 = ct{594};
t1966 = ct{595};
t1967 = ct{596};
t1969 = ct{597};
t1971 = ct{598};
t1972 = ct{599};
t1973 = ct{600};
t1978 = ct{601};
t1979 = ct{602};
t1980 = ct{603};
t1981 = ct{604};
t1983 = ct{605};
t1984 = ct{606};
t1985 = ct{607};
t1988 = ct{608};
t1990 = ct{609};
t1991 = ct{610};
t1992 = ct{611};
t1993 = ct{612};
t1994 = ct{613};
t1997 = ct{614};
t1998 = ct{615};
t1999 = ct{616};
t20 = ct{617};
t2001 = ct{618};
t2002 = ct{619};
t2003 = ct{620};
t2004 = ct{621};
t2005 = ct{622};
t2006 = ct{623};
t2007 = ct{624};
t2008 = ct{625};
t2009 = ct{626};
t201 = ct{627};
t2010 = ct{628};
t2013 = ct{629};
t2014 = ct{630};
t2015 = ct{631};
t2016 = ct{632};
t2017 = ct{633};
t202 = ct{634};
t2023 = ct{635};
t2024 = ct{636};
t2027 = ct{637};
t2028 = ct{638};
t2029 = ct{639};
t203 = ct{640};
t2030 = ct{641};
t2031 = ct{642};
t2032 = ct{643};
t2033 = ct{644};
t2034 = ct{645};
t2035 = ct{646};
t2036 = ct{647};
t2037 = ct{648};
t2039 = ct{649};
t2040 = ct{650};
t2041 = ct{651};
t2042 = ct{652};
t2043 = ct{653};
t2044 = ct{654};
t2045 = ct{655};
t2049 = ct{656};
t2050 = ct{657};
t2051 = ct{658};
t2052 = ct{659};
t2053 = ct{660};
t2054 = ct{661};
t2057 = ct{662};
t2058 = ct{663};
t2059 = ct{664};
t2060 = ct{665};
t2061 = ct{666};
t2062 = ct{667};
t2063 = ct{668};
t2064 = ct{669};
t2065 = ct{670};
t2066 = ct{671};
t2067 = ct{672};
t2068 = ct{673};
t2069 = ct{674};
t2070 = ct{675};
t2071 = ct{676};
t2072 = ct{677};
t2073 = ct{678};
t2074 = ct{679};
t2075 = ct{680};
t2079 = ct{681};
t2081 = ct{682};
t2082 = ct{683};
t2083 = ct{684};
t2084 = ct{685};
t2085 = ct{686};
t2086 = ct{687};
t2087 = ct{688};
t2089 = ct{689};
t2090 = ct{690};
t2091 = ct{691};
t2093 = ct{692};
t2094 = ct{693};
t2095 = ct{694};
t2098 = ct{695};
t2099 = ct{696};
t21 = ct{697};
t2100 = ct{698};
t2101 = ct{699};
t2102 = ct{700};
t2103 = ct{701};
t2104 = ct{702};
t2105 = ct{703};
t2106 = ct{704};
t2107 = ct{705};
t2108 = ct{706};
t2109 = ct{707};
t2110 = ct{708};
t2111 = ct{709};
t2112 = ct{710};
t2117 = ct{711};
t2120 = ct{712};
t2122 = ct{713};
t2123 = ct{714};
t2125 = ct{715};
t2130 = ct{716};
t2132 = ct{717};
t2133 = ct{718};
t2134 = ct{719};
t2135 = ct{720};
t2137 = ct{721};
t2138 = ct{722};
t2139 = ct{723};
t2140 = ct{724};
t2141 = ct{725};
t2142 = ct{726};
t2143 = ct{727};
t2145 = ct{728};
t2146 = ct{729};
t2147 = ct{730};
t2149 = ct{731};
t2150 = ct{732};
t2151 = ct{733};
t2152 = ct{734};
t2153 = ct{735};
t2154 = ct{736};
t2155 = ct{737};
t2156 = ct{738};
t2157 = ct{739};
t2159 = ct{740};
t216 = ct{741};
t2160 = ct{742};
t2161 = ct{743};
t2162 = ct{744};
t2163 = ct{745};
t2164 = ct{746};
t2165 = ct{747};
t2166 = ct{748};
t2167 = ct{749};
t2168 = ct{750};
t2169 = ct{751};
t2170 = ct{752};
t2171 = ct{753};
t2172 = ct{754};
t2173 = ct{755};
t2174 = ct{756};
t2176 = ct{757};
t2177 = ct{758};
t2178 = ct{759};
t2179 = ct{760};
t2180 = ct{761};
t2181 = ct{762};
t2182 = ct{763};
t2183 = ct{764};
t2184 = ct{765};
t2187 = ct{766};
t2190 = ct{767};
t2191 = ct{768};
t2192 = ct{769};
t2193 = ct{770};
t2194 = ct{771};
t2195 = ct{772};
t2198 = ct{773};
t2199 = ct{774};
t22 = ct{775};
t2200 = ct{776};
t2201 = ct{777};
t2202 = ct{778};
t2203 = ct{779};
t2207 = ct{780};
t2208 = ct{781};
t2209 = ct{782};
t2210 = ct{783};
t2211 = ct{784};
t2215 = ct{785};
t2216 = ct{786};
t2217 = ct{787};
t2218 = ct{788};
t2219 = ct{789};
t2222 = ct{790};
t2223 = ct{791};
t2224 = ct{792};
t2227 = ct{793};
t2229 = ct{794};
t2230 = ct{795};
t2232 = ct{796};
t2233 = ct{797};
t2234 = ct{798};
t2237 = ct{799};
t2238 = ct{800};
t2239 = ct{801};
t2240 = ct{802};
t2241 = ct{803};
t2242 = ct{804};
t2243 = ct{805};
t2248 = ct{806};
t2249 = ct{807};
t2254 = ct{808};
t2256 = ct{809};
t2257 = ct{810};
t2258 = ct{811};
t2259 = ct{812};
t2260 = ct{813};
t2261 = ct{814};
t2262 = ct{815};
t2263 = ct{816};
t2264 = ct{817};
t2265 = ct{818};
t2266 = ct{819};
t2267 = ct{820};
t2268 = ct{821};
t2269 = ct{822};
t2270 = ct{823};
t2271 = ct{824};
t2272 = ct{825};
t2273 = ct{826};
t2274 = ct{827};
t2275 = ct{828};
t2276 = ct{829};
t2277 = ct{830};
t2278 = ct{831};
t2279 = ct{832};
t2280 = ct{833};
t2281 = ct{834};
t2282 = ct{835};
t2283 = ct{836};
t2284 = ct{837};
t2285 = ct{838};
t2286 = ct{839};
t2287 = ct{840};
t2288 = ct{841};
t2289 = ct{842};
t2290 = ct{843};
t2291 = ct{844};
t2292 = ct{845};
t2293 = ct{846};
t2294 = ct{847};
t2295 = ct{848};
t2296 = ct{849};
t2297 = ct{850};
t2298 = ct{851};
t2299 = ct{852};
t230 = ct{853};
t2300 = ct{854};
t2301 = ct{855};
t2302 = ct{856};
t2303 = ct{857};
t2304 = ct{858};
t2305 = ct{859};
t2306 = ct{860};
t2307 = ct{861};
t2308 = ct{862};
t2309 = ct{863};
t231 = ct{864};
t2310 = ct{865};
t2311 = ct{866};
t2312 = ct{867};
t2313 = ct{868};
t2317 = ct{869};
t2320 = ct{870};
t2322 = ct{871};
t2323 = ct{872};
t2324 = ct{873};
t2325 = ct{874};
t2326 = ct{875};
t2327 = ct{876};
t2328 = ct{877};
t2329 = ct{878};
t2335 = ct{879};
t2336 = ct{880};
t2337 = ct{881};
t2338 = ct{882};
t2339 = ct{883};
t2340 = ct{884};
t2341 = ct{885};
t2342 = ct{886};
t2343 = ct{887};
t2344 = ct{888};
t2345 = ct{889};
t2346 = ct{890};
t2350 = ct{891};
t2351 = ct{892};
t2352 = ct{893};
t2353 = ct{894};
t2354 = ct{895};
t2355 = ct{896};
t2356 = ct{897};
t2357 = ct{898};
t2358 = ct{899};
t2359 = ct{900};
t236 = ct{901};
t2360 = ct{902};
t2361 = ct{903};
t2362 = ct{904};
t2363 = ct{905};
t2364 = ct{906};
t2365 = ct{907};
t2366 = ct{908};
t2367 = ct{909};
t2368 = ct{910};
t2369 = ct{911};
t237 = ct{912};
t2370 = ct{913};
t2371 = ct{914};
t2373 = ct{915};
t2374 = ct{916};
t2375 = ct{917};
t2376 = ct{918};
t2377 = ct{919};
t2378 = ct{920};
t2379 = ct{921};
t238 = ct{922};
t2380 = ct{923};
t2381 = ct{924};
t2382 = ct{925};
t2384 = ct{926};
t2385 = ct{927};
t2386 = ct{928};
t2387 = ct{929};
t2388 = ct{930};
t2389 = ct{931};
t239 = ct{932};
t2390 = ct{933};
